simulink model "Supplementary"  (R2021a)
(part 36 of 44)

C12b = 0.125*a4*lc4_1*m4*theta_dot_1*sin(2.0*theta3 - 2.0*theta2 + 2.0*theta4) - 0.125*a4*lc4_1*m4*theta_dot_1*sin(2.0*theta2 + 2.0*theta3 + 2.0*theta4) + 0.5*lc5_1*lc5_3*m5*theta_dot_2*sin(theta3 - theta2 + theta4 + theta5) + 0.25*a1*a3*m3*theta_dot_1*sin(theta2 - theta3) + 0.5*a1*a3*m4*theta_dot_1*sin(theta2 - theta3) + 0.5*a1*a3*m5*theta_dot_1*sin(theta2 - theta3) + 0.25*a2*a3*m3*theta_dot_2*sin(theta2 - theta3) + 0.5*a2*a3*m4*theta_dot_2*sin(theta2 - theta3) + 0.5*a2*a3*m5*theta_dot_2*sin(theta2 - theta3) - 0.25*a4*a5*m5*theta_dot_3*sin(theta2 - theta5) - 0.25*a4*a5*m5*theta_dot_4*sin(theta2 - theta5) - 0.125*a4*a5*m5*theta_dot_5*sin(theta2 - theta5) - 0.125*a5*lc5_2*m5*theta_dot_1*cos(2.0*theta3 - 2.0*theta2 + 2.0*theta4 + 2.0*theta5) + 0.125*a5*lc5_2*m5*theta_dot_1*cos(2.0*theta2 + 2.0*theta3 + 2.0*theta4 + 2.0*theta5) - 0.25*a3*a4*m4*theta_dot_2*cos(2.0*theta3 - theta2 + theta4) + 0.25*a3*a4*m4*theta_dot_3*cos(2.0*theta3 - theta2 + theta4) - 0.5*a3*a4*m5*theta_dot_2*cos(2.0*theta3 - theta2 + theta4) + 0.125*a3*a4*m4*theta_dot_4*cos(2.0*theta3 - theta2 + theta4) + 0.5*a3*a4*m5*theta_dot_3*cos(2.0*theta3 - theta2 + theta4) + 0.25*a3*a4*m5*theta_dot_4*cos(2.0*theta3 - theta2 + theta4) + 0.5*lc3_1*lc3_3*m3*theta_dot_2*cos(theta2 - theta3) + 0.5*a1*lc3_1*m3*theta_dot_1*sin(theta2 - theta3) + 0.5*a2*lc3_1*m3*theta_dot_2*sin(theta2 - theta3) + 0.5*a3*lc4_2*m4*theta_dot_3*sin(theta2 - theta4) + 0.25*a3*lc4_2*m4*theta_dot_4*sin(theta2 - theta4) - 0.5*a4*lc5_1*m5*theta_dot_3*sin(theta2 - theta5) - 0.5*a4*lc5_1*m5*theta_dot_4*sin(theta2 - theta5) - 0.25*a4*lc5_1*m5*theta_dot_5*sin(theta2 - theta5) - 0.25*lc5_1*lc5_2*m5*theta_dot_1*cos(2.0*theta3 - 2.0*theta2 + 2.0*theta4 + 2.0*theta5) + 0.25*lc5_1*lc5_2*m5*theta_dot_1*cos(2.0*theta2 + 2.0*theta3 + 2.0*theta4 + 2.0*theta5) - 0.5*a3*lc4_1*m4*theta_dot_2*cos(2.0*theta3 - theta2 + theta4) + 0.5*a3*lc4_1*m4*theta_dot_3*cos(2.0*theta3 - theta2 + theta4) + 0.25*a3*lc4_1*m4*theta_dot_4*cos(2.0*theta3 - theta2 + theta4) - 0.5*a1*lc4_2*m4*theta_dot_1*cos(theta2 + theta3 + theta4) + 0.5*a2*lc4_2*m4*theta_dot_2*cos(theta2 + theta3 + theta4) + 0.25*a4*lc4_3*m4*theta_dot_2*cos(theta2 + theta3 + theta4) + 0.5*a4*lc5_3*m5*theta_dot_2*cos(theta2 + theta3 + theta4) + 0.5*a3*lc5_2*m5*theta_dot_3*cos(theta2 + theta4 + theta5) + 0.25*a3*lc5_2*m5*theta_dot_4*cos(theta2 + theta4 + theta5) + 0.25*a3*lc5_2*m5*theta_dot_5*cos(theta2 + theta4 + theta5) - 0.125*a5*lc5_1*m5*theta_dot_1*sin(2.0*theta3 - 2.0*theta2 + 2.0*theta4 + 2.0*theta5) + 0.125*a5*lc5_1*m5*theta_dot_1*sin(2.0*theta2 + 2.0*theta3 + 2.0*theta4 + 2.0*theta5) - 0.25*a1*a4*m4*theta_dot_1*sin(theta2 + theta3 + theta4) - 0.5*a1*a4*m5*theta_dot_1*sin(theta2 + theta3 + theta4) + 0.25*a2*a4*m4*theta_dot_2*sin(theta2 + theta3 + theta4) + 0.5*a2*a4*m5*theta_dot_2*sin(theta2 + theta3 + theta4) + 0.25*a3*a5*m5*theta_dot_3*sin(theta2 + theta4 + theta5) + 0.125*a3*a5*m5*theta_dot_4*sin(theta2 + theta4 + theta5) + 0.125*a3*a5*m5*theta_dot_5*sin(theta2 + theta4 + theta5) + 0.5*lc3_2*lc3_3*m3*theta_dot_2*sin(theta2 - theta3) + 0.5*lc4_1*lc4_3*m4*theta_dot_2*cos(theta2 + theta3 + theta4) + 0.5*a3*lc4_2*m4*theta_dot_2*sin(2.0*theta3 - theta2 + theta4) - 0.5*a3*lc4_2*m4*theta_dot_3*sin(2.0*theta3 - theta2 + theta4) - 0.25*a3*lc4_2*m4*theta_dot_4*sin(2.0*theta3 - theta2 + theta4) - 0.5*a1*lc4_1*m4*theta_dot_1*sin(theta2 + theta3 + theta4) + 0.5*a2*lc4_1*m4*theta_dot_2*sin(theta2 + theta3 + theta4) + 0.5*a3*lc5_1*m5*theta_dot_3*sin(theta2 + theta4 + theta5) + 0.25*a3*lc5_1*m5*theta_dot_4*sin(theta2 + theta4 + theta5) + 0.25*a3*lc5_1*m5*theta_dot_5*sin(theta2 + theta4 + theta5) - 0.5*a4*lc5_2*m5*theta_dot_2*cos(2.0*theta3 - theta2 + 2.0*theta4 + theta5) + 0.5*a4*lc5_2*m5*theta_dot_3*cos(2.0*theta3 - theta2 + 2.0*theta4 + theta5) + 0.5*a4*lc5_2*m5*theta_dot_4*cos(2.0*theta3 - theta2 + 2.0*theta4 + theta5) + 0.25*a4*lc5_2*m5*theta_dot_5*cos(2.0*theta3 - theta2 + 2.0*theta4 + theta5) - 0.5*a2*lc5_2*m5*theta_dot_1*cos(theta3 - 2.0*theta2 + theta4 + theta5) + 0.5*a2*lc5_2*m5*theta_dot_1*cos(2.0*theta2 + theta3 + theta4 + theta5) + 0.5*a3*lc5_2*m5*theta_dot_2*cos(theta2 + 2.0*theta3 + theta4 + theta5) + 0.5*a3*lc5_2*m5*theta_dot_3*cos(theta2 + 2.0*theta3 + theta4 + theta5) + 0.25*a3*lc5_2*m5*theta_dot_4*cos(theta2 + 2.0*theta3 + theta4 + theta5) + 0.25*a5*lc5_3*m5*theta_dot_1*cos(theta3 - 2.0*theta2 + theta4 + theta5) + 0.25*a5*lc5_3*m5*theta_dot_1*cos(2.0*theta2 + theta3 + theta4 + theta5) + 0.25*a3*lc5_2*m5*theta_dot_5*cos(theta2 + 2.0*theta3 + theta4 + theta5) - 0.25*a4*a5*m5*theta_dot_2*sin(2.0*theta3 - theta2 + 2.0*theta4 + theta5) + 0.25*a4*a5*m5*theta_dot_3*sin(2.0*theta3 - theta2 + 2.0*theta4 + theta5) + 0.25*a4*a5*m5*theta_dot_4*sin(2.0*theta3 - theta2 + 2.0*theta4 + theta5) + 0.125*a4*a5*m5*theta_dot_5*sin(2.0*theta3 - theta2 + 2.0*theta4 + theta5) - 0.25*a2*a5*m5*theta_dot_1*sin(theta3 - 2.0*theta2 + theta4 + theta5) + 0.25*a2*a5*m5*theta_dot_1*sin(2.0*theta2 + theta3 + theta4 + theta5) + 0.25*a3*a5*m5*theta_dot_2*sin(theta2 + 2.0*theta3 + theta4 + theta5) + 0.25*a3*a5*m5*theta_dot_3*sin(theta2 + 2.0*theta3 + theta4 + theta5) + 0.125*a3*a5*m5*theta_dot_4*sin(theta2 + 2.0*theta3 + theta4 + theta5) + 0.125*a3*a5*m5*theta_dot_5*sin(theta2 + 2.0*theta3 + theta4 + theta5) - 0.5*lc4_2*lc4_3*m4*theta_dot_2*sin(theta2 + theta3 + theta4) + 0.5*lc5_1*lc5_3*m5*theta_dot_1*cos(theta3 - 2.0*theta2 + theta4 + theta5) + 0.5*lc5_1*lc5_3*m5*theta_dot_1*cos(2.0*theta2 + theta3 + theta4 + theta5) + 0.25*a2*a3*m3*theta_dot_1*cos(2.0*theta2 + theta3) + 0.5*a2*a3*m4*theta_dot_1*cos(2.0*theta2 + theta3) + 0.5*a2*a3*m5*theta_dot_1*cos(2.0*theta2 + theta3) - 0.125*a4*a5*m5*theta_dot_1*cos(2.0*theta2 + theta5) - 0.5*a4*lc5_1*m5*theta_dot_2*sin(2.0*theta3 - theta2 + 2.0*theta4 + theta5) + 0.5*a4*lc5_1*m5*theta_dot_3*sin(2.0*theta3 - theta2 + 2.0*theta4 + theta5) + 0.5*a4*lc5_1*m5*theta_dot_4*sin(2.0*theta3 - theta2 + 2.0*theta4 + theta5) + 0.25*a4*lc5_1*m5*theta_dot_5*sin(2.0*theta3 - theta2 + 2.0*theta4 + theta5) - 0.5*a2*lc5_1*m5*theta_dot_1*sin(theta3 - 2.0*theta2 + theta4 + theta5) + 0.5*a2*lc5_1*m5*theta_dot_1*sin(2.0*theta2 + theta3 + theta4 + theta5) + 0.5*a3*lc5_1*m5*theta_dot_2*sin(theta2 + 2.0*theta3 + theta4 + theta5) + 0.5*a3*lc5_1*m5*theta_dot_3*sin(theta2 + 2.0*theta3 + theta4 + theta5) + 0.25*a3*lc5_1*m5*theta_dot_4*sin(theta2 + 2.0*theta3 + theta4 + theta5) + 0.25*a3*lc5_1*m5*theta_dot_5*sin(theta2 + 2.0*theta3 + theta4 + theta5) + 0.5*a2*lc3_1*m3*theta_dot_1*cos(2.0*theta2 + theta3) - 0.25*a3*lc3_1*m3*theta_dot_2*cos(theta2 - 2.0*theta3) + 0.25*a3*lc3_1*m3*theta_dot_2*cos(theta2 + 2.0*theta3) + 0.25*a3*lc3_1*m3*theta_dot_3*cos(theta2 - 2.0*theta3) + 0.25*a3*lc3_1*m3*theta_dot_3*cos(theta2 + 2.0*theta3) + 0.25*a3*lc4_2*m4*theta_dot_1*cos(2.0*theta2 + theta4) - 0.25*a4*lc5_1*m5*theta_dot_1*cos(2.0*theta2 + theta5) - 0.5*lc5_2*lc5_3*m5*theta_dot_1*sin(theta3 - 2.0*theta2 + theta4 + theta5) - 0.5*lc5_2*lc5_3*m5*theta_dot_1*sin(2.0*theta2 + theta3 + theta4 + theta5) + 0.125*a3*a4*m4*theta_dot_1*sin(2.0*theta2 + theta4) + 0.25*a3*a4*m5*theta_dot_1*sin(2.0*theta2 + theta4) - 0.5*lc3_2*lc3_3*m3*theta_dot_1*cos(2.0*theta2 + theta3) - 0.5*a2*lc3_2*m3*theta_dot_1*sin(2.0*theta2 + theta3) - 0.25*a3*lc3_2*m3*theta_dot_2*sin(theta2 - 2.0*theta3) - 0.25*a3*lc3_2*m3*theta_dot_2*sin(theta2 + 2.0*theta3) - 0.25*a3*lc3_3*m3*theta_dot_1*sin(2.0*theta2 + theta3) + 0.25*a3*lc3_2*m3*theta_dot_3*sin(theta2 - 2.0*theta3) - 0.25*a3*lc3_2*m3*theta_dot_3*sin(theta2 + 2.0*theta3) + 0.25*a3*lc4_1*m4*theta_dot_1*sin(2.0*theta2 + theta4) - 0.5*a3*lc4_3*m4*theta_dot_1*sin(2.0*theta2 + theta3) - 0.5*a3*lc5_3*m5*theta_dot_1*sin(2.0*theta2 + theta3) + 0.25*a4*lc5_2*m5*theta_dot_1*sin(2.0*theta2 + theta5) + 0.25*a3*lc4_2*m4*theta_dot_1*cos(2.0*theta3 - 2.0*theta2 + theta4) - 0.25*a3*lc4_2*m4*theta_dot_1*cos(2.0*theta2 + 2.0*theta3 + theta4) + 0.25*a4*lc4_1*m4*theta_dot_2*cos(theta2 + 2.0*theta3 + 2.0*theta4) + 0.25*a4*lc4_1*m4*theta_dot_3*cos(theta2 + 2.0*theta3 + 2.0*theta4) + 0.25*a4*lc4_1*m4*theta_dot_4*cos(theta2 + 2.0*theta3 + 2.0*theta4) + 0.125*a3*a4*m4*theta_dot_1*sin(2.0*theta3 - 2.0*theta2 + theta4) - 0.125*a3*a4*m4*theta_dot_1*sin(2.0*theta2 + 2.0*theta3 + theta4) + 0.25*a3*a4*m5*theta_dot_1*sin(2.0*theta3 - 2.0*theta2 + theta4) - 0.25*a3*a4*m5*theta_dot_1*sin(2.0*theta2 + 2.0*theta3 + theta4) - 0.5*lc3_1*lc3_2*m3*theta_dot_2*sin(theta2 - 2.0*theta3) - 0.5*lc3_1*lc3_2*m3*theta_dot_2*sin(theta2 + 2.0*theta3) - 0.5*lc3_1*lc3_3*m3*theta_dot_1*sin(2.0*theta2 + theta3) + 0.5*lc3_1*lc3_2*m3*theta_dot_3*sin(theta2 - 2.0*theta3) - 0.5*lc3_1*lc3_2*m3*theta_dot_3*sin(theta2 + 2.0*theta3) - 0.125*a4*a5*m5*theta_dot_1*cos(2.0*theta3 - 2.0*theta2 + 2.0*theta4 + theta5) + 0.125*a4*a5*m5*theta_dot_1*cos(2.0*theta2 + 2.0*theta3 + 2.0*theta4 + theta5) + 0.25*a3*lc4_1*m4*theta_dot_1*sin(2.0*theta3 - 2.0*theta2 + theta4) - 0.25*a3*lc4_1*m4*theta_dot_1*sin(2.0*theta2 + 2.0*theta3 + theta4) - 0.25*a4*lc4_2*m4*theta_dot_2*sin(theta2 + 2.0*theta3 + 2.0*theta4) - 0.25*a4*lc4_2*m4*theta_dot_3*sin(theta2 + 2.0*theta3 + 2.0*theta4) - 0.25*a4*lc4_2*m4*theta_dot_4*sin(theta2 + 2.0*theta3 + 2.0*theta4) - 0.25*a4*lc5_1*m5*theta_dot_1*cos(2.0*theta3 - 2.0*theta2 + 2.0*theta4 + theta5) + 0.25*a4*lc5_1*m5*theta_dot_1*cos(2.0*theta2 + 2.0*theta3 + 2.0*theta4 + theta5) - 0.25*a5*lc5_1*m5*theta_dot_2*cos(theta2 + 2.0*theta3 + 2.0*theta4 + 2.0*theta5) - 0.25*a5*lc5_1*m5*theta_dot_3*cos(theta2 + 2.0*theta3 + 2.0*theta4 + 2.0*theta5) - 0.25*a5*lc5_1*m5*theta_dot_4*cos(theta2 + 2.0*theta3 + 2.0*theta4 + 2.0*theta5) - 0.25*a5*lc5_1*m5*theta_dot_5*cos(theta2 + 2.0*theta3 + 2.0*theta4 + 2.0*theta5) + 0.5*a2*lc2_3*m2*theta_dot_1*cos(2.0*theta2) + 1.0*a2*lc3_3*m3*theta_dot_1*cos(2.0*theta2) + 1.0*a2*lc4_3*m4*theta_dot_1*cos(2.0*theta2) + 1.0*a2*lc5_3*m5*theta_dot_1*cos(2.0*theta2) - 0.5*lc4_1*lc4_2*m4*theta_dot_2*sin(theta2 + 2.0*theta3 + 2.0*theta4) - 0.5*lc4_1*lc4_2*m4*theta_dot_3*sin(theta2 + 2.0*theta3 + 2.0*theta4) - 0.5*lc4_1*lc4_2*m4*theta_dot_4*sin(theta2 + 2.0*theta3 + 2.0*theta4) - 0.5*a1*lc4_2*m4*theta_dot_1*cos(theta3 - theta2 + theta4) - 0.5*a2*lc4_2*m4*theta_dot_2*cos(theta3 - theta2 + theta4) + 0.25*a4*lc4_3*m4*theta_dot_2*cos(theta3 - theta2 + theta4) + 0.5*a4*lc5_3*m5*theta_dot_2*cos(theta3 - theta2 + theta4) + 0.5*a3*lc5_2*m5*theta_dot_3*cos(theta4 - theta2 + theta5) + 0.25*a3*lc5_2*m5*theta_dot_4*cos(theta4 - theta2 + theta5) + 0.25*a3*lc5_2*m5*theta_dot_5*cos(theta4 - theta2 + theta5) + 1.0*lc2_1*lc2_3*m2*theta_dot_1*cos(2.0*theta2) + 0.25*a4*lc5_2*m5*theta_dot_1*sin(2.0*theta3 - 2.0*theta2 + 2.0*theta4 + theta5) - 0.25*a4*lc5_2*m5*theta_dot_1*sin(2.0*theta2 + 2.0*theta3 + 2.0*theta4 + theta5) + 0.25*a5*lc5_2*m5*theta_dot_2*sin(theta2 + 2.0*theta3 + 2.0*theta4 + 2.0*theta5) + 0.25*a5*lc5_2*m5*theta_dot_3*sin(theta2 + 2.0*theta3 + 2.0*theta4 + 2.0*theta5) + 0.25*a5*lc5_2*m5*theta_dot_4*sin(theta2 + 2.0*theta3 + 2.0*theta4 + 2.0*theta5) + 0.25*a5*lc5_2*m5*theta_dot_5*sin(theta2 + 2.0*theta3 + 2.0*theta4 + 2.0*theta5) - 0.25*a1*a4*m4*theta_dot_1*sin(theta3 - theta2 + theta4) - 0.5*a1*a4*m5*theta_dot_1*sin(theta3 - theta2 + theta4) - 0.25*a2*a4*m4*theta_dot_2*sin(theta3 - theta2 + theta4) - 0.5*a2*a4*m5*theta_dot_2*sin(theta3 - theta2 + theta4) + 0.25*a3*a5*m5*theta_dot_3*sin(theta4 - theta2 + theta5) + 0.125*a3*a5*m5*theta_dot_4*sin(theta4 - theta2 + theta5) + 0.125*a3*a5*m5*theta_dot_5*sin(theta4 - theta2 + theta5) + 0.5*a2*lc2_1*m2*theta_dot_1*sin(2.0*theta2) + 0.25*a3*lc3_1*m3*theta_dot_1*sin(2.0*theta2) + 0.25*a4*lc4_1*m4*theta_dot_1*sin(2.0*theta2) + 0.25*a5*lc5_1*m5*theta_dot_1*sin(2.0*theta2) + 0.25*a1*a5*m5*theta_dot_1*cos(theta2 + theta3 + theta4 + theta5) - 0.25*a2*a5*m5*theta_dot_2*cos(theta2 + theta3 + theta4 + theta5) + 0.5*lc4_1*lc4_3*m4*theta_dot_2*cos(theta3 - theta2 + theta4) + 0.5*lc5_1*lc5_2*m5*theta_dot_2*sin(theta2 + 2.0*theta3 + 2.0*theta4 + 2.0*theta5) + 0.5*lc5_1*lc5_2*m5*theta_dot_3*sin(theta2 + 2.0*theta3 + 2.0*theta4 + 2.0*theta5) + 0.5*lc5_1*lc5_2*m5*theta_dot_4*sin(theta2 + 2.0*theta3 + 2.0*theta4 + 2.0*theta5) + 0.5*lc5_1*lc5_2*m5*theta_dot_5*sin(theta2 + 2.0*theta3 + 2.0*theta4 + 2.0*theta5) - 0.5*a1*lc4_1*m4*theta_dot_1*sin(theta3 - theta2 + theta4) - 0.5*a2*lc4_1*m4*theta_dot_2*sin(theta3 - theta2 + theta4) + 0.5*a3*lc5_1*m5*theta_dot_3*sin(theta4 - theta2 + theta5) + 0.25*a3*lc5_1*m5*theta_dot_4*sin(theta4 - theta2 + theta5) + 0.25*a3*lc5_1*m5*theta_dot_5*sin(theta4 - theta2 + theta5) - 0.5*a3*lc5_2*m5*theta_dot_2*cos(2.0*theta3 - theta2 + theta4 + theta5) + 0.5*a3*lc5_2*m5*theta_dot_3*cos(2.0*theta3 - theta2 + theta4 + theta5) + 0.25*a3*lc5_2*m5*theta_dot_4*cos(2.0*theta3 - theta2 + theta4 + theta5) + 0.25*a3*lc5_2*m5*theta_dot_5*cos(2.0*theta3 - theta2 + theta4 + theta5) + 0.5*a1*lc5_1*m5*theta_dot_1*cos(theta2 + theta3 + theta4 + theta5) - 0.5*a2*lc5_1*m5*theta_dot_2*cos(theta2 + theta3 + theta4 + theta5) - 0.25*a3*a5*m5*theta_dot_2*sin(2.0*theta3 - theta2 + theta4 + theta5) + 0.25*a3*a5*m5*theta_dot_3*sin(2.0*theta3 - theta2 + theta4 + theta5) + 0.125*a3*a5*m5*theta_dot_4*sin(2.0*theta3 - theta2 + theta4 + theta5) + 0.125*a3*a5*m5*theta_dot_5*sin(2.0*theta3 - theta2 + theta4 + theta5) - 0.5*lc4_2*lc4_3*m4*theta_dot_2*sin(theta3 - theta2 + theta4) - 0.25*a2*a3*m3*theta_dot_1*cos(2.0*theta2 - theta3) - 0.5*a2*a3*m4*theta_dot_1*cos(2.0*theta2 - theta3) - 0.5*a2*a3*m5*theta_dot_1*cos(2.0*theta2 - theta3) + 0.125*a4*a5*m5*theta_dot_1*cos(2.0*theta2 - theta5) + 0.5*lc5_2*lc5_3*m5*theta_dot_2*cos(theta2 + theta3 + theta4 + theta5) + 0.25*a3*a4*m4*theta_dot_3*cos(theta2 + theta4) + 0.125*a3*a4*m4*theta_dot_4*cos(theta2 + theta4) + 0.5*a3*a4*m5*theta_dot_3*cos(theta2 + theta4) + 0.25*a3*a4*m5*theta_dot_4*cos(theta2 + theta4) - 0.5*a3*lc5_1*m5*theta_dot_2*sin(2.0*theta3 - theta2 + theta4 + theta5) + 0.5*a3*lc5_1*m5*theta_dot_3*sin(2.0*theta3 - theta2 + theta4 + theta5) + 0.25*a3*lc5_1*m5*theta_dot_4*sin(2.0*theta3 - theta2 + theta4 + theta5) + 0.25*a3*lc5_1*m5*theta_dot_5*sin(2.0*theta3 - theta2 + theta4 + theta5) - 0.5*a1*lc5_2*m5*theta_dot_1*sin(theta2 + theta3 + theta4 + theta5) + 0.5*a2*lc5_2*m5*theta_dot_2*sin(theta2 + theta3 + theta4 + theta5) + 0.25*a5*lc5_3*m5*theta_dot_2*sin(theta2 + theta3 + theta4 + theta5) - 0.5*a2*lc3_1*m3*theta_dot_1*cos(2.0*theta2 - theta3) - 0.25*a3*lc4_2*m4*theta_dot_1*cos(2.0*theta2 - theta4) + 0.25*a4*lc5_1*m5*theta_dot_1*cos(2.0*theta2 - theta5) - 0.5*a1*lc3_2*m3*theta_dot_1*cos(theta2 + theta3) + 0.5*a2*lc3_2*m3*theta_dot_2*cos(theta2 + theta3) + 0.25*a3*lc3_3*m3*theta_dot_2*cos(theta2 + theta3) + 0.5*a3*lc4_1*m4*theta_dot_3*cos(theta2 + theta4) + 0.5*a3*lc4_3*m4*theta_dot_2*cos(theta2 + theta3) + 0.25*a3*lc4_1*m4*theta_dot_4*cos(theta2 + theta4) + 0.5*a3*lc5_3*m5*theta_dot_2*cos(theta2 + theta3) + 0.5*a4*lc5_2*m5*theta_dot_3*cos(theta2 + theta5) + 0.5*a4*lc5_2*m5*theta_dot_4*cos(theta2 + theta5) + 0.25*a4*lc5_2*m5*theta_dot_5*cos(theta2 + theta5) + 0.125*a3*a4*m4*theta_dot_1*sin(2.0*theta2 - theta4) + 0.25*a3*a4*m5*theta_dot_1*sin(2.0*theta2 - theta4) + 0.5*lc5_1*lc5_3*m5*theta_dot_2*sin(theta2 + theta3 + theta4 + theta5) - 0.25*a1*a3*m3*theta_dot_1*sin(theta2 + theta3) - 0.5*a1*a3*m4*theta_dot_1*sin(theta2 + theta3) - 0.5*a1*a3*m5*theta_dot_1*sin(theta2 + theta3) + 0.25*a2*a3*m3*theta_dot_2*sin(theta2 + theta3) + 0.5*a2*a3*m4*theta_dot_2*sin(theta2 + theta3) + 0.5*a2*a3*m5*theta_dot_2*sin(theta2 + theta3) + 0.25*a4*a5*m5*theta_dot_3*sin(theta2 + theta5) + 0.25*a4*a5*m5*theta_dot_4*sin(theta2 + theta5) + 0.125*a4*a5*m5*theta_dot_5*sin(theta2 + theta5) - 0.25*a2*a4*m4*theta_dot_1*cos(theta3 - 2.0*theta2 + theta4) + 0.25*a2*a4*m4*theta_dot_1*cos(2.0*theta2 + theta3 + theta4) - 0.5*a2*a4*m5*theta_dot_1*cos(theta3 - 2.0*theta2 + theta4) + 0.5*a2*a4*m5*theta_dot_1*cos(2.0*theta2 + theta3 + theta4) + 0.25*a3*a4*m4*theta_dot_2*cos(theta2 + 2.0*theta3 + theta4) + 0.25*a3*a4*m4*theta_dot_3*cos(theta2 + 2.0*theta3 + theta4) + 0.5*a3*a4*m5*theta_dot_2*cos(theta2 + 2.0*theta3 + theta4) + 0.125*a3*a4*m4*theta_dot_4*cos(theta2 + 2.0*theta3 + theta4) + 0.5*a3*a4*m5*theta_dot_3*cos(theta2 + 2.0*theta3 + theta4) + 0.25*a3*a4*m5*theta_dot_4*cos(theta2 + 2.0*theta3 + theta4) + 0.125*a3*a5*m5*theta_dot_1*cos(theta4 - 2.0*theta2 + theta5) - 0.125*a3*a5*m5*theta_dot_1*cos(2.0*theta2 + theta4 + theta5) - 0.5*lc3_2*lc3_3*m3*theta_dot_1*cos(2.0*theta2 - theta3) + 0.5*lc3_1*lc3_3*m3*theta_dot_2*cos(theta2 + theta3) - 0.5*a2*lc3_2*m3*theta_dot_1*sin(2.0*theta2 - theta3) + 0.25*a3*lc3_3*m3*theta_dot_1*sin(2.0*theta2 - theta3) + 0.25*a3*lc4_1*m4*theta_dot_1*sin(2.0*theta2 - theta4) + 0.5*a3*lc4_3*m4*theta_dot_1*sin(2.0*theta2 - theta3) + 0.5*a3*lc5_3*m5*theta_dot_1*sin(2.0*theta2 - theta3) + 0.25*a4*lc5_2*m5*theta_dot_1*sin(2.0*theta2 - theta5) - 0.5*a1*lc3_1*m3*theta_dot_1*sin(theta2 + theta3) + 0.5*a2*lc3_1*m3*theta_dot_2*sin(theta2 + theta3) - 0.5*a3*lc4_2*m4*theta_dot_3*sin(theta2 + theta4) - 0.25*a3*lc4_2*m4*theta_dot_4*sin(theta2 + theta4) + 0.5*a4*lc5_1*m5*theta_dot_3*sin(theta2 + theta5) + 0.5*a4*lc5_1*m5*theta_dot_4*sin(theta2 + theta5) + 0.25*a4*lc5_1*m5*theta_dot_5*sin(theta2 + theta5) - 0.25*a4*lc4_1*m4*theta_dot_2*cos(2.0*theta3 - theta2 + 2.0*theta4) + 0.25*a4*lc4_1*m4*theta_dot_3*cos(2.0*theta3 - theta2 + 2.0*theta4) + 0.25*a4*lc4_1*m4*theta_dot_4*cos(2.0*theta3 - theta2 + 2.0*theta4) - 0.5*a2*lc4_1*m4*theta_dot_1*cos(theta3 - 2.0*theta2 + theta4) + 0.5*a2*lc4_1*m4*theta_dot_1*cos(2.0*theta2 + theta3 + theta4) + 0.5*a3*lc4_1*m4*theta_dot_2*cos(theta2 + 2.0*theta3 + theta4) + 0.5*a3*lc4_1*m4*theta_dot_3*cos(theta2 + 2.0*theta3 + theta4) + 0.25*a3*lc4_1*m4*theta_dot_4*cos(theta2 + 2.0*theta3 + theta4) + 0.25*a3*lc5_1*m5*theta_dot_1*cos(theta4 - 2.0*theta2 + theta5) - 0.25*a3*lc5_1*m5*theta_dot_1*cos(2.0*theta2 + theta4 + theta5) + 0.5*lc3_1*lc3_3*m3*theta_dot_1*sin(2.0*theta2 - theta3) - 0.5*lc3_2*lc3_3*m3*theta_dot_2*sin(theta2 + theta3) - 0.125*a3*a5*m5*theta_dot_1*cos(2.0*theta3 - 2.0*theta2 + theta4 + theta5) + 0.125*a3*a5*m5*theta_dot_1*cos(2.0*theta2 + 2.0*theta3 + theta4 + theta5) - 0.5*lc4_2*lc4_3*m4*theta_dot_1*cos(theta3 - 2.0*theta2 + theta4) - 0.5*lc4_2*lc4_3*m4*theta_dot_1*cos(2.0*theta2 + theta3 + theta4) + 0.5*a1*a2*m2*theta_dot_1*cos(theta2) + 1.0*a1*a2*m3*theta_dot_1*cos(theta2) + 1.0*a1*a2*m4*theta_dot_1*cos(theta2) + 1.0*a1*a2*m5*theta_dot_1*cos(theta2) + 0.25*a4*lc4_2*m4*theta_dot_2*sin(2.0*theta3 - theta2 + 2.0*theta4) - 0.25*a4*lc4_2*m4*theta_dot_3*sin(2.0*theta3 - theta2 + 2.0*theta4) - 0.25*a4*lc4_2*m4*theta_dot_4*sin(2.0*theta3 - theta2 + 2.0*theta4) + 0.5*a2*lc4_2*m4*theta_dot_1*sin(theta3 - 2.0*theta2 + theta4) - 0.5*a2*lc4_2*m4*theta_dot_1*sin(2.0*theta2 + theta3 + theta4) - 0.5*a3*lc4_2*m4*theta_dot_2*sin(theta2 + 2.0*theta3 + theta4) - 0.5*a3*lc4_2*m4*theta_dot_3*sin(theta2 + 2.0*theta3 + theta4) - 0.25*a4*lc4_3*m4*theta_dot_1*sin(theta3 - 2.0*theta2 + theta4) - 0.25*a4*lc4_3*m4*theta_dot_1*sin(2.0*theta2 + theta3 + theta4) - 0.25*a3*lc4_2*m4*theta_dot_4*sin(theta2 + 2.0*theta3 + theta4) - 0.25*a3*lc5_2*m5*theta_dot_1*sin(theta4 - 2.0*theta2 + theta5) + 0.25*a3*lc5_2*m5*theta_dot_1*sin(2.0*theta2 + theta4 + theta5) - 0.5*a4*lc5_3*m5*theta_dot_1*sin(theta3 - 2.0*theta2 + theta4) - 0.5*a4*lc5_3*m5*theta_dot_1*sin(2.0*theta2 + theta3 + theta4) + 0.25*a5*lc5_1*m5*theta_dot_2*cos(2.0*theta3 - theta2 + 2.0*theta4 + 2.0*theta5) - 0.25*a5*lc5_1*m5*theta_dot_3*cos(2.0*theta3 - theta2 + 2.0*theta4 + 2.0*theta5) - 0.25*a5*lc5_1*m5*theta_dot_4*cos(2.0*theta3 - theta2 + 2.0*theta4 + 2.0*theta5) - 0.25*a5*lc5_1*m5*theta_dot_5*cos(2.0*theta3 - theta2 + 2.0*theta4 + 2.0*theta5) - 0.25*a3*lc5_1*m5*theta_dot_1*cos(2.0*theta3 - 2.0*theta2 + theta4 + theta5) + 0.25*a3*lc5_1*m5*theta_dot_1*cos(2.0*theta2 + 2.0*theta3 + theta4 + theta5) + 0.5*a4*lc5_2*m5*theta_dot_2*cos(theta2 + 2.0*theta3 + 2.0*theta4 + theta5) + 0.5*a4*lc5_2*m5*theta_dot_3*cos(theta2 + 2.0*theta3 + 2.0*theta4 + theta5) + 0.5*a4*lc5_2*m5*theta_dot_4*cos(theta2 + 2.0*theta3 + 2.0*theta4 + theta5) + 0.25*a4*lc5_2*m5*theta_dot_5*cos(theta2 + 2.0*theta3 + 2.0*theta4 + theta5) + 1.0*a1*lc2_1*m2*theta_dot_1*cos(theta2) + 0.5*a3*lc3_1*m3*theta_dot_3*cos(theta2) + 0.5*a4*lc4_1*m4*theta_dot_3*cos(theta2) + 0.5*a4*lc4_1*m4*theta_dot_4*cos(theta2) + 0.5*a5*lc5_1*m5*theta_dot_3*cos(theta2) + 0.5*a5*lc5_1*m5*theta_dot_4*cos(theta2) + 0.5*a5*lc5_1*m5*theta_dot_5*cos(theta2) + 0.25*a4*a5*m5*theta_dot_2*sin(theta2 + 2.0*theta3 + 2.0*theta4 + theta5) + 0.25*a4*a5*m5*theta_dot_3*sin(theta2 + 2.0*theta3 + 2.0*theta4 + theta5) + 0.25*a4*a5*m5*theta_dot_4*sin(theta2 + 2.0*theta3 + 2.0*theta4 + theta5) + 0.125*a4*a5*m5*theta_dot_5*sin(theta2 + 2.0*theta3 + 2.0*theta4 + theta5) + 0.5*lc4_1*lc4_2*m4*theta_dot_2*sin(2.0*theta3 - theta2 + 2.0*theta4) - 0.5*lc4_1*lc4_2*m4*theta_dot_3*sin(2.0*theta3 - theta2 + 2.0*theta4) - 0.5*lc4_1*lc4_2*m4*theta_dot_4*sin(2.0*theta3 - theta2 + 2.0*theta4) - 0.5*lc4_1*lc4_3*m4*theta_dot_1*sin(theta3 - 2.0*theta2 + theta4) - 0.5*lc4_1*lc4_3*m4*theta_dot_1*sin(2.0*theta2 + theta3 + theta4) - 0.25*a5*lc5_2*m5*theta_dot_2*sin(2.0*theta3 - theta2 + 2.0*theta4 + 2.0*theta5) + 0.25*a5*lc5_2*m5*theta_dot_3*sin(2.0*theta3 - theta2 + 2.0*theta4 + 2.0*theta5) + 0.25*a5*lc5_2*m5*theta_dot_4*sin(2.0*theta3 - theta2 + 2.0*theta4 + 2.0*theta5) + 0.25*a5*lc5_2*m5*theta_dot_5*sin(2.0*theta3 - theta2 + 2.0*theta4 + 2.0*theta5) + 1.0*lc2_2*lc2_3*m2*theta_dot_2*cos(theta2) + 0.25*a3*lc5_2*m5*theta_dot_1*sin(2.0*theta3 - 2.0*theta2 + theta4 + theta5) - 0.25*a3*lc5_2*m5*theta_dot_1*sin(2.0*theta2 + 2.0*theta3 + theta4 + theta5) + 0.5*a4*lc5_1*m5*theta_dot_2*sin(theta2 + 2.0*theta3 + 2.0*theta4 + theta5) + 0.5*a4*lc5_1*m5*theta_dot_3*sin(theta2 + 2.0*theta3 + 2.0*theta4 + theta5) + 0.5*a4*lc5_1*m5*theta_dot_4*sin(theta2 + 2.0*theta3 + 2.0*theta4 + theta5) + 0.25*a4*lc5_1*m5*theta_dot_5*sin(theta2 + 2.0*theta3 + 2.0*theta4 + theta5) - 1.0*a1*lc2_3*m2*theta_dot_1*sin(theta2) + 0.5*a2*lc2_2*m2*theta_dot_2*sin(theta2) - 1.0*a1*lc3_3*m3*theta_dot_1*sin(theta2) - 1.0*a1*lc4_3*m4*theta_dot_1*sin(theta2) - 1.0*a1*lc5_3*m5*theta_dot_1*sin(theta2) + 0.25*a1*a5*m5*theta_dot_1*cos(theta3 - theta2 + theta4 + theta5) + 0.25*a2*a5*m5*theta_dot_2*cos(theta3 - theta2 + theta4 + theta5) + 0.125*a3*lc3_2*m3*theta_dot_1*cos(2.0*theta2 - 2.0*theta3) - 0.125*a3*lc3_2*m3*theta_dot_1*cos(2.0*theta2 + 2.0*theta3) - 0.5*lc5_1*lc5_2*m5*theta_dot_2*sin(2.0*theta3 - theta2 + 2.0*theta4 + 2.0*theta5) + 0.5*lc5_1*lc5_2*m5*theta_dot_3*sin(2.0*theta3 - theta2 + 2.0*theta4 + 2.0*theta5) + 0.5*lc5_1*lc5_2*m5*theta_dot_4*sin(2.0*theta3 - theta2 + 2.0*theta4 + 2.0*theta5) + 0.5*lc5_1*lc5_2*m5*theta_dot_5*sin(2.0*theta3 - theta2 + 2.0*theta4 + 2.0*theta5)
C12 = C12a + C12b
C13a = 0.25*I_xy_3*theta_dot_1*cos(2.0*theta2 - 2.0*theta3) + 0.25*I_xy_3*theta_dot_1*cos(2.0*theta2 + 2.0*theta3) + 0.5*I_xy_4*theta_dot_1*cos(2.0*theta3 + 2.0*theta4) + 0.5*I_yz_5*theta_dot_3*cos(theta3 - theta2 + theta4 + theta5) + 0.5*I_yz_5*theta_dot_4*cos(theta3 - theta2 + theta4 + theta5) + 0.5*I_yz_5*theta_dot_5*cos(theta3 - theta2 + theta4 + theta5) - 0.125*I_xx_3*theta_dot_1*sin(2.0*theta2 - 2.0*theta3) + 0.125*I_xx_3*theta_dot_1*sin(2.0*theta2 + 2.0*theta3) + 0.25*I_xx_4*theta_dot_1*sin(2.0*theta3 + 2.0*theta4) + 0.125*I_yy_3*theta_dot_1*sin(2.0*theta2 - 2.0*theta3) - 0.125*I_yy_3*theta_dot_1*sin(2.0*theta2 + 2.0*theta3) - 0.25*I_yy_4*theta_dot_1*sin(2.0*theta3 + 2.0*theta4) + 0.25*I_xy_4*theta_dot_1*cos(2.0*theta3 - 2.0*theta2 + 2.0*theta4) + 0.25*I_xy_4*theta_dot_1*cos(2.0*theta2 + 2.0*theta3 + 2.0*theta4) - 0.5*I_xy_5*theta_dot_1*cos(2.0*theta3 + 2.0*theta4 + 2.0*theta5) + 0.5*I_xz_5*theta_dot_3*sin(theta3 - theta2 + theta4 + theta5) + 0.5*I_xz_5*theta_dot_4*sin(theta3 - theta2 + theta4 + theta5) + 0.5*I_xz_5*theta_dot_5*sin(theta3 - theta2 + theta4 + theta5) + 0.5*I_xz_3*theta_dot_3*cos(theta2 - theta3) + 0.125*I_xx_4*theta_dot_1*sin(2.0*theta3 - 2.0*theta2 + 2.0*theta4) + 0.125*I_xx_4*theta_dot_1*sin(2.0*theta2 + 2.0*theta3 + 2.0*theta4) - 0.25*I_xx_5*theta_dot_1*sin(2.0*theta3 + 2.0*theta4 + 2.0*theta5) - 0.125*I_yy_4*theta_dot_1*sin(2.0*theta3 - 2.0*theta2 + 2.0*theta4) - 0.125*I_yy_4*theta_dot_1*sin(2.0*theta2 + 2.0*theta3 + 2.0*theta4) + 0.25*I_yy_5*theta_dot_1*sin(2.0*theta3 + 2.0*theta4 + 2.0*theta5) - 0.25*I_xy_5*theta_dot_1*cos(2.0*theta3 - 2.0*theta2 + 2.0*theta4 + 2.0*theta5) - 0.25*I_xy_5*theta_dot_1*cos(2.0*theta2 + 2.0*theta3 + 2.0*theta4 + 2.0*theta5) + 0.5*I_yz_3*theta_dot_3*sin(theta2 - theta3) + 0.5*I_xz_4*theta_dot_3*cos(theta2 + theta3 + theta4) + 0.5*I_xz_4*theta_dot_4*cos(theta2 + theta3 + theta4) - 0.125*I_xx_5*theta_dot_1*sin(2.0*theta3 - 2.0*theta2 + 2.0*theta4 + 2.0*theta5) - 0.125*I_xx_5*theta_dot_1*sin(2.0*theta2 + 2.0*theta3 + 2.0*theta4 + 2.0*theta5) + 0.125*I_yy_5*theta_dot_1*sin(2.0*theta3 - 2.0*theta2 + 2.0*theta4 + 2.0*theta5) + 0.125*I_yy_5*theta_dot_1*sin(2.0*theta2 + 2.0*theta3 + 2.0*theta4 + 2.0*theta5) - 0.5*I_yz_4*theta_dot_3*sin(theta2 + theta3 + theta4) - 0.5*I_yz_4*theta_dot_4*sin(theta2 + theta3 + theta4) + 0.25*I_xz_5*theta_dot_1*cos(theta3 - 2.0*theta2 + theta4 + theta5) - 0.25*I_xz_5*theta_dot_1*cos(2.0*theta2 + theta3 + theta4 + theta5) - 0.25*I_yz_5*theta_dot_1*sin(theta3 - 2.0*theta2 + theta4 + theta5) + 0.25*I_yz_5*theta_dot_1*sin(2.0*theta2 + theta3 + theta4 + theta5) - 0.25*I_xx_3*theta_dot_2*cos(theta2 - 2.0*theta3) - 0.25*I_xx_3*theta_dot_2*cos(theta2 + 2.0*theta3) + 0.25*I_yy_3*theta_dot_2*cos(theta2 - 2.0*theta3) + 0.25*I_yy_3*theta_dot_2*cos(theta2 + 2.0*theta3) + 0.25*I_yz_3*theta_dot_1*cos(2.0*theta2 + theta3) - 0.5*I_xy_3*theta_dot_2*sin(theta2 - 2.0*theta3) + 0.5*I_xy_3*theta_dot_2*sin(theta2 + 2.0*theta3) + 0.25*I_xz_3*theta_dot_1*sin(2.0*theta2 + theta3) - 0.25*I_xx_4*theta_dot_2*cos(theta2 + 2.0*theta3 + 2.0*theta4) + 0.25*I_yy_4*theta_dot_2*cos(theta2 + 2.0*theta3 + 2.0*theta4) + 0.5*I_xy_4*theta_dot_2*sin(theta2 + 2.0*theta3 + 2.0*theta4) + 0.25*I_xx_5*theta_dot_2*cos(theta2 + 2.0*theta3 + 2.0*theta4 + 2.0*theta5) - 0.25*I_yy_5*theta_dot_2*cos(theta2 + 2.0*theta3 + 2.0*theta4 + 2.0*theta5) + 0.5*I_xy_3*theta_dot_1*cos(2.0*theta3) + 0.5*I_xz_4*theta_dot_3*cos(theta3 - theta2 + theta4) + 0.5*I_xz_4*theta_dot_4*cos(theta3 - theta2 + theta4) - 0.5*I_xy_5*theta_dot_2*sin(theta2 + 2.0*theta3 + 2.0*theta4 + 2.0*theta5) + 0.25*I_xx_3*theta_dot_1*sin(2.0*theta3) - 0.25*I_yy_3*theta_dot_1*sin(2.0*theta3) - 0.5*I_yz_4*theta_dot_3*sin(theta3 - theta2 + theta4) - 0.5*I_yz_4*theta_dot_4*sin(theta3 - theta2 + theta4) + 0.5*I_yz_5*theta_dot_3*cos(theta2 + theta3 + theta4 + theta5) + 0.5*I_yz_5*theta_dot_4*cos(theta2 + theta3 + theta4 + theta5) + 0.5*I_yz_5*theta_dot_5*cos(theta2 + theta3 + theta4 + theta5) + 0.5*I_xz_5*theta_dot_3*sin(theta2 + theta3 + theta4 + theta5) + 0.5*I_xz_5*theta_dot_4*sin(theta2 + theta3 + theta4 + theta5) + 0.5*I_xz_5*theta_dot_5*sin(theta2 + theta3 + theta4 + theta5) - 0.25*I_yz_3*theta_dot_1*cos(2.0*theta2 - theta3) + 0.5*I_xz_3*theta_dot_3*cos(theta2 + theta3) + 0.25*I_xz_3*theta_dot_1*sin(2.0*theta2 - theta3) - 0.5*I_yz_3*theta_dot_3*sin(theta2 + theta3) - 0.25*I_xx_4*theta_dot_2*cos(2.0*theta3 - theta2 + 2.0*theta4) + 0.25*I_yy_4*theta_dot_2*cos(2.0*theta3 - theta2 + 2.0*theta4) - 0.25*I_yz_4*theta_dot_1*cos(theta3 - 2.0*theta2 + theta4) + 0.25*I_yz_4*theta_dot_1*cos(2.0*theta2 + theta3 + theta4) + 0.5*I_xy_4*theta_dot_2*sin(2.0*theta3 - theta2 + 2.0*theta4) - 0.25*I_xz_4*theta_dot_1*sin(theta3 - 2.0*theta2 + theta4) + 0.25*I_xz_4*theta_dot_1*sin(2.0*theta2 + theta3 + theta4) + 0.25*I_xx_5*theta_dot_2*cos(2.0*theta3 - theta2 + 2.0*theta4 + 2.0*theta5) - 0.25*I_yy_5*theta_dot_2*cos(2.0*theta3 - theta2 + 2.0*theta4 + 2.0*theta5) + 0.5*I_zz_3*theta_dot_2*cos(theta2) + 0.5*I_zz_4*theta_dot_2*cos(theta2) + 0.5*I_zz_5*theta_dot_2*cos(theta2) - 0.5*I_xy_5*theta_dot_2*sin(2.0*theta3 - theta2 + 2.0*theta4 + 2.0*theta5) + 0.125*lc3_1^2*m3*theta_dot_1*sin(2.0*theta2 - 2.0*theta3) - 0.125*lc3_1^2*m3*theta_dot_1*sin(2.0*theta2 + 2.0*theta3) - 0.125*lc3_2^2*m3*theta_dot_1*sin(2.0*theta2 - 2.0*theta3) + 0.125*lc3_2^2*m3*theta_dot_1*sin(2.0*theta2 + 2.0*theta3) - 0.25*lc4_1^2*m4*theta_dot_1*sin(2.0*theta3 + 2.0*theta4) + 0.25*lc4_2^2*m4*theta_dot_1*sin(2.0*theta3 + 2.0*theta4) - 0.03125*a4^2*m4*theta_dot_1*sin(2.0*theta3 - 2.0*theta2 + 2.0*theta4) - 0.03125*a4^2*m4*theta_dot_1*sin(2.0*theta2 + 2.0*theta3 + 2.0*theta4) - 0.125*a4^2*m5*theta_dot_1*sin(2.0*theta3 - 2.0*theta2 + 2.0*theta4) - 0.125*a4^2*m5*theta_dot_1*sin(2.0*theta2 + 2.0*theta3 + 2.0*theta4) + 0.0625*a5^2*m5*theta_dot_1*sin(2.0*theta3 + 2.0*theta4 + 2.0*theta5) - 0.125*lc4_1^2*m4*theta_dot_1*sin(2.0*theta3 - 2.0*theta2 + 2.0*theta4) - 0.125*lc4_1^2*m4*theta_dot_1*sin(2.0*theta2 + 2.0*theta3 + 2.0*theta4) + 0.125*lc4_2^2*m4*theta_dot_1*sin(2.0*theta3 - 2.0*theta2 + 2.0*theta4) + 0.125*lc4_2^2*m4*theta_dot_1*sin(2.0*theta2 + 2.0*theta3 + 2.0*theta4) + 0.25*lc5_1^2*m5*theta_dot_1*sin(2.0*theta3 + 2.0*theta4 + 2.0*theta5) - 0.25*lc5_2^2*m5*theta_dot_1*sin(2.0*theta3 + 2.0*theta4 + 2.0*theta5) + 0.03125*a5^2*m5*theta_dot_1*sin(2.0*theta3 - 2.0*theta2 + 2.0*theta4 + 2.0*theta5) + 0.03125*a5^2*m5*theta_dot_1*sin(2.0*theta2 + 2.0*theta3 + 2.0*theta4 + 2.0*theta5) + 0.125*lc5_1^2*m5*theta_dot_1*sin(2.0*theta3 - 2.0*theta2 + 2.0*theta4 + 2.0*theta5) + 0.125*lc5_1^2*m5*theta_dot_1*sin(2.0*theta2 + 2.0*theta3 + 2.0*theta4 + 2.0*theta5) - 0.125*lc5_2^2*m5*theta_dot_1*sin(2.0*theta3 - 2.0*theta2 + 2.0*theta4 + 2.0*theta5) - 0.125*lc5_2^2*m5*theta_dot_1*sin(2.0*theta2 + 2.0*theta3 + 2.0*theta4 + 2.0*theta5) + 0.0625*a3^2*m3*theta_dot_2*cos(theta2 - 2.0*theta3) + 0.0625*a3^2*m3*theta_dot_2*cos(theta2 + 2.0*theta3) + 0.25*a3^2*m4*theta_dot_2*cos(theta2 - 2.0*theta3) + 0.25*a3^2*m4*theta_dot_2*cos(theta2 + 2.0*theta3) + 0.25*a3^2*m5*theta_dot_2*cos(theta2 - 2.0*theta3) + 0.25*a3^2*m5*theta_dot_2*cos(theta2 + 2.0*theta3) + 0.25*lc3_1^2*m3*theta_dot_2*cos(theta2 - 2.0*theta3) + 0.25*lc3_1^2*m3*theta_dot_2*cos(theta2 + 2.0*theta3) - 0.25*lc3_2^2*m3*theta_dot_2*cos(theta2 - 2.0*theta3) - 0.25*lc3_2^2*m3*theta_dot_2*cos(theta2 + 2.0*theta3) + 0.0625*a4^2*m4*theta_dot_2*cos(theta2 + 2.0*theta3 + 2.0*theta4) + 0.25*a4^2*m5*theta_dot_2*cos(theta2 + 2.0*theta3 + 2.0*theta4) + 0.25*lc4_1^2*m4*theta_dot_2*cos(theta2 + 2.0*theta3 + 2.0*theta4) - 0.25*lc4_2^2*m4*theta_dot_2*cos(theta2 + 2.0*theta3 + 2.0*theta4) - 0.0625*a5^2*m5*theta_dot_2*cos(theta2 + 2.0*theta3 + 2.0*theta4 + 2.0*theta5) - 0.25*lc5_1^2*m5*theta_dot_2*cos(theta2 + 2.0*theta3 + 2.0*theta4 + 2.0*theta5) + 0.25*lc5_2^2*m5*theta_dot_2*cos(theta2 + 2.0*theta3 + 2.0*theta4 + 2.0*theta5) - 0.0625*a3^2*m3*theta_dot_1*sin(2.0*theta3) - 0.25*a3^2*m4*theta_dot_1*sin(2.0*theta3) - 0.25*a3^2*m5*theta_dot_1*sin(2.0*theta3) - 0.25*lc3_1^2*m3*theta_dot_1*sin(2.0*theta3) + 0.25*lc3_2^2*m3*theta_dot_1*sin(2.0*theta3) + 0.0625*a4^2*m4*theta_dot_2*cos(2.0*theta3 - theta2 + 2.0*theta4) + 0.25*a4^2*m5*theta_dot_2*cos(2.0*theta3 - theta2 + 2.0*theta4) + 0.25*lc4_1^2*m4*theta_dot_2*cos(2.0*theta3 - theta2 + 2.0*theta4) - 0.25*lc4_2^2*m4*theta_dot_2*cos(2.0*theta3 - theta2 + 2.0*theta4) - 0.0625*a5^2*m5*theta_dot_2*cos(2.0*theta3 - theta2 + 2.0*theta4 + 2.0*theta5) + 0.125*a3^2*m3*theta_dot_2*cos(theta2) + 0.5*a3^2*m4*theta_dot_2*cos(theta2) + 0.5*a3^2*m5*theta_dot_2*cos(theta2) + 0.125*a4^2*m4*theta_dot_2*cos(theta2) + 0.5*a4^2*m5*theta_dot_2*cos(theta2) + 0.125*a5^2*m5*theta_dot_2*cos(theta2) - 0.25*lc5_1^2*m5*theta_dot_2*cos(2.0*theta3 - theta2 + 2.0*theta4 + 2.0*theta5) + 0.25*lc5_2^2*m5*theta_dot_2*cos(2.0*theta3 - theta2 + 2.0*theta4 + 2.0*theta5) + 0.5*lc3_1^2*m3*theta_dot_2*cos(theta2) + 0.5*lc3_2^2*m3*theta_dot_2*cos(theta2) + 0.5*lc4_1^2*m4*theta_dot_2*cos(theta2) + 0.5*lc4_2^2*m4*theta_dot_2*cos(theta2) + 0.5*lc5_1^2*m5*theta_dot_2*cos(theta2) + 0.5*lc5_2^2*m5*theta_dot_2*cos(theta2) + 0.03125*a3^2*m3*theta_dot_1*sin(2.0*theta2 - 2.0*theta3) - 0.03125*a3^2*m3*theta_dot_1*sin(2.0*theta2 + 2.0*theta3) + 0.125*a3^2*m4*theta_dot_1*sin(2.0*theta2 - 2.0*theta3) - 0.125*a3^2*m4*theta_dot_1*sin(2.0*theta2 + 2.0*theta3) + 0.125*a3^2*m5*theta_dot_1*sin(2.0*theta2 - 2.0*theta3) - 0.125*a3^2*m5*theta_dot_1*sin(2.0*theta2 + 2.0*theta3) - 0.0625*a4^2*m4*theta_dot_1*sin(2.0*theta3 + 2.0*theta4) - 0.25*a4^2*m5*theta_dot_1*sin(2.0*theta3 + 2.0*theta4) - 0.5*a1*lc5_1*m5*theta_dot_1*cos(theta3 - theta2 + theta4 + theta5) - 0.5*a2*lc5_1*m5*theta_dot_3*cos(theta3 - theta2 + theta4 + theta5) - 0.5*a2*lc5_1*m5*theta_dot_4*cos(theta3 - theta2 + theta4 + theta5) - 0.5*a2*lc5_1*m5*theta_dot_5*cos(theta3 - theta2 + theta4 + theta5) - 0.25*lc3_1*lc3_2*m3*theta_dot_1*cos(2.0*theta2 - 2.0*theta3) - 0.25*lc3_1*lc3_2*m3*theta_dot_1*cos(2.0*theta2 + 2.0*theta3) - 0.5*lc4_1*lc4_2*m4*theta_dot_1*cos(2.0*theta3 + 2.0*theta4) + 0.125*a3*lc3_1*m3*theta_dot_1*sin(2.0*theta2 - 2.0*theta3) - 0.125*a3*lc3_1*m3*theta_dot_1*sin(2.0*theta2 + 2.0*theta3) - 0.25*a4*lc4_1*m4*theta_dot_1*sin(2.0*theta3 + 2.0*theta4) - 0.125*a4*lc4_2*m4*theta_dot_1*cos(2.0*theta3 - 2.0*theta2 + 2.0*theta4) - 0.125*a4*lc4_2*m4*theta_dot_1*cos(2.0*theta2 + 2.0*theta3 + 2.0*theta4) + 0.25*a5*lc5_2*m5*theta_dot_1*cos(2.0*theta3 + 2.0*theta4 + 2.0*theta5) - 0.5*lc5_2*lc5_3*m5*theta_dot_3*cos(theta3 - theta2 + theta4 + theta5) - 0.5*lc5_2*lc5_3*m5*theta_dot_4*cos(theta3 - theta2 + theta4 + theta5) - 0.5*lc5_2*lc5_3*m5*theta_dot_5*cos(theta3 - theta2 + theta4 + theta5) + 0.25*a3*a4*m4*theta_dot_2*cos(theta2 - theta4) + 0.5*a3*a4*m5*theta_dot_2*cos(theta2 - theta4) - 0.25*a3*a4*m4*theta_dot_4*cos(theta2 - theta4) - 0.5*a3*a4*m5*theta_dot_4*cos(theta2 - theta4) + 0.5*a1*lc5_2*m5*theta_dot_1*sin(theta3 - theta2 + theta4 + theta5) + 0.5*a2*lc5_2*m5*theta_dot_3*sin(theta3 - theta2 + theta4 + theta5) + 0.5*a2*lc5_2*m5*theta_dot_4*sin(theta3 - theta2 + theta4 + theta5) + 0.5*a2*lc5_2*m5*theta_dot_5*sin(theta3 - theta2 + theta4 + theta5) - 0.25*a5*lc5_3*m5*theta_dot_3*sin(theta3 - theta2 + theta4 + theta5) - 0.25*a5*lc5_3*m5*theta_dot_4*sin(theta3 - theta2 + theta4 + theta5) - 0.25*a5*lc5_3*m5*theta_dot_5*sin(theta3 - theta2 + theta4 + theta5) - 0.25*lc4_1*lc4_2*m4*theta_dot_1*cos(2.0*theta3 - 2.0*theta2 + 2.0*theta4) - 0.25*lc4_1*lc4_2*m4*theta_dot_1*cos(2.0*theta2 + 2.0*theta3 + 2.0*theta4) + 0.5*lc5_1*lc5_2*m5*theta_dot_1*cos(2.0*theta3 + 2.0*theta4 + 2.0*theta5) + 0.5*a1*lc3_2*m3*theta_dot_1*cos(theta2 - theta3) + 0.5*a2*lc3_2*m3*theta_dot_3*cos(theta2 - theta3) - 0.25*a3*lc3_3*m3*theta_dot_3*cos(theta2 - theta3) + 0.5*a3*lc4_1*m4*theta_dot_2*cos(theta2 - theta4) - 0.5*a3*lc4_1*m4*theta_dot_4*cos(theta2 - theta4) - 0.5*a3*lc4_3*m4*theta_dot_3*cos(theta2 - theta3) - 0.5*a3*lc5_3*m5*theta_dot_3*cos(theta2 - theta3) + 0.5*a4*lc5_2*m5*theta_dot_2*cos(theta2 - theta5) - 0.5*a4*lc5_2*m5*theta_dot_5*cos(theta2 - theta5) - 0.125*a4*lc4_1*m4*theta_dot_1*sin(2.0*theta3 - 2.0*theta2 + 2.0*theta4) - 0.125*a4*lc4_1*m4*theta_dot_1*sin(2.0*theta2 + 2.0*theta3 + 2.0*theta4) + 0.25*a5*lc5_1*m5*theta_dot_1*sin(2.0*theta3 + 2.0*theta4 + 2.0*theta5) - 0.5*lc5_1*lc5_3*m5*theta_dot_3*sin(theta3 - theta2 + theta4 + theta5) - 0.5*lc5_1*lc5_3*m5*theta_dot_4*sin(theta3 - theta2 + theta4 + theta5) - 0.5*lc5_1*lc5_3*m5*theta_dot_5*sin(theta3 - theta2 + theta4 + theta5) - 0.25*a1*a3*m3*theta_dot_1*sin(theta2 - theta3) - 0.5*a1*a3*m4*theta_dot_1*sin(theta2 - theta3) - 0.5*a1*a3*m5*theta_dot_1*sin(theta2 - theta3) - 0.25*a2*a3*m3*theta_dot_3*sin(theta2 - theta3) - 0.5*a2*a3*m4*theta_dot_3*sin(theta2 - theta3) - 0.5*a2*a3*m5*theta_dot_3*sin(theta2 - theta3) - 0.25*a4*a5*m5*theta_dot_2*sin(theta2 - theta5) + 0.25*a4*a5*m5*theta_dot_5*sin(theta2 - theta5) + 0.125*a5*lc5_2*m5*theta_dot_1*cos(2.0*theta3 - 2.0*theta2 + 2.0*theta4 + 2.0*theta5) + 0.125*a5*lc5_2*m5*theta_dot_1*cos(2.0*theta2 + 2.0*theta3 + 2.0*theta4 + 2.0*theta5) + 0.25*a3*a4*m4*theta_dot_2*cos(2.0*theta3 - theta2 + theta4) + 0.5*a3*a4*m5*theta_dot_2*cos(2.0*theta3 - theta2 + theta4) - 0.5*lc3_1*lc3_3*m3*theta_dot_3*cos(theta2 - theta3) - 0.5*a1*lc3_1*m3*theta_dot_1*sin(theta2 - theta3) - 0.5*a2*lc3_1*m3*theta_dot_3*sin(theta2 - theta3) + 0.5*a3*lc4_2*m4*theta_dot_2*sin(theta2 - theta4) - 0.5*a3*lc4_2*m4*theta_dot_4*sin(theta2 - theta4) - 0.5*a4*lc5_1*m5*theta_dot_2*sin(theta2 - theta5) + 0.5*a4*lc5_1*m5*theta_dot_5*sin(theta2 - theta5) + 0.25*lc5_1*lc5_2*m5*theta_dot_1*cos(2.0*theta3 - 2.0*theta2 + 2.0*theta4 + 2.0*theta5) + 0.25*lc5_1*lc5_2*m5*theta_dot_1*cos(2.0*theta2 + 2.0*theta3 + 2.0*theta4 + 2.0*theta5) + 0.5*a3*lc4_1*m4*theta_dot_2*cos(2.0*theta3 - theta2 + theta4) - 0.5*a1*lc4_2*m4*theta_dot_1*cos(theta2 + theta3 + theta4) - 0.5*a2*lc4_2*m4*theta_dot_3*cos(theta2 + theta3 + theta4) - 0.5*a2*lc4_2*m4*theta_dot_4*cos(theta2 + theta3 + theta4) - 0.25*a4*lc4_3*m4*theta_dot_3*cos(theta2 + theta3 + theta4) - 0.25*a4*lc4_3*m4*theta_dot_4*cos(theta2 + theta3 + theta4) - 0.5*a2*lc5_2*m5*theta_dot_1*cos(theta3 + theta4 + theta5) - 1.0*a1*lc5_2*m5*theta_dot_3*cos(theta3 + theta4 + theta5) + 0.5*a3*lc5_2*m5*theta_dot_2*cos(theta2 + theta4 + theta5) - 1.0*a1*lc5_2*m5*theta_dot_4*cos(theta3 + theta4 + theta5) - 0.5*a4*lc5_3*m5*theta_dot_3*cos(theta2 + theta3 + theta4) - 1.0*a1*lc5_2*m5*theta_dot_5*cos(theta3 + theta4 + theta5) + 0.5*a3*lc5_2*m5*theta_dot_4*cos(theta2 + theta4 + theta5) - 0.5*a4*lc5_3*m5*theta_dot_4*cos(theta2 + theta3 + theta4) + 0.5*a3*lc5_2*m5*theta_dot_5*cos(theta2 + theta4 + theta5) + 0.125*a5*lc5_1*m5*theta_dot_1*sin(2.0*theta3 - 2.0*theta2 + 2.0*theta4 + 2.0*theta5) + 0.125*a5*lc5_1*m5*theta_dot_1*sin(2.0*theta2 + 2.0*theta3 + 2.0*theta4 + 2.0*theta5) - 0.25*a1*a4*m4*theta_dot_1*sin(theta2 + theta3 + theta4) - 0.5*a1*a4*m5*theta_dot_1*sin(theta2 + theta3 + theta4) - 0.25*a2*a4*m4*theta_dot_3*sin(theta2 + theta3 + theta4) - 0.25*a2*a4*m4*theta_dot_4*sin(theta2 + theta3 + theta4) - 0.5*a2*a4*m5*theta_dot_3*sin(theta2 + theta3 + theta4) - 0.5*a2*a4*m5*theta_dot_4*sin(theta2 + theta3 + theta4) - 0.25*a2*a5*m5*theta_dot_1*sin(theta3 + theta4 + theta5) - 0.5*a1*a5*m5*theta_dot_3*sin(theta3 + theta4 + theta5) 
C13b = 0.25*a3*a5*m5*theta_dot_2*sin(theta2 + theta4 + theta5) - 0.5*a1*a5*m5*theta_dot_4*sin(theta3 + theta4 + theta5) - 0.5*a1*a5*m5*theta_dot_5*sin(theta3 + theta4 + theta5) + 0.25*a3*a5*m5*theta_dot_4*sin(theta2 + theta4 + theta5) + 0.25*a3*a5*m5*theta_dot_5*sin(theta2 + theta4 + theta5) - 0.5*lc3_2*lc3_3*m3*theta_dot_3*sin(theta2 - theta3) - 0.5*lc4_1*lc4_3*m4*theta_dot_3*cos(theta2 + theta3 + theta4) - 0.5*lc4_1*lc4_3*m4*theta_dot_4*cos(theta2 + theta3 + theta4) - 0.5*a3*lc4_2*m4*theta_dot_2*sin(2.0*theta3 - theta2 + theta4) - 0.5*a1*lc4_1*m4*theta_dot_1*sin(theta2 + theta3 + theta4) - 0.5*a2*lc4_1*m4*theta_dot_3*sin(theta2 + theta3 + theta4) - 0.5*a2*lc4_1*m4*theta_dot_4*sin(theta2 + theta3 + theta4) - 0.5*a2*lc5_1*m5*theta_dot_1*sin(theta3 + theta4 + theta5) - 1.0*a1*lc5_1*m5*theta_dot_3*sin(theta3 + theta4 + theta5) + 0.5*a3*lc5_1*m5*theta_dot_2*sin(theta2 + theta4 + theta5) - 1.0*a1*lc5_1*m5*theta_dot_4*sin(theta3 + theta4 + theta5) - 1.0*a1*lc5_1*m5*theta_dot_5*sin(theta3 + theta4 + theta5) + 0.5*a3*lc5_1*m5*theta_dot_4*sin(theta2 + theta4 + theta5) + 0.5*a3*lc5_1*m5*theta_dot_5*sin(theta2 + theta4 + theta5) + 0.5*a4*lc5_2*m5*theta_dot_2*cos(2.0*theta3 - theta2 + 2.0*theta4 + theta5) + 0.25*a2*lc5_2*m5*theta_dot_1*cos(theta3 - 2.0*theta2 + theta4 + theta5) + 0.25*a2*lc5_2*m5*theta_dot_1*cos(2.0*theta2 + theta3 + theta4 + theta5) + 0.5*a3*lc5_2*m5*theta_dot_2*cos(theta2 + 2.0*theta3 + theta4 + theta5) - 0.125*a5*lc5_3*m5*theta_dot_1*cos(theta3 - 2.0*theta2 + theta4 + theta5) + 0.125*a5*lc5_3*m5*theta_dot_1*cos(2.0*theta2 + theta3 + theta4 + theta5) + 0.25*a4*a5*m5*theta_dot_2*sin(2.0*theta3 - theta2 + 2.0*theta4 + theta5) + 0.125*a2*a5*m5*theta_dot_1*sin(theta3 - 2.0*theta2 + theta4 + theta5) + 0.125*a2*a5*m5*theta_dot_1*sin(2.0*theta2 + theta3 + theta4 + theta5) + 0.25*a3*a5*m5*theta_dot_2*sin(theta2 + 2.0*theta3 + theta4 + theta5) + 0.5*lc4_2*lc4_3*m4*theta_dot_3*sin(theta2 + theta3 + theta4) + 0.5*lc4_2*lc4_3*m4*theta_dot_4*sin(theta2 + theta3 + theta4) - 0.25*lc5_1*lc5_3*m5*theta_dot_1*cos(theta3 - 2.0*theta2 + theta4 + theta5) + 0.25*lc5_1*lc5_3*m5*theta_dot_1*cos(2.0*theta2 + theta3 + theta4 + theta5) + 0.125*a2*a3*m3*theta_dot_1*cos(2.0*theta2 + theta3) + 0.25*a2*a3*m4*theta_dot_1*cos(2.0*theta2 + theta3) + 0.25*a2*a3*m5*theta_dot_1*cos(2.0*theta2 + theta3) + 0.5*a4*lc5_1*m5*theta_dot_2*sin(2.0*theta3 - theta2 + 2.0*theta4 + theta5) + 0.25*a2*lc5_1*m5*theta_dot_1*sin(theta3 - 2.0*theta2 + theta4 + theta5) + 0.25*a2*lc5_1*m5*theta_dot_1*sin(2.0*theta2 + theta3 + theta4 + theta5) + 0.5*a3*lc5_1*m5*theta_dot_2*sin(theta2 + 2.0*theta3 + theta4 + theta5) + 0.25*a2*lc3_1*m3*theta_dot_1*cos(2.0*theta2 + theta3) + 0.25*a3*lc3_1*m3*theta_dot_2*cos(theta2 - 2.0*theta3) + 0.25*a3*lc3_1*m3*theta_dot_2*cos(theta2 + 2.0*theta3) - 0.5*a3*lc4_2*m4*theta_dot_1*cos(2.0*theta3 + theta4) + 0.25*lc5_2*lc5_3*m5*theta_dot_1*sin(theta3 - 2.0*theta2 + theta4 + theta5) - 0.25*lc5_2*lc5_3*m5*theta_dot_1*sin(2.0*theta2 + theta3 + theta4 + theta5) - 0.25*a3*a4*m4*theta_dot_1*sin(2.0*theta3 + theta4) - 0.5*a3*a4*m5*theta_dot_1*sin(2.0*theta3 + theta4) + 0.25*a4*a5*m5*theta_dot_1*cos(2.0*theta3 + 2.0*theta4 + theta5) - 0.25*lc3_2*lc3_3*m3*theta_dot_1*cos(2.0*theta2 + theta3) - 0.25*a2*lc3_2*m3*theta_dot_1*sin(2.0*theta2 + theta3) + 0.25*a3*lc3_2*m3*theta_dot_2*sin(theta2 - 2.0*theta3) - 0.25*a3*lc3_2*m3*theta_dot_2*sin(theta2 + 2.0*theta3) - 0.125*a3*lc3_3*m3*theta_dot_1*sin(2.0*theta2 + theta3) - 0.5*a3*lc4_1*m4*theta_dot_1*sin(2.0*theta3 + theta4) - 0.25*a3*lc4_3*m4*theta_dot_1*sin(2.0*theta2 + theta3) - 0.25*a3*lc5_3*m5*theta_dot_1*sin(2.0*theta2 + theta3) - 0.25*a3*lc4_2*m4*theta_dot_1*cos(2.0*theta3 - 2.0*theta2 + theta4) - 0.25*a3*lc4_2*m4*theta_dot_1*cos(2.0*theta2 + 2.0*theta3 + theta4) + 0.25*a4*lc4_1*m4*theta_dot_2*cos(theta2 + 2.0*theta3 + 2.0*theta4) + 0.5*a4*lc5_1*m5*theta_dot_1*cos(2.0*theta3 + 2.0*theta4 + theta5) - 0.125*a3*a4*m4*theta_dot_1*sin(2.0*theta3 - 2.0*theta2 + theta4) - 0.125*a3*a4*m4*theta_dot_1*sin(2.0*theta2 + 2.0*theta3 + theta4) - 0.25*a3*a4*m5*theta_dot_1*sin(2.0*theta3 - 2.0*theta2 + theta4) - 0.25*a3*a4*m5*theta_dot_1*sin(2.0*theta2 + 2.0*theta3 + theta4) + 0.5*lc3_1*lc3_2*m3*theta_dot_2*sin(theta2 - 2.0*theta3) - 0.5*lc3_1*lc3_2*m3*theta_dot_2*sin(theta2 + 2.0*theta3) - 0.25*lc3_1*lc3_3*m3*theta_dot_1*sin(2.0*theta2 + theta3) + 0.125*a4*a5*m5*theta_dot_1*cos(2.0*theta3 - 2.0*theta2 + 2.0*theta4 + theta5) + 0.125*a4*a5*m5*theta_dot_1*cos(2.0*theta2 + 2.0*theta3 + 2.0*theta4 + theta5) - 0.25*a3*lc4_1*m4*theta_dot_1*sin(2.0*theta3 - 2.0*theta2 + theta4) - 0.25*a3*lc4_1*m4*theta_dot_1*sin(2.0*theta2 + 2.0*theta3 + theta4) - 0.25*a4*lc4_2*m4*theta_dot_2*sin(theta2 + 2.0*theta3 + 2.0*theta4) - 0.5*a4*lc5_2*m5*theta_dot_1*sin(2.0*theta3 + 2.0*theta4 + theta5) + 0.25*a4*lc5_1*m5*theta_dot_1*cos(2.0*theta3 - 2.0*theta2 + 2.0*theta4 + theta5) + 0.25*a4*lc5_1*m5*theta_dot_1*cos(2.0*theta2 + 2.0*theta3 + 2.0*theta4 + theta5) - 0.25*a5*lc5_1*m5*theta_dot_2*cos(theta2 + 2.0*theta3 + 2.0*theta4 + 2.0*theta5) - 0.25*a3*lc3_2*m3*theta_dot_1*cos(2.0*theta3) - 0.5*lc4_1*lc4_2*m4*theta_dot_2*sin(theta2 + 2.0*theta3 + 2.0*theta4) + 0.5*a1*lc4_2*m4*theta_dot_1*cos(theta3 - theta2 + theta4) + 0.5*a2*lc4_2*m4*theta_dot_3*cos(theta3 - theta2 + theta4) + 0.5*a2*lc4_2*m4*theta_dot_4*cos(theta3 - theta2 + theta4) - 0.25*a4*lc4_3*m4*theta_dot_3*cos(theta3 - theta2 + theta4) - 0.25*a4*lc4_3*m4*theta_dot_4*cos(theta3 - theta2 + theta4) + 0.5*a3*lc5_2*m5*theta_dot_2*cos(theta4 - theta2 + theta5) - 0.5*a4*lc5_3*m5*theta_dot_3*cos(theta3 - theta2 + theta4) - 0.5*a3*lc5_2*m5*theta_dot_4*cos(theta4 - theta2 + theta5) - 0.5*a4*lc5_3*m5*theta_dot_4*cos(theta3 - theta2 + theta4) - 0.5*a3*lc5_2*m5*theta_dot_5*cos(theta4 - theta2 + theta5) - 0.5*lc3_1*lc3_2*m3*theta_dot_1*cos(2.0*theta3) - 0.25*a4*lc5_2*m5*theta_dot_1*sin(2.0*theta3 - 2.0*theta2 + 2.0*theta4 + theta5) - 0.25*a4*lc5_2*m5*theta_dot_1*sin(2.0*theta2 + 2.0*theta3 + 2.0*theta4 + theta5) + 0.25*a5*lc5_2*m5*theta_dot_2*sin(theta2 + 2.0*theta3 + 2.0*theta4 + 2.0*theta5) + 0.25*a1*a4*m4*theta_dot_1*sin(theta3 - theta2 + theta4) + 0.5*a1*a4*m5*theta_dot_1*sin(theta3 - theta2 + theta4) + 0.25*a2*a4*m4*theta_dot_3*sin(theta3 - theta2 + theta4) + 0.25*a2*a4*m4*theta_dot_4*sin(theta3 - theta2 + theta4) + 0.5*a2*a4*m5*theta_dot_3*sin(theta3 - theta2 + theta4) + 0.5*a2*a4*m5*theta_dot_4*sin(theta3 - theta2 + theta4) + 0.25*a3*a5*m5*theta_dot_2*sin(theta4 - theta2 + theta5) - 0.25*a3*a5*m5*theta_dot_4*sin(theta4 - theta2 + theta5) - 0.25*a3*a5*m5*theta_dot_5*sin(theta4 - theta2 + theta5) - 0.25*a3*lc3_1*m3*theta_dot_1*sin(2.0*theta3) + 0.25*a1*a5*m5*theta_dot_1*cos(theta2 + theta3 + theta4 + theta5) + 0.25*a2*a5*m5*theta_dot_3*cos(theta2 + theta3 + theta4 + theta5) + 0.25*a2*a5*m5*theta_dot_4*cos(theta2 + theta3 + theta4 + theta5) + 0.25*a2*a5*m5*theta_dot_5*cos(theta2 + theta3 + theta4 + theta5) - 0.5*lc4_1*lc4_3*m4*theta_dot_3*cos(theta3 - theta2 + theta4) - 0.5*lc4_1*lc4_3*m4*theta_dot_4*cos(theta3 - theta2 + theta4) + 0.5*lc5_1*lc5_2*m5*theta_dot_2*sin(theta2 + 2.0*theta3 + 2.0*theta4 + 2.0*theta5) + 0.5*a1*lc4_1*m4*theta_dot_1*sin(theta3 - theta2 + theta4) + 0.5*a2*lc4_1*m4*theta_dot_3*sin(theta3 - theta2 + theta4) + 0.5*a2*lc4_1*m4*theta_dot_4*sin(theta3 - theta2 + theta4) + 0.5*a3*lc5_1*m5*theta_dot_2*sin(theta4 - theta2 + theta5) - 0.5*a3*lc5_1*m5*theta_dot_4*sin(theta4 - theta2 + theta5) - 0.5*a3*lc5_1*m5*theta_dot_5*sin(theta4 - theta2 + theta5) + 0.5*a3*lc5_2*m5*theta_dot_2*cos(2.0*theta3 - theta2 + theta4 + theta5) + 0.5*a1*lc5_1*m5*theta_dot_1*cos(theta2 + theta3 + theta4 + theta5) + 0.5*a2*lc5_1*m5*theta_dot_3*cos(theta2 + theta3 + theta4 + theta5) + 0.5*a2*lc5_1*m5*theta_dot_4*cos(theta2 + theta3 + theta4 + theta5) + 0.5*a2*lc5_1*m5*theta_dot_5*cos(theta2 + theta3 + theta4 + theta5) + 0.25*a3*a5*m5*theta_dot_2*sin(2.0*theta3 - theta2 + theta4 + theta5) + 0.5*lc4_2*lc4_3*m4*theta_dot_3*sin(theta3 - theta2 + theta4) + 0.5*lc4_2*lc4_3*m4*theta_dot_4*sin(theta3 - theta2 + theta4) + 0.125*a2*a3*m3*theta_dot_1*cos(2.0*theta2 - theta3) + 0.25*a2*a3*m4*theta_dot_1*cos(2.0*theta2 - theta3) + 0.25*a2*a3*m5*theta_dot_1*cos(2.0*theta2 - theta3) - 0.5*lc5_2*lc5_3*m5*theta_dot_3*cos(theta2 + theta3 + theta4 + theta5) - 0.5*lc5_2*lc5_3*m5*theta_dot_4*cos(theta2 + theta3 + theta4 + theta5) - 0.5*lc5_2*lc5_3*m5*theta_dot_5*cos(theta2 + theta3 + theta4 + theta5) - 0.25*a2*a4*m4*theta_dot_1*cos(theta3 + theta4) - 0.5*a1*a4*m4*theta_dot_3*cos(theta3 + theta4) - 0.5*a2*a4*m5*theta_dot_1*cos(theta3 + theta4) + 0.25*a3*a4*m4*theta_dot_2*cos(theta2 + theta4) - 0.5*a1*a4*m4*theta_dot_4*cos(theta3 + theta4) - 1.0*a1*a4*m5*theta_dot_3*cos(theta3 + theta4) + 0.5*a3*a4*m5*theta_dot_2*cos(theta2 + theta4) - 1.0*a1*a4*m5*theta_dot_4*cos(theta3 + theta4) + 0.25*a3*a4*m4*theta_dot_4*cos(theta2 + theta4) + 0.5*a3*a4*m5*theta_dot_4*cos(theta2 + theta4) + 0.5*a3*lc5_1*m5*theta_dot_2*sin(2.0*theta3 - theta2 + theta4 + theta5) - 0.5*a1*lc5_2*m5*theta_dot_1*sin(theta2 + theta3 + theta4 + theta5) - 0.5*a2*lc5_2*m5*theta_dot_3*sin(theta2 + theta3 + theta4 + theta5) - 0.5*a2*lc5_2*m5*theta_dot_4*sin(theta2 + theta3 + theta4 + theta5) - 0.5*a2*lc5_2*m5*theta_dot_5*sin(theta2 + theta3 + theta4 + theta5) - 0.25*a5*lc5_3*m5*theta_dot_3*sin(theta2 + theta3 + theta4 + theta5) - 0.25*a5*lc5_3*m5*theta_dot_4*sin(theta2 + theta3 + theta4 + theta5) - 0.25*a5*lc5_3*m5*theta_dot_5*sin(theta2 + theta3 + theta4 + theta5) + 0.25*a2*lc3_1*m3*theta_dot_1*cos(2.0*theta2 - theta3) - 0.5*a1*lc3_2*m3*theta_dot_1*cos(theta2 + theta3) - 0.5*a2*lc3_2*m3*theta_dot_3*cos(theta2 + theta3) - 0.25*a3*lc3_3*m3*theta_dot_3*cos(theta2 + theta3) - 0.5*a2*lc4_1*m4*theta_dot_1*cos(theta3 + theta4) - 1.0*a1*lc4_1*m4*theta_dot_3*cos(theta3 + theta4) + 0.5*a3*lc4_1*m4*theta_dot_2*cos(theta2 + theta4) - 1.0*a1*lc4_1*m4*theta_dot_4*cos(theta3 + theta4) + 0.5*a3*lc4_1*m4*theta_dot_4*cos(theta2 + theta4) - 0.5*a3*lc4_3*m4*theta_dot_3*cos(theta2 + theta3) - 0.5*a3*lc5_3*m5*theta_dot_3*cos(theta2 + theta3) + 0.5*a4*lc5_2*m5*theta_dot_2*cos(theta2 + theta5) + 0.5*a4*lc5_2*m5*theta_dot_5*cos(theta2 + theta5) - 0.5*lc5_1*lc5_3*m5*theta_dot_3*sin(theta2 + theta3 + theta4 + theta5) - 0.5*lc5_1*lc5_3*m5*theta_dot_4*sin(theta2 + theta3 + theta4 + theta5) - 0.5*lc5_1*lc5_3*m5*theta_dot_5*sin(theta2 + theta3 + theta4 + theta5) - 0.25*a1*a3*m3*theta_dot_1*sin(theta2 + theta3) - 0.5*a1*a3*m4*theta_dot_1*sin(theta2 + theta3) - 0.5*a1*a3*m5*theta_dot_1*sin(theta2 + theta3) - 0.25*a2*a3*m3*theta_dot_3*sin(theta2 + theta3) - 0.5*a2*a3*m4*theta_dot_3*sin(theta2 + theta3) - 0.5*a2*a3*m5*theta_dot_3*sin(theta2 + theta3) + 0.25*a4*a5*m5*theta_dot_2*sin(theta2 + theta5) + 0.25*a4*a5*m5*theta_dot_5*sin(theta2 + theta5) + 0.125*a2*a4*m4*theta_dot_1*cos(theta3 - 2.0*theta2 + theta4) + 0.125*a2*a4*m4*theta_dot_1*cos(2.0*theta2 + theta3 + theta4) + 0.25*a2*a4*m5*theta_dot_1*cos(theta3 - 2.0*theta2 + theta4) + 0.25*a2*a4*m5*theta_dot_1*cos(2.0*theta2 + theta3 + theta4) + 0.25*a3*a4*m4*theta_dot_2*cos(theta2 + 2.0*theta3 + theta4) + 0.5*a3*a4*m5*theta_dot_2*cos(theta2 + 2.0*theta3 + theta4) + 0.25*a3*a5*m5*theta_dot_1*cos(2.0*theta3 + theta4 + theta5) + 0.25*lc3_2*lc3_3*m3*theta_dot_1*cos(2.0*theta2 - theta3) - 0.5*lc3_1*lc3_3*m3*theta_dot_3*cos(theta2 + theta3) + 0.25*a2*lc3_2*m3*theta_dot_1*sin(2.0*theta2 - theta3) - 0.125*a3*lc3_3*m3*theta_dot_1*sin(2.0*theta2 - theta3) - 0.25*a3*lc4_3*m4*theta_dot_1*sin(2.0*theta2 - theta3) - 0.25*a3*lc5_3*m5*theta_dot_1*sin(2.0*theta2 - theta3) - 0.5*a1*lc3_1*m3*theta_dot_1*sin(theta2 + theta3) - 0.5*a2*lc3_1*m3*theta_dot_3*sin(theta2 + theta3) + 0.5*a2*lc4_2*m4*theta_dot_1*sin(theta3 + theta4) + 1.0*a1*lc4_2*m4*theta_dot_3*sin(theta3 + theta4) - 0.5*a3*lc4_2*m4*theta_dot_2*sin(theta2 + theta4) + 1.0*a1*lc4_2*m4*theta_dot_4*sin(theta3 + theta4) - 0.5*a3*lc4_2*m4*theta_dot_4*sin(theta2 + theta4) + 0.5*a4*lc5_1*m5*theta_dot_2*sin(theta2 + theta5) + 0.5*a4*lc5_1*m5*theta_dot_5*sin(theta2 + theta5) + 0.25*a4*lc4_1*m4*theta_dot_2*cos(2.0*theta3 - theta2 + 2.0*theta4) + 0.25*a2*lc4_1*m4*theta_dot_1*cos(theta3 - 2.0*theta2 + theta4) + 0.25*a2*lc4_1*m4*theta_dot_1*cos(2.0*theta2 + theta3 + theta4) + 0.5*a3*lc4_1*m4*theta_dot_2*cos(theta2 + 2.0*theta3 + theta4) + 0.5*a3*lc5_1*m5*theta_dot_1*cos(2.0*theta3 + theta4 + theta5) - 0.25*lc3_1*lc3_3*m3*theta_dot_1*sin(2.0*theta2 - theta3) + 0.5*lc3_2*lc3_3*m3*theta_dot_3*sin(theta2 + theta3) + 0.125*a3*a5*m5*theta_dot_1*cos(2.0*theta3 - 2.0*theta2 + theta4 + theta5) + 0.125*a3*a5*m5*theta_dot_1*cos(2.0*theta2 + 2.0*theta3 + theta4 + theta5) + 0.25*lc4_2*lc4_3*m4*theta_dot_1*cos(theta3 - 2.0*theta2 + theta4) - 0.25*lc4_2*lc4_3*m4*theta_dot_1*cos(2.0*theta2 + theta3 + theta4) - 0.25*a2*a3*m3*theta_dot_1*cos(theta3) - 0.5*a1*a3*m3*theta_dot_3*cos(theta3) - 0.5*a2*a3*m4*theta_dot_1*cos(theta3) - 1.0*a1*a3*m4*theta_dot_3*cos(theta3) - 0.5*a2*a3*m5*theta_dot_1*cos(theta3) - 1.0*a1*a3*m5*theta_dot_3*cos(theta3) - 0.25*a4*lc4_2*m4*theta_dot_2*sin(2.0*theta3 - theta2 + 2.0*theta4) - 0.25*a2*lc4_2*m4*theta_dot_1*sin(theta3 - 2.0*theta2 + theta4) - 0.25*a2*lc4_2*m4*theta_dot_1*sin(2.0*theta2 + theta3 + theta4) - 0.5*a3*lc4_2*m4*theta_dot_2*sin(theta2 + 2.0*theta3 + theta4) + 0.125*a4*lc4_3*m4*theta_dot_1*sin(theta3 - 2.0*theta2 + theta4) - 0.125*a4*lc4_3*m4*theta_dot_1*sin(2.0*theta2 + theta3 + theta4) + 0.25*a4*lc5_3*m5*theta_dot_1*sin(theta3 - 2.0*theta2 + theta4) - 0.25*a4*lc5_3*m5*theta_dot_1*sin(2.0*theta2 + theta3 + theta4) - 0.5*a3*lc5_2*m5*theta_dot_1*sin(2.0*theta3 + theta4 + theta5) - 0.25*a5*lc5_1*m5*theta_dot_2*cos(2.0*theta3 - theta2 + 2.0*theta4 + 2.0*theta5) + 0.25*a3*lc5_1*m5*theta_dot_1*cos(2.0*theta3 - 2.0*theta2 + theta4 + theta5) + 0.25*a3*lc5_1*m5*theta_dot_1*cos(2.0*theta2 + 2.0*theta3 + theta4 + theta5) + 0.5*a4*lc5_2*m5*theta_dot_2*cos(theta2 + 2.0*theta3 + 2.0*theta4 + theta5) - 0.5*a2*lc3_1*m3*theta_dot_1*cos(theta3) - 1.0*a1*lc3_1*m3*theta_dot_3*cos(theta3) + 0.5*a3*lc3_1*m3*theta_dot_2*cos(theta2) + 0.5*a4*lc4_1*m4*theta_dot_2*cos(theta2) + 0.5*a5*lc5_1*m5*theta_dot_2*cos(theta2) + 0.25*a4*a5*m5*theta_dot_2*sin(theta2 + 2.0*theta3 + 2.0*theta4 + theta5) - 0.5*lc4_1*lc4_2*m4*theta_dot_2*sin(2.0*theta3 - theta2 + 2.0*theta4) + 0.25*lc4_1*lc4_3*m4*theta_dot_1*sin(theta3 - 2.0*theta2 + theta4) - 0.25*lc4_1*lc4_3*m4*theta_dot_1*sin(2.0*theta2 + theta3 + theta4) + 0.25*a5*lc5_2*m5*theta_dot_2*sin(2.0*theta3 - theta2 + 2.0*theta4 + 2.0*theta5) - 0.25*a3*lc5_2*m5*theta_dot_1*sin(2.0*theta3 - 2.0*theta2 + theta4 + theta5) - 0.25*a3*lc5_2*m5*theta_dot_1*sin(2.0*theta2 + 2.0*theta3 + theta4 + theta5) + 0.5*a4*lc5_1*m5*theta_dot_2*sin(theta2 + 2.0*theta3 + 2.0*theta4 + theta5) + 0.5*a2*lc3_2*m3*theta_dot_1*sin(theta3) + 1.0*a1*lc3_2*m3*theta_dot_3*sin(theta3) - 0.25*a1*a5*m5*theta_dot_1*cos(theta3 - theta2 + theta4 + theta5) - 0.25*a2*a5*m5*theta_dot_3*cos(theta3 - theta2 + theta4 + theta5) - 0.25*a2*a5*m5*theta_dot_4*cos(theta3 - theta2 + theta4 + theta5) - 0.25*a2*a5*m5*theta_dot_5*cos(theta3 - theta2 + theta4 + theta5) - 0.125*a3*lc3_2*m3*theta_dot_1*cos(2.0*theta2 - 2.0*theta3) - 0.125*a3*lc3_2*m3*theta_dot_1*cos(2.0*theta2 + 2.0*theta3) - 0.25*a4*lc4_2*m4*theta_dot_1*cos(2.0*theta3 + 2.0*theta4) + 0.5*lc5_1*lc5_2*m5*theta_dot_2*sin(2.0*theta3 - theta2 + 2.0*theta4 + 2.0*theta5)
C13  = C13a + C13b 
C14 = 0.5*I_yz_5*theta_dot_3*cos(theta3 - theta2 + theta4 + theta5) + 0.5*I_yz_5*theta_dot_4*cos(theta3 - theta2 + theta4 + theta5) + 0.5*I_yz_5*theta_dot_5*cos(theta3 - theta2 + theta4 + theta5) + 0.5*I_xz_5*theta_dot_3*sin(theta3 - theta2 + theta4 + theta5) + 0.5*I_xz_5*theta_dot_4*sin(theta3 - theta2 + theta4 + theta5) + 0.5*I_xz_5*theta_dot_5*sin(theta3 - theta2 + theta4 + theta5) - 0.25*I_xy_5*theta_dot_1*cos(2*theta2 + 2*theta3 + 2*theta4 + 2*theta5) + 0.5*I_xz_4*theta_dot_3*cos(theta2 + theta3 + theta4) + 0.5*I_xz_4*theta_dot_4*cos(theta2 + theta3 + theta4) - 0.125*I_xx_5*theta_dot_1*sin(2*theta2 + 2*theta3 + 2*theta4 + 2*theta5) + 0.125*I_yy_5*theta_dot_1*sin(2*theta2 + 2*theta3 + 2*theta4 + 2*theta5) - 0.5*I_yz_4*theta_dot_3*sin(theta2 + theta3 + theta4) - 0.5*I_yz_4*theta_dot_4*sin(theta2 + theta3 + theta4) + 0.25*I_xz_5*theta_dot_1*cos(theta3 - 2.0*theta2 + theta4 + theta5) - 0.25*I_xz_5*theta_dot_1*cos(2.0*theta2 + theta3 + theta4 + theta5) + 0.25*I_xy_4*theta_dot_1*cos(2*theta2 + 2*theta3 + 2*theta4) - 0.5*I_xy_5*theta_dot_1*cos(2*theta3 + 2*theta4 + 2*theta5) - 0.25*I_yz_5*theta_dot_1*sin(theta3 - 2.0*theta2 + theta4 + theta5) + 0.25*I_yz_5*theta_dot_1*sin(2.0*theta2 + theta3 + theta4 + theta5) + 0.125*I_xx_4*theta_dot_1*sin(2*theta2 + 2*theta3 + 2*theta4) - 0.25*I_xx_5*theta_dot_1*sin(2*theta3 + 2*theta4 + 2*theta5) - 0.125*I_yy_4*theta_dot_1*sin(2*theta2 + 2*theta3 + 2*theta4) + 0.25*I_yy_5*theta_dot_1*sin(2*theta3 + 2*theta4 + 2*theta5) - 0.25*I_xx_4*theta_dot_2*cos(theta2 + 2.0*theta3 + 2.0*theta4) + 0.25*I_yy_4*theta_dot_2*cos(theta2 + 2.0*theta3 + 2.0*theta4) + 0.5*I_xy_4*theta_dot_1*cos(2*theta3 + 2*theta4) + 0.5*I_xy_4*theta_dot_2*sin(theta2 + 2.0*theta3 + 2.0*theta4) + 0.25*I_xx_5*theta_dot_2*cos(theta2 + 2.0*theta3 + 2.0*theta4 + 2.0*theta5) - 0.25*I_yy_5*theta_dot_2*cos(theta2 + 2.0*theta3 + 2.0*theta4 + 2.0*theta5) + 0.25*I_xx_4*theta_dot_1*sin(2*theta3 + 2*theta4) - 0.25*I_yy_4*theta_dot_1*sin(2*theta3 + 2*theta4) + 0.5*I_xz_4*theta_dot_3*cos(theta3 - theta2 + theta4) + 0.5*I_xz_4*theta_dot_4*cos(theta3 - theta2 + theta4) - 0.5*I_xy_5*theta_dot_2*sin(theta2 + 2.0*theta3 + 2.0*theta4 + 2.0*theta5) - 0.5*I_yz_4*theta_dot_3*sin(theta3 - theta2 + theta4) - 0.5*I_yz_4*theta_dot_4*sin(theta3 - theta2 + theta4) + 0.5*I_yz_5*theta_dot_3*cos(theta2 + theta3 + theta4 + theta5) + 0.5*I_yz_5*theta_dot_4*cos(theta2 + theta3 + theta4 + theta5) + 0.5*I_yz_5*theta_dot_5*cos(theta2 + theta3 + theta4 + theta5) + 0.5*I_xz_5*theta_dot_3*sin(theta2 + theta3 + theta4 + theta5) + 0.5*I_xz_5*theta_dot_4*sin(theta2 + theta3 + theta4 + theta5) + 0.5*I_xz_5*theta_dot_5*sin(theta2 + theta3 + theta4 + theta5) - 0.25*I_xx_4*theta_dot_2*cos(2.0*theta3 - theta2 + 2.0*theta4) + 0.25*I_xy_4*theta_dot_1*cos(2.0*theta3 - 2*theta2 + 2.0*theta4) + 0.25*I_yy_4*theta_dot_2*cos(2.0*theta3 - theta2 + 2.0*theta4) - 0.25*I_yz_4*theta_dot_1*cos(theta3 - 2.0*theta2 + theta4) + 0.25*I_yz_4*theta_dot_1*cos(2.0*theta2 + theta3 + theta4) + 0.125*I_xx_4*theta_dot_1*sin(2.0*theta3 - 2*theta2 + 2.0*theta4) + 0.5*I_xy_4*theta_dot_2*sin(2.0*theta3 - theta2 + 2.0*theta4) - 0.125*I_yy_4*theta_dot_1*sin(2.0*theta3 - 2*theta2 + 2.0*theta4) - 0.25*I_xz_4*theta_dot_1*sin(theta3 - 2.0*theta2 + theta4) + 0.25*I_xz_4*theta_dot_1*sin(2.0*theta2 + theta3 + theta4) + 0.25*I_xx_5*theta_dot_2*cos(2.0*theta3 - theta2 + 2.0*theta4 + 2.0*theta5) - 0.25*I_xy_5*theta_dot_1*cos(2.0*theta3 - 2*theta2 + 2.0*theta4 + 2.0*theta5) - 0.25*I_yy_5*theta_dot_2*cos(2.0*theta3 - theta2 + 2.0*theta4 + 2.0*theta5) + 0.5*I_zz_4*theta_dot_2*cos(theta2) + 0.5*I_zz_5*theta_dot_2*cos(theta2) - 0.125*I_xx_5*theta_dot_1*sin(2.0*theta3 - 2*theta2 + 2.0*theta4 + 2.0*theta5) - 0.5*I_xy_5*theta_dot_2*sin(2.0*theta3 - theta2 + 2.0*theta4 + 2.0*theta5) + 0.125*I_yy_5*theta_dot_1*sin(2.0*theta3 - 2*theta2 + 2.0*theta4 + 2.0*theta5) + 0.03125*a5^2*m5*theta_dot_1*sin(2*theta2 + 2*theta3 + 2*theta4 + 2*theta5) + 0.125*lc5_1^2*m5*theta_dot_1*sin(2*theta2 + 2*theta3 + 2*theta4 + 2*theta5) - 0.125*lc5_2^2*m5*theta_dot_1*sin(2*theta2 + 2*theta3 + 2*theta4 + 2*theta5) - 0.03125*a4^2*m4*theta_dot_1*sin(2*theta2 + 2*theta3 + 2*theta4) - 0.125*a4^2*m5*theta_dot_1*sin(2*theta2 + 2*theta3 + 2*theta4) + 0.0625*a5^2*m5*theta_dot_1*sin(2*theta3 + 2*theta4 + 2*theta5) - 0.125*lc4_1^2*m4*theta_dot_1*sin(2*theta2 + 2*theta3 + 2*theta4) + 0.125*lc4_2^2*m4*theta_dot_1*sin(2*theta2 + 2*theta3 + 2*theta4) + 0.25*lc5_1^2*m5*theta_dot_1*sin(2*theta3 + 2*theta4 + 2*theta5) - 0.25*lc5_2^2*m5*theta_dot_1*sin(2*theta3 + 2*theta4 + 2*theta5) + 0.0625*a4^2*m4*theta_dot_2*cos(theta2 + 2.0*theta3 + 2.0*theta4) + 0.25*a4^2*m5*theta_dot_2*cos(theta2 + 2.0*theta3 + 2.0*theta4) + 0.25*lc4_1^2*m4*theta_dot_2*cos(theta2 + 2.0*theta3 + 2.0*theta4) - 0.25*lc4_2^2*m4*theta_dot_2*cos(theta2 + 2.0*theta3 + 2.0*theta4) - 0.0625*a5^2*m5*theta_dot_2*cos(theta2 + 2.0*theta3 + 2.0*theta4 + 2.0*theta5) - 0.0625*a4^2*m4*theta_dot_1*sin(2*theta3 + 2*theta4) - 0.25*a4^2*m5*theta_dot_1*sin(2*theta3 + 2*theta4) - 0.25*lc5_1^2*m5*theta_dot_2*cos(theta2 + 2.0*theta3 + 2.0*theta4 + 2.0*theta5) + 0.25*lc5_2^2*m5*theta_dot_2*cos(theta2 + 2.0*theta3 + 2.0*theta4 + 2.0*theta5) - 0.25*lc4_1^2*m4*theta_dot_1*sin(2*theta3 + 2*theta4) + 0.25*lc4_2^2*m4*theta_dot_1*sin(2*theta3 + 2*theta4) + 0.0625*a4^2*m4*theta_dot_2*cos(2.0*theta3 - theta2 + 2.0*theta4) + 0.25*a4^2*m5*theta_dot_2*cos(2.0*theta3 - theta2 + 2.0*theta4) + 0.25*lc4_1^2*m4*theta_dot_2*cos(2.0*theta3 - theta2 + 2.0*theta4) - 0.25*lc4_2^2*m4*theta_dot_2*cos(2.0*theta3 - theta2 + 2.0*theta4) - 0.03125*a4^2*m4*theta_dot_1*sin(2.0*theta3 - 2*theta2 + 2.0*theta4) - 0.125*a4^2*m5*theta_dot_1*sin(2.0*theta3 - 2*theta2 + 2.0*theta4) - 0.0625*a5^2*m5*theta_dot_2*cos(2.0*theta3 - theta2 + 2.0*theta4 + 2.0*theta5) + 0.125*a4^2*m4*theta_dot_2*cos(theta2) + 0.5*a4^2*m5*theta_dot_2*cos(theta2) + 0.125*a5^2*m5*theta_dot_2*cos(theta2) - 0.125*lc4_1^2*m4*theta_dot_1*sin(2.0*theta3 - 2*theta2 + 2.0*theta4) + 0.125*lc4_2^2*m4*theta_dot_1*sin(2.0*theta3 - 2*theta2 + 2.0*theta4) - 0.25*lc5_1^2*m5*theta_dot_2*cos(2.0*theta3 - theta2 + 2.0*theta4 + 2.0*theta5) + 0.25*lc5_2^2*m5*theta_dot_2*cos(2.0*theta3 - theta2 + 2.0*theta4 + 2.0*theta5) + 0.03125*a5^2*m5*theta_dot_1*sin(2.0*theta3 - 2*theta2 + 2.0*theta4 + 2.0*theta5) + 0.5*lc4_1^2*m4*theta_dot_2*cos(theta2) + 0.5*lc4_2^2*m4*theta_dot_2*cos(theta2) + 0.5*lc5_1^2*m5*theta_dot_2*cos(theta2) + 0.5*lc5_2^2*m5*theta_dot_2*cos(theta2) + 0.125*lc5_1^2*m5*theta_dot_1*sin(2.0*theta3 - 2*theta2 + 2.0*theta4 + 2.0*theta5) - 0.125*lc5_2^2*m5*theta_dot_1*sin(2.0*theta3 - 2*theta2 + 2.0*theta4 + 2.0*theta5) - 0.5*a1*lc5_1*m5*theta_dot_1*cos(theta3 - theta2 + theta4 + theta5) - 0.5*a2*lc5_1*m5*theta_dot_3*cos(theta3 - theta2 + theta4 + theta5) - 0.5*a2*lc5_1*m5*theta_dot_4*cos(theta3 - theta2 + theta4 + theta5) - 0.5*a2*lc5_1*m5*theta_dot_5*cos(theta3 - theta2 + theta4 + theta5) - 0.125*a3*lc4_1*m4*theta_dot_1*sin(2.0*theta2 - 1.0*theta4) - 0.5*lc5_2*lc5_3*m5*theta_dot_3*cos(theta3 - theta2 + theta4 + theta5) - 0.5*lc5_2*lc5_3*m5*theta_dot_4*cos(theta3 - theta2 + theta4 + theta5) - 0.5*lc5_2*lc5_3*m5*theta_dot_5*cos(theta3 - theta2 + theta4 + theta5) + 0.5*a1*lc5_2*m5*theta_dot_1*sin(theta3 - theta2 + theta4 + theta5) + 0.5*a2*lc5_2*m5*theta_dot_3*sin(theta3 - theta2 + theta4 + theta5) + 0.5*a2*lc5_2*m5*theta_dot_4*sin(theta3 - theta2 + theta4 + theta5) + 0.5*a2*lc5_2*m5*theta_dot_5*sin(theta3 - theta2 + theta4 + theta5) - 0.25*a5*lc5_3*m5*theta_dot_3*sin(theta3 - theta2 + theta4 + theta5) - 0.25*a5*lc5_3*m5*theta_dot_4*sin(theta3 - theta2 + theta4 + theta5) - 0.25*a5*lc5_3*m5*theta_dot_5*sin(theta3 - theta2 + theta4 + theta5) - 0.5*lc5_1*lc5_3*m5*theta_dot_3*sin(theta3 - theta2 + theta4 + theta5) - 0.5*lc5_1*lc5_3*m5*theta_dot_4*sin(theta3 - theta2 + theta4 + theta5) - 0.5*lc5_1*lc5_3*m5*theta_dot_5*sin(theta3 - theta2 + theta4 + theta5) + 0.125*a5*lc5_2*m5*theta_dot_1*cos(2*theta2 + 2*theta3 + 2*theta4 + 2*theta5) + 0.125*a3*a4*m4*theta_dot_2*cos(2.0*theta3 - theta2 + theta4) + 0.25*a3*a4*m5*theta_dot_2*cos(2.0*theta3 - theta2 + theta4) + 0.25*lc5_1*lc5_2*m5*theta_dot_1*cos(2*theta2 + 2*theta3 + 2*theta4 + 2*theta5) + 0.25*a3*lc4_1*m4*theta_dot_2*cos(2.0*theta3 - theta2 + theta4) - 0.5*a1*lc4_2*m4*theta_dot_1*cos(theta2 + theta3 + theta4) - 0.5*a2*lc4_2*m4*theta_dot_3*cos(theta2 + theta3 + theta4) - 0.5*a2*lc4_2*m4*theta_dot_4*cos(theta2 + theta3 + theta4) - 0.25*a4*lc4_3*m4*theta_dot_3*cos(theta2 + theta3 + theta4) - 0.25*a4*lc4_3*m4*theta_dot_4*cos(theta2 + theta3 + theta4) - 0.5*a2*lc5_2*m5*theta_dot_1*cos(theta3 + theta4 + theta5) - 1.0*a1*lc5_2*m5*theta_dot_3*cos(theta3 + theta4 + theta5) + 0.25*a3*lc5_2*m5*theta_dot_2*cos(theta2 + theta4 + theta5) - 1.0*a1*lc5_2*m5*theta_dot_4*cos(theta3 + theta4 + theta5) + 0.5*a3*lc5_2*m5*theta_dot_3*cos(theta2 + theta4 + theta5) - 0.5*a4*lc5_3*m5*theta_dot_3*cos(theta2 + theta3 + theta4) - 1.0*a1*lc5_2*m5*theta_dot_5*cos(theta3 + theta4 + theta5) + 0.5*a3*lc5_2*m5*theta_dot_4*cos(theta2 + theta4 + theta5) - 0.5*a4*lc5_3*m5*theta_dot_4*cos(theta2 + theta3 + theta4) + 0.5*a3*lc5_2*m5*theta_dot_5*cos(theta2 + theta4 + theta5) + 0.125*a5*lc5_1*m5*theta_dot_1*sin(2*theta2 + 2*theta3 + 2*theta4 + 2*theta5) - 0.25*a1*a4*m4*theta_dot_1*sin(theta2 + theta3 + theta4) - 0.5*a1*a4*m5*theta_dot_1*sin(theta2 + theta3 + theta4) - 0.25*a2*a4*m4*theta_dot_3*sin(theta2 + theta3 + theta4) - 0.25*a2*a4*m4*theta_dot_4*sin(theta2 + theta3 + theta4) - 0.5*a2*a4*m5*theta_dot_3*sin(theta2 + theta3 + theta4) - 0.5*a2*a4*m5*theta_dot_4*sin(theta2 + theta3 + theta4) - 0.25*a2*a5*m5*theta_dot_1*sin(theta3 + theta4 + theta5) - 0.5*a1*a5*m5*theta_dot_3*sin(theta3 + theta4 + theta5) + 0.125*a3*a5*m5*theta_dot_2*sin(theta2 + theta4 + theta5) - 0.5*a1*a5*m5*theta_dot_4*sin(theta3 + theta4 + theta5) + 0.25*a3*a5*m5*theta_dot_3*sin(theta2 + theta4 + theta5) - 0.5*a1*a5*m5*theta_dot_5*sin(theta3 + theta4 + theta5) + 0.25*a3*a5*m5*theta_dot_4*sin(theta2 + theta4 + theta5) + 0.25*a3*a5*m5*theta_dot_5*sin(theta2 + theta4 + theta5) - 0.5*lc4_1*lc4_3*m4*theta_dot_3*cos(theta2 + theta3 + theta4) - 0.5*lc4_1*lc4_3*m4*theta_dot_4*cos(theta2 + theta3 + theta4) - 0.25*a3*lc4_2*m4*theta_dot_2*sin(2.0*theta3 - theta2 + theta4) - 0.5*a1*lc4_1*m4*theta_dot_1*sin(theta2 + theta3 + theta4) - 0.5*a2*lc4_1*m4*theta_dot_3*sin(theta2 + theta3 + theta4) - 0.5*a2*lc4_1*m4*theta_dot_4*sin(theta2 + theta3 + theta4) - 0.5*a2*lc5_1*m5*theta_dot_1*sin(theta3 + theta4 + theta5) - 1.0*a1*lc5_1*m5*theta_dot_3*sin(theta3 + theta4 + theta5) + 0.25*a3*lc5_1*m5*theta_dot_2*sin(theta2 + theta4 + theta5) - 1.0*a1*lc5_1*m5*theta_dot_4*sin(theta3 + theta4 + theta5) + 0.5*a3*lc5_1*m5*theta_dot_3*sin(theta2 + theta4 + theta5) - 1.0*a1*lc5_1*m5*theta_dot_5*sin(theta3 + theta4 + theta5) + 0.5*a3*lc5_1*m5*theta_dot_4*sin(theta2 + theta4 + theta5) + 0.5*a3*lc5_1*m5*theta_dot_5*sin(theta2 + theta4 + theta5) + 0.5*a4*lc5_2*m5*theta_dot_2*cos(2.0*theta3 - theta2 + 2.0*theta4 + theta5) + 0.25*a2*lc5_2*m5*theta_dot_1*cos(theta3 - 2.0*theta2 + theta4 + theta5) + 0.25*a2*lc5_2*m5*theta_dot_1*cos(2.0*theta2 + theta3 + theta4 + theta5) + 0.25*a3*lc5_2*m5*theta_dot_2*cos(theta2 + 2.0*theta3 + theta4 + theta5) - 0.125*a5*lc5_3*m5*theta_dot_1*cos(theta3 - 2.0*theta2 + theta4 + theta5) + 0.125*a5*lc5_3*m5*theta_dot_1*cos(2.0*theta2 + theta3 + theta4 + theta5) + 0.25*a4*a5*m5*theta_dot_2*sin(2.0*theta3 - theta2 + 2.0*theta4 + theta5) + 0.125*a2*a5*m5*theta_dot_1*sin(theta3 - 2.0*theta2 + theta4 + theta5) + 0.125*a2*a5*m5*theta_dot_1*sin(2.0*theta2 + theta3 + theta4 + theta5) + 0.125*a3*a5*m5*theta_dot_2*sin(theta2 + 2.0*theta3 + theta4 + theta5) + 0.5*lc4_2*lc4_3*m4*theta_dot_3*sin(theta2 + theta3 + theta4) + 0.5*lc4_2*lc4_3*m4*theta_dot_4*sin(theta2 + theta3 + theta4) - 0.125*a4*lc4_2*m4*theta_dot_1*cos(2*theta2 + 2*theta3 + 2*theta4) + 0.25*a5*lc5_2*m5*theta_dot_1*cos(2*theta3 + 2*theta4 + 2*theta5) - 0.25*lc5_1*lc5_3*m5*theta_dot_1*cos(theta3 - 2.0*theta2 + theta4 + theta5) + 0.25*lc5_1*lc5_3*m5*theta_dot_1*cos(2.0*theta2 + theta3 + theta4 + theta5) + 0.125*a3*a4*m4*theta_dot_2*cos(theta2 - 1.0*theta4) - 0.25*a3*a4*m4*theta_dot_3*cos(theta2 - 1.0*theta4) + 0.25*a3*a4*m5*theta_dot_2*cos(theta2 - 1.0*theta4) - 0.25*a3*a4*m4*theta_dot_4*cos(theta2 - 1.0*theta4) - 0.5*a3*a4*m5*theta_dot_3*cos(theta2 - 1.0*theta4) - 0.5*a3*a4*m5*theta_dot_4*cos(theta2 - 1.0*theta4) + 0.5*a4*lc5_1*m5*theta_dot_2*sin(2.0*theta3 - theta2 + 2.0*theta4 + theta5) + 0.25*a2*lc5_1*m5*theta_dot_1*sin(theta3 - 2.0*theta2 + theta4 + theta5) + 0.25*a2*lc5_1*m5*theta_dot_1*sin(2.0*theta2 + theta3 + theta4 + theta5) + 0.25*a3*lc5_1*m5*theta_dot_2*sin(theta2 + 2.0*theta3 + theta4 + theta5) - 0.25*lc4_1*lc4_2*m4*theta_dot_1*cos(2*theta2 + 2*theta3 + 2*theta4) + 0.5*lc5_1*lc5_2*m5*theta_dot_1*cos(2*theta3 + 2*theta4 + 2*theta5) + 0.25*a3*lc4_1*m4*theta_dot_2*cos(theta2 - 1.0*theta4) - 0.5*a3*lc4_1*m4*theta_dot_3*cos(theta2 - 1.0*theta4) + 0.125*a3*lc4_2*m4*theta_dot_1*cos(2.0*theta2 + theta4) - 0.5*a3*lc4_1*m4*theta_dot_4*cos(theta2 - 1.0*theta4) - 0.25*a3*lc4_2*m4*theta_dot_1*cos(2.0*theta3 + theta4) + 0.5*a4*lc5_2*m5*theta_dot_2*cos(theta2 - 1.0*theta5) - 0.5*a4*lc5_2*m5*theta_dot_5*cos(theta2 - 1.0*theta5) - 0.125*a4*lc4_1*m4*theta_dot_1*sin(2*theta2 + 2*theta3 + 2*theta4) + 0.25*a5*lc5_1*m5*theta_dot_1*sin(2*theta3 + 2*theta4 + 2*theta5) + 0.25*lc5_2*lc5_3*m5*theta_dot_1*sin(theta3 - 2.0*theta2 + theta4 + theta5) - 0.25*lc5_2*lc5_3*m5*theta_dot_1*sin(2.0*theta2 + theta3 + theta4 + theta5) + 0.0625*a3*a4*m4*theta_dot_1*sin(2.0*theta2 + theta4) - 0.125*a3*a4*m4*theta_dot_1*sin(2.0*theta3 + theta4) + 0.125*a3*a4*m5*theta_dot_1*sin(2.0*theta2 + theta4) - 0.25*a3*a4*m5*theta_dot_1*sin(2.0*theta3 + theta4) - 0.25*a4*a5*m5*theta_dot_2*sin(theta2 - 1.0*theta5) + 0.25*a4*a5*m5*theta_dot_5*sin(theta2 - 1.0*theta5) + 0.25*a4*a5*m5*theta_dot_1*cos(2.0*theta3 + 2.0*theta4 + theta5) + 0.125*a3*lc4_1*m4*theta_dot_1*sin(2.0*theta2 + theta4) - 0.25*a3*lc4_1*m4*theta_dot_1*sin(2.0*theta3 + theta4) + 0.25*a3*lc4_2*m4*theta_dot_2*sin(theta2 - 1.0*theta4) - 0.5*a3*lc4_2*m4*theta_dot_3*sin(theta2 - 1.0*theta4) - 0.5*a3*lc4_2*m4*theta_dot_4*sin(theta2 - 1.0*theta4) - 0.5*a4*lc5_1*m5*theta_dot_2*sin(theta2 - 1.0*theta5) + 0.5*a4*lc5_1*m5*theta_dot_5*sin(theta2 - 1.0*theta5) - 0.125*a3*lc4_2*m4*theta_dot_1*cos(2.0*theta3 - 2.0*theta2 + theta4) - 0.125*a3*lc4_2*m4*theta_dot_1*cos(2.0*theta2 + 2.0*theta3 + theta4) + 0.25*a4*lc4_1*m4*theta_dot_2*cos(theta2 + 2.0*theta3 + 2.0*theta4) + 0.5*a4*lc5_1*m5*theta_dot_1*cos(2.0*theta3 + 2.0*theta4 + theta5) - 0.0625*a3*a4*m4*theta_dot_1*sin(2.0*theta3 - 2.0*theta2 + theta4) - 0.0625*a3*a4*m4*theta_dot_1*sin(2.0*theta2 + 2.0*theta3 + theta4) - 0.125*a3*a4*m5*theta_dot_1*sin(2.0*theta3 - 2.0*theta2 + theta4) - 0.125*a3*a4*m5*theta_dot_1*sin(2.0*theta2 + 2.0*theta3 + theta4) + 0.125*a4*a5*m5*theta_dot_1*cos(2.0*theta3 - 2.0*theta2 + 2.0*theta4 + theta5) + 0.125*a4*a5*m5*theta_dot_1*cos(2.0*theta2 + 2.0*theta3 + 2.0*theta4 + theta5) - 0.25*a4*lc4_2*m4*theta_dot_1*cos(2*theta3 + 2*theta4) - 0.125*a3*lc4_1*m4*theta_dot_1*sin(2.0*theta3 - 2.0*theta2 + theta4) - 0.125*a3*lc4_1*m4*theta_dot_1*sin(2.0*theta2 + 2.0*theta3 + theta4) - 0.25*a4*lc4_2*m4*theta_dot_2*sin(theta2 + 2.0*theta3 + 2.0*theta4) - 0.5*a4*lc5_2*m5*theta_dot_1*sin(2.0*theta3 + 2.0*theta4 + theta5) + 0.25*a4*lc5_1*m5*theta_dot_1*cos(2.0*theta3 - 2.0*theta2 + 2.0*theta4 + theta5) + 0.25*a4*lc5_1*m5*theta_dot_1*cos(2.0*theta2 + 2.0*theta3 + 2.0*theta4 + theta5) - 0.25*a5*lc5_1*m5*theta_dot_2*cos(theta2 + 2.0*theta3 + 2.0*theta4 + 2.0*theta5) - 0.5*lc4_1*lc4_2*m4*theta_dot_1*cos(2*theta3 + 2*theta4) - 0.5*lc4_1*lc4_2*m4*theta_dot_2*sin(theta2 + 2.0*theta3 + 2.0*theta4) - 0.25*a4*lc4_1*m4*theta_dot_1*sin(2*theta3 + 2*theta4) + 0.5*a1*lc4_2*m4*theta_dot_1*cos(theta3 - theta2 + theta4) + 0.5*a2*lc4_2*m4*theta_dot_3*cos(theta3 - theta2 + theta4) + 0.5*a2*lc4_2*m4*theta_dot_4*cos(theta3 - theta2 + theta4) - 0.25*a4*lc4_3*m4*theta_dot_3*cos(theta3 - theta2 + theta4) - 0.25*a4*lc4_3*m4*theta_dot_4*cos(theta3 - theta2 + theta4) + 0.25*a3*lc5_2*m5*theta_dot_2*cos(theta4 - theta2 + theta5) - 0.5*a3*lc5_2*m5*theta_dot_3*cos(theta4 - theta2 + theta5) - 0.5*a4*lc5_3*m5*theta_dot_3*cos(theta3 - theta2 + theta4) - 0.5*a3*lc5_2*m5*theta_dot_4*cos(theta4 - theta2 + theta5) - 0.5*a4*lc5_3*m5*theta_dot_4*cos(theta3 - theta2 + theta4) - 0.5*a3*lc5_2*m5*theta_dot_5*cos(theta4 - theta2 + theta5) - 0.25*a4*lc5_2*m5*theta_dot_1*sin(2.0*theta3 - 2.0*theta2 + 2.0*theta4 + theta5) - 0.25*a4*lc5_2*m5*theta_dot_1*sin(2.0*theta2 + 2.0*theta3 + 2.0*theta4 + theta5) + 0.25*a5*lc5_2*m5*theta_dot_2*sin(theta2 + 2.0*theta3 + 2.0*theta4 + 2.0*theta5) + 0.25*a1*a4*m4*theta_dot_1*sin(theta3 - theta2 + theta4) + 0.5*a1*a4*m5*theta_dot_1*sin(theta3 - theta2 + theta4) + 0.25*a2*a4*m4*theta_dot_3*sin(theta3 - theta2 + theta4) + 0.25*a2*a4*m4*theta_dot_4*sin(theta3 - theta2 + theta4) + 0.5*a2*a4*m5*theta_dot_3*sin(theta3 - theta2 + theta4) + 0.5*a2*a4*m5*theta_dot_4*sin(theta3 - theta2 + theta4) + 0.125*a3*a5*m5*theta_dot_2*sin(theta4 - theta2 + theta5) - 0.25*a3*a5*m5*theta_dot_3*sin(theta4 - theta2 + theta5) - 0.25*a3*a5*m5*theta_dot_4*sin(theta4 - theta2 + theta5) - 0.25*a3*a5*m5*theta_dot_5*sin(theta4 - theta2 + theta5) + 0.25*a1*a5*m5*theta_dot_1*cos(theta2 + theta3 + theta4 + theta5) + 0.25*a2*a5*m5*theta_dot_3*cos(theta2 + theta3 + theta4 + theta5) + 0.25*a2*a5*m5*theta_dot_4*cos(theta2 + theta3 + theta4 + theta5) + 0.25*a2*a5*m5*theta_dot_5*cos(theta2 + theta3 + theta4 + theta5) - 0.5*lc4_1*lc4_3*m4*theta_dot_3*cos(theta3 - theta2 + theta4) - 0.5*lc4_1*lc4_3*m4*theta_dot_4*cos(theta3 - theta2 + theta4) + 0.5*lc5_1*lc5_2*m5*theta_dot_2*sin(theta2 + 2.0*theta3 + 2.0*theta4 + 2.0*theta5) + 0.5*a1*lc4_1*m4*theta_dot_1*sin(theta3 - theta2 + theta4) + 0.5*a2*lc4_1*m4*theta_dot_3*sin(theta3 - theta2 + theta4) + 0.5*a2*lc4_1*m4*theta_dot_4*sin(theta3 - theta2 + theta4) + 0.25*a3*lc5_1*m5*theta_dot_2*sin(theta4 - theta2 + theta5) - 0.5*a3*lc5_1*m5*theta_dot_3*sin(theta4 - theta2 + theta5) - 0.5*a3*lc5_1*m5*theta_dot_4*sin(theta4 - theta2 + theta5) - 0.5*a3*lc5_1*m5*theta_dot_5*sin(theta4 - theta2 + theta5) + 0.25*a3*lc5_2*m5*theta_dot_2*cos(2.0*theta3 - theta2 + theta4 + theta5) + 0.5*a1*lc5_1*m5*theta_dot_1*cos(theta2 + theta3 + theta4 + theta5) + 0.5*a2*lc5_1*m5*theta_dot_3*cos(theta2 + theta3 + theta4 + theta5) + 0.5*a2*lc5_1*m5*theta_dot_4*cos(theta2 + theta3 + theta4 + theta5) + 0.5*a2*lc5_1*m5*theta_dot_5*cos(theta2 + theta3 + theta4 + theta5) + 0.125*a3*a5*m5*theta_dot_2*sin(2.0*theta3 - theta2 + theta4 + theta5) + 0.5*lc4_2*lc4_3*m4*theta_dot_3*sin(theta3 - theta2 + theta4) + 0.5*lc4_2*lc4_3*m4*theta_dot_4*sin(theta3 - theta2 + theta4) - 0.5*lc5_2*lc5_3*m5*theta_dot_3*cos(theta2 + theta3 + theta4 + theta5) - 0.5*lc5_2*lc5_3*m5*theta_dot_4*cos(theta2 + theta3 + theta4 + theta5) - 0.5*lc5_2*lc5_3*m5*theta_dot_5*cos(theta2 + theta3 + theta4 + theta5) - 0.25*a2*a4*m4*theta_dot_1*cos(theta3 + theta4) - 0.5*a1*a4*m4*theta_dot_3*cos(theta3 + theta4) - 0.5*a2*a4*m5*theta_dot_1*cos(theta3 + theta4) + 0.125*a3*a4*m4*theta_dot_2*cos(theta2 + theta4) - 0.5*a1*a4*m4*theta_dot_4*cos(theta3 + theta4) - 1.0*a1*a4*m5*theta_dot_3*cos(theta3 + theta4) + 0.25*a3*a4*m4*theta_dot_3*cos(theta2 + theta4) + 0.25*a3*a4*m5*theta_dot_2*cos(theta2 + theta4) - 1.0*a1*a4*m5*theta_dot_4*cos(theta3 + theta4) + 0.25*a3*a4*m4*theta_dot_4*cos(theta2 + theta4) + 0.5*a3*a4*m5*theta_dot_3*cos(theta2 + theta4) + 0.5*a3*a4*m5*theta_dot_4*cos(theta2 + theta4) + 0.375*a3*a5*m5*theta_dot_1*cos(theta4 + theta5) + 0.25*a3*lc5_1*m5*theta_dot_2*sin(2.0*theta3 - theta2 + theta4 + theta5) - 0.5*a1*lc5_2*m5*theta_dot_1*sin(theta2 + theta3 + theta4 + theta5) - 0.5*a2*lc5_2*m5*theta_dot_3*sin(theta2 + theta3 + theta4 + theta5) - 0.5*a2*lc5_2*m5*theta_dot_4*sin(theta2 + theta3 + theta4 + theta5) - 0.5*a2*lc5_2*m5*theta_dot_5*sin(theta2 + theta3 + theta4 + theta5) - 0.25*a5*lc5_3*m5*theta_dot_3*sin(theta2 + theta3 + theta4 + theta5) - 0.25*a5*lc5_3*m5*theta_dot_4*sin(theta2 + theta3 + theta4 + theta5) - 0.25*a5*lc5_3*m5*theta_dot_5*sin(theta2 + theta3 + theta4 + theta5) - 0.5*a2*lc4_1*m4*theta_dot_1*cos(theta3 + theta4) - 1.0*a1*lc4_1*m4*theta_dot_3*cos(theta3 + theta4) + 0.25*a3*lc4_1*m4*theta_dot_2*cos(theta2 + theta4) - 1.0*a1*lc4_1*m4*theta_dot_4*cos(theta3 + theta4) + 0.5*a3*lc4_1*m4*theta_dot_3*cos(theta2 + theta4) + 0.5*a3*lc4_1*m4*theta_dot_4*cos(theta2 + theta4) + 0.75*a3*lc5_1*m5*theta_dot_1*cos(theta4 + theta5) + 0.5*a4*lc5_2*m5*theta_dot_2*cos(theta2 + theta5) + 0.5*a4*lc5_2*m5*theta_dot_5*cos(theta2 + theta5) - 0.5*lc5_1*lc5_3*m5*theta_dot_3*sin(theta2 + theta3 + theta4 + theta5) - 0.5*lc5_1*lc5_3*m5*theta_dot_4*sin(theta2 + theta3 + theta4 + theta5) - 0.5*lc5_1*lc5_3*m5*theta_dot_5*sin(theta2 + theta3 + theta4 + theta5) + 0.25*a4*a5*m5*theta_dot_2*sin(theta2 + theta5) + 0.25*a4*a5*m5*theta_dot_5*sin(theta2 + theta5) + 0.125*a2*a4*m4*theta_dot_1*cos(theta3 - 2.0*theta2 + theta4) + 0.125*a2*a4*m4*theta_dot_1*cos(2.0*theta2 + theta3 + theta4) + 0.25*a2*a4*m5*theta_dot_1*cos(theta3 - 2.0*theta2 + theta4) + 0.25*a2*a4*m5*theta_dot_1*cos(2.0*theta2 + theta3 + theta4) + 0.125*a3*a4*m4*theta_dot_2*cos(theta2 + 2.0*theta3 + theta4) + 0.25*a3*a4*m5*theta_dot_2*cos(theta2 + 2.0*theta3 + theta4) - 0.0625*a3*a5*m5*theta_dot_1*cos(theta4 - 2.0*theta2 + theta5) - 0.0625*a3*a5*m5*theta_dot_1*cos(2.0*theta2 + theta4 + theta5) + 0.125*a3*a5*m5*theta_dot_1*cos(2.0*theta3 + theta4 + theta5) + 0.5*a2*lc4_2*m4*theta_dot_1*sin(theta3 + theta4) + a1*lc4_2*m4*theta_dot_3*sin(theta3 + theta4) - 0.25*a3*lc4_2*m4*theta_dot_2*sin(theta2 + theta4) + a1*lc4_2*m4*theta_dot_4*sin(theta3 + theta4) - 0.5*a3*lc4_2*m4*theta_dot_3*sin(theta2 + theta4) - 0.5*a3*lc4_2*m4*theta_dot_4*sin(theta2 + theta4) + 0.5*a4*lc5_1*m5*theta_dot_2*sin(theta2 + theta5) - 0.75*a3*lc5_2*m5*theta_dot_1*sin(theta4 + theta5) + 0.5*a4*lc5_1*m5*theta_dot_5*sin(theta2 + theta5) + 0.25*a4*lc4_1*m4*theta_dot_2*cos(2.0*theta3 - theta2 + 2.0*theta4) - 0.125*a4*lc4_2*m4*theta_dot_1*cos(2.0*theta3 - 2*theta2 + 2.0*theta4) + 0.25*a2*lc4_1*m4*theta_dot_1*cos(theta3 - 2.0*theta2 + theta4) + 0.25*a2*lc4_1*m4*theta_dot_1*cos(2.0*theta2 + theta3 + theta4) + 0.25*a3*lc4_1*m4*theta_dot_2*cos(theta2 + 2.0*theta3 + theta4) - 0.125*a3*lc5_1*m5*theta_dot_1*cos(theta4 - 2.0*theta2 + theta5) - 0.125*a3*lc5_1*m5*theta_dot_1*cos(2.0*theta2 + theta4 + theta5) + 0.25*a3*lc5_1*m5*theta_dot_1*cos(2.0*theta3 + theta4 + theta5) + 0.0625*a3*a5*m5*theta_dot_1*cos(2.0*theta3 - 2.0*theta2 + theta4 + theta5) + 0.0625*a3*a5*m5*theta_dot_1*cos(2.0*theta2 + 2.0*theta3 + theta4 + theta5) - 0.25*lc4_1*lc4_2*m4*theta_dot_1*cos(2.0*theta3 - 2*theta2 + 2.0*theta4) + 0.25*lc4_2*lc4_3*m4*theta_dot_1*cos(theta3 - 2.0*theta2 + theta4) - 0.25*lc4_2*lc4_3*m4*theta_dot_1*cos(2.0*theta2 + theta3 + theta4) - 0.125*a4*lc4_1*m4*theta_dot_1*sin(2.0*theta3 - 2*theta2 + 2.0*theta4) - 0.25*a4*lc4_2*m4*theta_dot_2*sin(2.0*theta3 - theta2 + 2.0*theta4) - 0.25*a2*lc4_2*m4*theta_dot_1*sin(theta3 - 2.0*theta2 + theta4) - 0.25*a2*lc4_2*m4*theta_dot_1*sin(2.0*theta2 + theta3 + theta4) - 0.25*a3*lc4_2*m4*theta_dot_2*sin(theta2 + 2.0*theta3 + theta4) + 0.125*a4*lc4_3*m4*theta_dot_1*sin(theta3 - 2.0*theta2 + theta4) - 0.125*a4*lc4_3*m4*theta_dot_1*sin(2.0*theta2 + theta3 + theta4) + 0.125*a3*lc5_2*m5*theta_dot_1*sin(theta4 - 2.0*theta2 + theta5) + 0.125*a3*lc5_2*m5*theta_dot_1*sin(2.0*theta2 + theta4 + theta5) + 0.25*a4*lc5_3*m5*theta_dot_1*sin(theta3 - 2.0*theta2 + theta4) - 0.25*a4*lc5_3*m5*theta_dot_1*sin(2.0*theta2 + theta3 + theta4) - 0.25*a3*lc5_2*m5*theta_dot_1*sin(2.0*theta3 + theta4 + theta5) - 0.25*a5*lc5_1*m5*theta_dot_2*cos(2.0*theta3 - theta2 + 2.0*theta4 + 2.0*theta5) + 0.125*a5*lc5_2*m5*theta_dot_1*cos(2.0*theta3 - 2*theta2 + 2.0*theta4 + 2.0*theta5) + 0.125*a3*lc5_1*m5*theta_dot_1*cos(2.0*theta3 - 2.0*theta2 + theta4 + theta5) + 0.125*a3*lc5_1*m5*theta_dot_1*cos(2.0*theta2 + 2.0*theta3 + theta4 + theta5) + 0.5*a4*lc5_2*m5*theta_dot_2*cos(theta2 + 2.0*theta3 + 2.0*theta4 + theta5) + 0.5*a4*lc4_1*m4*theta_dot_2*cos(theta2) - 0.75*a3*lc4_2*m4*theta_dot_1*cos(theta4) + 0.5*a5*lc5_1*m5*theta_dot_2*cos(theta2) + 0.25*a4*a5*m5*theta_dot_2*sin(theta2 + 2.0*theta3 + 2.0*theta4 + theta5) - 0.5*lc4_1*lc4_2*m4*theta_dot_2*sin(2.0*theta3 - theta2 + 2.0*theta4) + 0.25*lc4_1*lc4_3*m4*theta_dot_1*sin(theta3 - 2.0*theta2 + theta4) - 0.25*lc4_1*lc4_3*m4*theta_dot_1*sin(2.0*theta2 + theta3 + theta4) - 0.375*a3*a4*m4*theta_dot_1*sin(theta4) - 0.75*a3*a4*m5*theta_dot_1*sin(theta4) + 0.25*lc5_1*lc5_2*m5*theta_dot_1*cos(2.0*theta3 - 2*theta2 + 2.0*theta4 + 2.0*theta5) + 0.125*a5*lc5_1*m5*theta_dot_1*sin(2.0*theta3 - 2*theta2 + 2.0*theta4 + 2.0*theta5) + 0.25*a5*lc5_2*m5*theta_dot_2*sin(2.0*theta3 - theta2 + 2.0*theta4 + 2.0*theta5) - 0.125*a3*lc5_2*m5*theta_dot_1*sin(2.0*theta3 - 2.0*theta2 + theta4 + theta5) - 0.125*a3*lc5_2*m5*theta_dot_1*sin(2.0*theta2 + 2.0*theta3 + theta4 + theta5) + 0.5*a4*lc5_1*m5*theta_dot_2*sin(theta2 + 2.0*theta3 + 2.0*theta4 + theta5) - 0.75*a3*lc4_1*m4*theta_dot_1*sin(theta4) - 0.25*a1*a5*m5*theta_dot_1*cos(theta3 - theta2 + theta4 + theta5) - 0.25*a2*a5*m5*theta_dot_3*cos(theta3 - theta2 + theta4 + theta5) - 0.25*a2*a5*m5*theta_dot_4*cos(theta3 - theta2 + theta4 + theta5) - 0.25*a2*a5*m5*theta_dot_5*cos(theta3 - theta2 + theta4 + theta5) + 0.125*a3*lc4_2*m4*theta_dot_1*cos(2.0*theta2 - 1.0*theta4) + 0.5*lc5_1*lc5_2*m5*theta_dot_2*sin(2.0*theta3 - theta2 + 2.0*theta4 + 2.0*theta5) - 0.0625*a3*a4*m4*theta_dot_1*sin(2.0*theta2 - 1.0*theta4) - 0.125*a3*a4*m5*theta_dot_1*sin(2.0*theta2 - 1.0*theta4)
C15 = 0.5*I_yz_5*theta_dot_3*cos(theta3 - theta2 + theta4 + theta5) + 0.5*I_yz_5*theta_dot_4*cos(theta3 - theta2 + theta4 + theta5) + 0.5*I_yz_5*theta_dot_5*cos(theta3 - theta2 + theta4 + theta5) + 0.5*I_xz_5*theta_dot_3*sin(theta3 - theta2 + theta4 + theta5) + 0.5*I_xz_5*theta_dot_4*sin(theta3 - theta2 + theta4 + theta5) + 0.5*I_xz_5*theta_dot_5*sin(theta3 - theta2 + theta4 + theta5) - 0.25*I_xy_5*theta_dot_1*cos(2*theta2 + 2*theta3 + 2*theta4 + 2*theta5) - 0.125*I_xx_5*theta_dot_1*sin(2*theta2 + 2*theta3 + 2*theta4 + 2*theta5) + 0.125*I_yy_5*theta_dot_1*sin(2*theta2 + 2*theta3 + 2*theta4 + 2*theta5) + 0.25*I_xz_5*theta_dot_1*cos(theta3 - 2.0*theta2 + theta4 + theta5) - 0.25*I_xz_5*theta_dot_1*cos(2.0*theta2 + theta3 + theta4 + theta5) - 0.5*I_xy_5*theta_dot_1*cos(2*theta3 + 2*theta4 + 2*theta5) - 0.25*I_yz_5*theta_dot_1*sin(theta3 - 2.0*theta2 + theta4 + theta5) + 0.25*I_yz_5*theta_dot_1*sin(2.0*theta2 + theta3 + theta4 + theta5) - 0.25*I_xx_5*theta_dot_1*sin(2*theta3 + 2*theta4 + 2*theta5) + 0.25*I_yy_5*theta_dot_1*sin(2*theta3 + 2*theta4 + 2*theta5) + 0.25*I_xx_5*theta_dot_2*cos(theta2 + 2.0*theta3 + 2.0*theta4 + 2.0*theta5) - 0.25*I_yy_5*theta_dot_2*cos(theta2 + 2.0*theta3 + 2.0*theta4 + 2.0*theta5) - 0.5*I_xy_5*theta_dot_2*sin(theta2 + 2.0*theta3 + 2.0*theta4 + 2.0*theta5) + 0.5*I_yz_5*theta_dot_3*cos(theta2 + theta3 + theta4 + theta5) + 0.5*I_yz_5*theta_dot_4*cos(theta2 + theta3 + theta4 + theta5) + 0.5*I_yz_5*theta_dot_5*cos(theta2 + theta3 + theta4 + theta5) + 0.5*I_xz_5*theta_dot_3*sin(theta2 + theta3 + theta4 + theta5) + 0.5*I_xz_5*theta_dot_4*sin(theta2 + theta3 + theta4 + theta5) + 0.5*I_xz_5*theta_dot_5*sin(theta2 + theta3 + theta4 + theta5) + 0.25*I_xx_5*theta_dot_2*cos(2.0*theta3 - theta2 + 2.0*theta4 + 2.0*theta5) - 0.25*I_xy_5*theta_dot_1*cos(2.0*theta3 - 2*theta2 + 2.0*theta4 + 2.0*theta5) - 0.25*I_yy_5*theta_dot_2*cos(2.0*theta3 - theta2 + 2.0*theta4 + 2.0*theta5) + 0.5*I_zz_5*theta_dot_2*cos(theta2) - 0.125*I_xx_5*theta_dot_1*sin(2.0*theta3 - 2*theta2 + 2.0*theta4 + 2.0*theta5) - 0.5*I_xy_5*theta_dot_2*sin(2.0*theta3 - theta2 + 2.0*theta4 + 2.0*theta5) + 0.125*I_yy_5*theta_dot_1*sin(2.0*theta3 - 2*theta2 + 2.0*theta4 + 2.0*theta5) + 0.03125*a5^2*m5*theta_dot_1*sin(2*theta2 + 2*theta3 + 2*theta4 + 2*theta5) + 0.125*lc5_1^2*m5*theta_dot_1*sin(2*theta2 + 2*theta3 + 2*theta4 + 2*theta5) - 0.125*lc5_2^2*m5*theta_dot_1*sin(2*theta2 + 2*theta3 + 2*theta4 + 2*theta5) + 0.0625*a5^2*m5*theta_dot_1*sin(2*theta3 + 2*theta4 + 2*theta5) + 0.25*lc5_1^2*m5*theta_dot_1*sin(2*theta3 + 2*theta4 + 2*theta5) - 0.25*lc5_2^2*m5*theta_dot_1*sin(2*theta3 + 2*theta4 + 2*theta5) - 0.0625*a5^2*m5*theta_dot_2*cos(theta2 + 2.0*theta3 + 2.0*theta4 + 2.0*theta5) - 0.25*lc5_1^2*m5*theta_dot_2*cos(theta2 + 2.0*theta3 + 2.0*theta4 + 2.0*theta5) + 0.25*lc5_2^2*m5*theta_dot_2*cos(theta2 + 2.0*theta3 + 2.0*theta4 + 2.0*theta5) - 0.0625*a5^2*m5*theta_dot_2*cos(2.0*theta3 - theta2 + 2.0*theta4 + 2.0*theta5) + 0.125*a5^2*m5*theta_dot_2*cos(theta2) - 0.25*lc5_1^2*m5*theta_dot_2*cos(2.0*theta3 - theta2 + 2.0*theta4 + 2.0*theta5) + 0.25*lc5_2^2*m5*theta_dot_2*cos(2.0*theta3 - theta2 + 2.0*theta4 + 2.0*theta5) + 0.03125*a5^2*m5*theta_dot_1*sin(2.0*theta3 - 2*theta2 + 2.0*theta4 + 2.0*theta5) + 0.5*lc5_1^2*m5*theta_dot_2*cos(theta2) + 0.5*lc5_2^2*m5*theta_dot_2*cos(theta2) + 0.125*lc5_1^2*m5*theta_dot_1*sin(2.0*theta3 - 2*theta2 + 2.0*theta4 + 2.0*theta5) - 0.125*lc5_2^2*m5*theta_dot_1*sin(2.0*theta3 - 2*theta2 + 2.0*theta4 + 2.0*theta5) - 0.5*a1*lc5_1*m5*theta_dot_1*cos(theta3 - theta2 + theta4 + theta5) - 0.5*a2*lc5_1*m5*theta_dot_3*cos(theta3 - theta2 + theta4 + theta5) - 0.5*a2*lc5_1*m5*theta_dot_4*cos(theta3 - theta2 + theta4 + theta5) - 0.5*a2*lc5_1*m5*theta_dot_5*cos(theta3 - theta2 + theta4 + theta5) - 0.125*a4*lc5_2*m5*theta_dot_1*sin(2.0*theta2 - 1.0*theta5) - 0.5*lc5_2*lc5_3*m5*theta_dot_3*cos(theta3 - theta2 + theta4 + theta5) - 0.5*lc5_2*lc5_3*m5*theta_dot_4*cos(theta3 - theta2 + theta4 + theta5) - 0.5*lc5_2*lc5_3*m5*theta_dot_5*cos(theta3 - theta2 + theta4 + theta5) + 0.5*a1*lc5_2*m5*theta_dot_1*sin(theta3 - theta2 + theta4 + theta5) + 0.5*a2*lc5_2*m5*theta_dot_3*sin(theta3 - theta2 + theta4 + theta5) + 0.5*a2*lc5_2*m5*theta_dot_4*sin(theta3 - theta2 + theta4 + theta5) + 0.5*a2*lc5_2*m5*theta_dot_5*sin(theta3 - theta2 + theta4 + theta5) - 0.25*a5*lc5_3*m5*theta_dot_3*sin(theta3 - theta2 + theta4 + theta5) - 0.25*a5*lc5_3*m5*theta_dot_4*sin(theta3 - theta2 + theta4 + theta5) - 0.25*a5*lc5_3*m5*theta_dot_5*sin(theta3 - theta2 + theta4 + theta5) - 0.5*lc5_1*lc5_3*m5*theta_dot_3*sin(theta3 - theta2 + theta4 + theta5) - 0.5*lc5_1*lc5_3*m5*theta_dot_4*sin(theta3 - theta2 + theta4 + theta5) - 0.5*lc5_1*lc5_3*m5*theta_dot_5*sin(theta3 - theta2 + theta4 + theta5) + 0.125*a5*lc5_2*m5*theta_dot_1*cos(2*theta2 + 2*theta3 + 2*theta4 + 2*theta5) + 0.25*lc5_1*lc5_2*m5*theta_dot_1*cos(2*theta2 + 2*theta3 + 2*theta4 + 2*theta5) - 0.5*a2*lc5_2*m5*theta_dot_1*cos(theta3 + theta4 + theta5) - 1.0*a1*lc5_2*m5*theta_dot_3*cos(theta3 + theta4 + theta5) + 0.25*a3*lc5_2*m5*theta_dot_2*cos(theta2 + theta4 + theta5) - 1.0*a1*lc5_2*m5*theta_dot_4*cos(theta3 + theta4 + theta5) + 0.5*a3*lc5_2*m5*theta_dot_3*cos(theta2 + theta4 + theta5) - 1.0*a1*lc5_2*m5*theta_dot_5*cos(theta3 + theta4 + theta5) + 0.5*a3*lc5_2*m5*theta_dot_4*cos(theta2 + theta4 + theta5) + 0.5*a3*lc5_2*m5*theta_dot_5*cos(theta2 + theta4 + theta5) + 0.125*a5*lc5_1*m5*theta_dot_1*sin(2*theta2 + 2*theta3 + 2*theta4 + 2*theta5) - 0.25*a2*a5*m5*theta_dot_1*sin(theta3 + theta4 + theta5) - 0.5*a1*a5*m5*theta_dot_3*sin(theta3 + theta4 + theta5) + 0.125*a3*a5*m5*theta_dot_2*sin(theta2 + theta4 + theta5) - 0.5*a1*a5*m5*theta_dot_4*sin(theta3 + theta4 + theta5) + 0.25*a3*a5*m5*theta_dot_3*sin(theta2 + theta4 + theta5) - 0.5*a1*a5*m5*theta_dot_5*sin(theta3 + theta4 + theta5) + 0.25*a3*a5*m5*theta_dot_4*sin(theta2 + theta4 + theta5) + 0.25*a3*a5*m5*theta_dot_5*sin(theta2 + theta4 + theta5) - 0.5*a2*lc5_1*m5*theta_dot_1*sin(theta3 + theta4 + theta5) - 1.0*a1*lc5_1*m5*theta_dot_3*sin(theta3 + theta4 + theta5) + 0.25*a3*lc5_1*m5*theta_dot_2*sin(theta2 + theta4 + theta5) - 1.0*a1*lc5_1*m5*theta_dot_4*sin(theta3 + theta4 + theta5) + 0.5*a3*lc5_1*m5*theta_dot_3*sin(theta2 + theta4 + theta5) - 1.0*a1*lc5_1*m5*theta_dot_5*sin(theta3 + theta4 + theta5) + 0.5*a3*lc5_1*m5*theta_dot_4*sin(theta2 + theta4 + theta5) + 0.5*a3*lc5_1*m5*theta_dot_5*sin(theta2 + theta4 + theta5) + 0.25*a4*lc5_2*m5*theta_dot_2*cos(2.0*theta3 - theta2 + 2.0*theta4 + theta5) + 0.25*a2*lc5_2*m5*theta_dot_1*cos(theta3 - 2.0*theta2 + theta4 + theta5) + 0.25*a2*lc5_2*m5*theta_dot_1*cos(2.0*theta2 + theta3 + theta4 + theta5) + 0.25*a3*lc5_2*m5*theta_dot_2*cos(theta2 + 2.0*theta3 + theta4 + theta5) - 0.125*a5*lc5_3*m5*theta_dot_1*cos(theta3 - 2.0*theta2 + theta4 + theta5) + 0.125*a5*lc5_3*m5*theta_dot_1*cos(2.0*theta2 + theta3 + theta4 + theta5) + 0.125*a4*a5*m5*theta_dot_2*sin(2.0*theta3 - theta2 + 2.0*theta4 + theta5) + 0.125*a2*a5*m5*theta_dot_1*sin(theta3 - 2.0*theta2 + theta4 + theta5) + 0.125*a2*a5*m5*theta_dot_1*sin(2.0*theta2 + theta3 + theta4 + theta5) + 0.125*a3*a5*m5*theta_dot_2*sin(theta2 + 2.0*theta3 + theta4 + theta5) + 0.25*a5*lc5_2*m5*theta_dot_1*cos(2*theta3 + 2*theta4 + 2*theta5) - 0.25*lc5_1*lc5_3*m5*theta_dot_1*cos(theta3 - 2.0*theta2 + theta4 + theta5) + 0.25*lc5_1*lc5_3*m5*theta_dot_1*cos(2.0*theta2 + theta3 + theta4 + theta5) - 0.0625*a4*a5*m5*theta_dot_1*cos(2.0*theta2 + theta5) + 0.25*a4*lc5_1*m5*theta_dot_2*sin(2.0*theta3 - theta2 + 2.0*theta4 + theta5) + 0.25*a2*lc5_1*m5*theta_dot_1*sin(theta3 - 2.0*theta2 + theta4 + theta5) + 0.25*a2*lc5_1*m5*theta_dot_1*sin(2.0*theta2 + theta3 + theta4 + theta5) + 0.25*a3*lc5_1*m5*theta_dot_2*sin(theta2 + 2.0*theta3 + theta4 + theta5) + 0.5*lc5_1*lc5_2*m5*theta_dot_1*cos(2*theta3 + 2*theta4 + 2*theta5) - 0.125*a4*lc5_1*m5*theta_dot_1*cos(2.0*theta2 + theta5) + 0.25*a4*lc5_2*m5*theta_dot_2*cos(theta2 - 1.0*theta5) - 0.5*a4*lc5_2*m5*theta_dot_3*cos(theta2 - 1.0*theta5) - 0.5*a4*lc5_2*m5*theta_dot_4*cos(theta2 - 1.0*theta5) - 0.5*a4*lc5_2*m5*theta_dot_5*cos(theta2 - 1.0*theta5) + 0.25*a5*lc5_1*m5*theta_dot_1*sin(2*theta3 + 2*theta4 + 2*theta5) + 0.25*lc5_2*lc5_3*m5*theta_dot_1*sin(theta3 - 2.0*theta2 + theta4 + theta5) - 0.25*lc5_2*lc5_3*m5*theta_dot_1*sin(2.0*theta2 + theta3 + theta4 + theta5) - 0.125*a4*a5*m5*theta_dot_2*sin(theta2 - 1.0*theta5) + 0.25*a4*a5*m5*theta_dot_3*sin(theta2 - 1.0*theta5) + 0.25*a4*a5*m5*theta_dot_4*sin(theta2 - 1.0*theta5) + 0.25*a4*a5*m5*theta_dot_5*sin(theta2 - 1.0*theta5) + 0.125*a4*a5*m5*theta_dot_1*cos(2.0*theta3 + 2.0*theta4 + theta5) - 0.25*a4*lc5_1*m5*theta_dot_2*sin(theta2 - 1.0*theta5) + 0.5*a4*lc5_1*m5*theta_dot_3*sin(theta2 - 1.0*theta5) + 0.125*a4*lc5_2*m5*theta_dot_1*sin(2.0*theta2 + theta5) + 0.5*a4*lc5_1*m5*theta_dot_4*sin(theta2 - 1.0*theta5) + 0.5*a4*lc5_1*m5*theta_dot_5*sin(theta2 - 1.0*theta5) + 0.25*a4*lc5_1*m5*theta_dot_1*cos(2.0*theta3 + 2.0*theta4 + theta5) + 0.0625*a4*a5*m5*theta_dot_1*cos(2.0*theta3 - 2.0*theta2 + 2.0*theta4 + theta5) + 0.0625*a4*a5*m5*theta_dot_1*cos(2.0*theta2 + 2.0*theta3 + 2.0*theta4 + theta5) - 0.25*a4*lc5_2*m5*theta_dot_1*sin(2.0*theta3 + 2.0*theta4 + theta5) + 0.125*a4*lc5_1*m5*theta_dot_1*cos(2.0*theta3 - 2.0*theta2 + 2.0*theta4 + theta5) + 0.125*a4*lc5_1*m5*theta_dot_1*cos(2.0*theta2 + 2.0*theta3 + 2.0*theta4 + theta5) - 0.25*a5*lc5_1*m5*theta_dot_2*cos(theta2 + 2.0*theta3 + 2.0*theta4 + 2.0*theta5) + 0.25*a3*lc5_2*m5*theta_dot_2*cos(theta4 - theta2 + theta5) - 0.5*a3*lc5_2*m5*theta_dot_3*cos(theta4 - theta2 + theta5) - 0.5*a3*lc5_2*m5*theta_dot_4*cos(theta4 - theta2 + theta5) - 0.5*a3*lc5_2*m5*theta_dot_5*cos(theta4 - theta2 + theta5) - 0.125*a4*lc5_2*m5*theta_dot_1*sin(2.0*theta3 - 2.0*theta2 + 2.0*theta4 + theta5) - 0.125*a4*lc5_2*m5*theta_dot_1*sin(2.0*theta2 + 2.0*theta3 + 2.0*theta4 + theta5) + 0.25*a5*lc5_2*m5*theta_dot_2*sin(theta2 + 2.0*theta3 + 2.0*theta4 + 2.0*theta5) + 0.125*a3*a5*m5*theta_dot_2*sin(theta4 - theta2 + theta5) - 0.25*a3*a5*m5*theta_dot_3*sin(theta4 - theta2 + theta5) - 0.25*a3*a5*m5*theta_dot_4*sin(theta4 - theta2 + theta5) - 0.25*a3*a5*m5*theta_dot_5*sin(theta4 - theta2 + theta5) + 0.25*a1*a5*m5*theta_dot_1*cos(theta2 + theta3 + theta4 + theta5) + 0.25*a2*a5*m5*theta_dot_3*cos(theta2 + theta3 + theta4 + theta5) + 0.25*a2*a5*m5*theta_dot_4*cos(theta2 + theta3 + theta4 + theta5) + 0.25*a2*a5*m5*theta_dot_5*cos(theta2 + theta3 + theta4 + theta5) + 0.5*lc5_1*lc5_2*m5*theta_dot_2*sin(theta2 + 2.0*theta3 + 2.0*theta4 + 2.0*theta5) + 0.25*a3*lc5_1*m5*theta_dot_2*sin(theta4 - theta2 + theta5) - 0.5*a3*lc5_1*m5*theta_dot_3*sin(theta4 - theta2 + theta5) - 0.5*a3*lc5_1*m5*theta_dot_4*sin(theta4 - theta2 + theta5) - 0.5*a3*lc5_1*m5*theta_dot_5*sin(theta4 - theta2 + theta5) + 0.25*a3*lc5_2*m5*theta_dot_2*cos(2.0*theta3 - theta2 + theta4 + theta5) + 0.5*a1*lc5_1*m5*theta_dot_1*cos(theta2 + theta3 + theta4 + theta5) + 0.5*a2*lc5_1*m5*theta_dot_3*cos(theta2 + theta3 + theta4 + theta5) + 0.5*a2*lc5_1*m5*theta_dot_4*cos(theta2 + theta3 + theta4 + theta5) + 0.5*a2*lc5_1*m5*theta_dot_5*cos(theta2 + theta3 + theta4 + theta5) + 0.125*a3*a5*m5*theta_dot_2*sin(2.0*theta3 - theta2 + theta4 + theta5) - 0.5*lc5_2*lc5_3*m5*theta_dot_3*cos(theta2 + theta3 + theta4 + theta5) - 0.5*lc5_2*lc5_3*m5*theta_dot_4*cos(theta2 + theta3 + theta4 + theta5) - 0.5*lc5_2*lc5_3*m5*theta_dot_5*cos(theta2 + theta3 + theta4 + theta5) + 0.375*a3*a5*m5*theta_dot_1*cos(theta4 + theta5) + 0.25*a3*lc5_1*m5*theta_dot_2*sin(2.0*theta3 - theta2 + theta4 + theta5) - 0.5*a1*lc5_2*m5*theta_dot_1*sin(theta2 + theta3 + theta4 + theta5) - 0.5*a2*lc5_2*m5*theta_dot_3*sin(theta2 + theta3 + theta4 + theta5) - 0.5*a2*lc5_2*m5*theta_dot_4*sin(theta2 + theta3 + theta4 + theta5) - 0.5*a2*lc5_2*m5*theta_dot_5*sin(theta2 + theta3 + theta4 + theta5) - 0.25*a5*lc5_3*m5*theta_dot_3*sin(theta2 + theta3 + theta4 + theta5) - 0.25*a5*lc5_3*m5*theta_dot_4*sin(theta2 + theta3 + theta4 + theta5) - 0.25*a5*lc5_3*m5*theta_dot_5*sin(theta2 + theta3 + theta4 + theta5) + 0.75*a3*lc5_1*m5*theta_dot_1*cos(theta4 + theta5) + 0.25*a4*lc5_2*m5*theta_dot_2*cos(theta2 + theta5) + 0.5*a4*lc5_2*m5*theta_dot_3*cos(theta2 + theta5) + 0.5*a4*lc5_2*m5*theta_dot_4*cos(theta2 + theta5) + 0.5*a4*lc5_2*m5*theta_dot_5*cos(theta2 + theta5) - 0.5*lc5_1*lc5_3*m5*theta_dot_3*sin(theta2 + theta3 + theta4 + theta5) - 0.5*lc5_1*lc5_3*m5*theta_dot_4*sin(theta2 + theta3 + theta4 + theta5) - 0.5*lc5_1*lc5_3*m5*theta_dot_5*sin(theta2 + theta3 + theta4 + theta5) + 0.125*a4*a5*m5*theta_dot_2*sin(theta2 + theta5) + 0.25*a4*a5*m5*theta_dot_3*sin(theta2 + theta5) + 0.25*a4*a5*m5*theta_dot_4*sin(theta2 + theta5) + 0.25*a4*a5*m5*theta_dot_5*sin(theta2 + theta5) - 0.0625*a3*a5*m5*theta_dot_1*cos(theta4 - 2.0*theta2 + theta5) - 0.0625*a3*a5*m5*theta_dot_1*cos(2.0*theta2 + theta4 + theta5) + 0.125*a3*a5*m5*theta_dot_1*cos(2.0*theta3 + theta4 + theta5) + 0.25*a4*lc5_1*m5*theta_dot_2*sin(theta2 + theta5) - 0.75*a3*lc5_2*m5*theta_dot_1*sin(theta4 + theta5) + 0.5*a4*lc5_1*m5*theta_dot_3*sin(theta2 + theta5) + 0.5*a4*lc5_1*m5*theta_dot_4*sin(theta2 + theta5) + 0.5*a4*lc5_1*m5*theta_dot_5*sin(theta2 + theta5) - 0.125*a3*lc5_1*m5*theta_dot_1*cos(theta4 - 2.0*theta2 + theta5) - 0.125*a3*lc5_1*m5*theta_dot_1*cos(2.0*theta2 + theta4 + theta5) + 0.25*a3*lc5_1*m5*theta_dot_1*cos(2.0*theta3 + theta4 + theta5) + 0.0625*a3*a5*m5*theta_dot_1*cos(2.0*theta3 - 2.0*theta2 + theta4 + theta5) + 0.0625*a3*a5*m5*theta_dot_1*cos(2.0*theta2 + 2.0*theta3 + theta4 + theta5) + 0.375*a4*a5*m5*theta_dot_1*cos(theta5) + 0.125*a3*lc5_2*m5*theta_dot_1*sin(theta4 - 2.0*theta2 + theta5) + 0.125*a3*lc5_2*m5*theta_dot_1*sin(2.0*theta2 + theta4 + theta5) - 0.25*a3*lc5_2*m5*theta_dot_1*sin(2.0*theta3 + theta4 + theta5) - 0.25*a5*lc5_1*m5*theta_dot_2*cos(2.0*theta3 - theta2 + 2.0*theta4 + 2.0*theta5) + 0.125*a5*lc5_2*m5*theta_dot_1*cos(2.0*theta3 - 2*theta2 + 2.0*theta4 + 2.0*theta5) + 0.125*a3*lc5_1*m5*theta_dot_1*cos(2.0*theta3 - 2.0*theta2 + theta4 + theta5) + 0.125*a3*lc5_1*m5*theta_dot_1*cos(2.0*theta2 + 2.0*theta3 + theta4 + theta5) + 0.25*a4*lc5_2*m5*theta_dot_2*cos(theta2 + 2.0*theta3 + 2.0*theta4 + theta5) + 0.5*a5*lc5_1*m5*theta_dot_2*cos(theta2) + 0.75*a4*lc5_1*m5*theta_dot_1*cos(theta5) + 0.125*a4*a5*m5*theta_dot_2*sin(theta2 + 2.0*theta3 + 2.0*theta4 + theta5) + 0.25*lc5_1*lc5_2*m5*theta_dot_1*cos(2.0*theta3 - 2*theta2 + 2.0*theta4 + 2.0*theta5) - 0.0625*a4*a5*m5*theta_dot_1*cos(2.0*theta2 - 1.0*theta5) + 0.125*a5*lc5_1*m5*theta_dot_1*sin(2.0*theta3 - 2*theta2 + 2.0*theta4 + 2.0*theta5) + 0.25*a5*lc5_2*m5*theta_dot_2*sin(2.0*theta3 - theta2 + 2.0*theta4 + 2.0*theta5) - 0.125*a3*lc5_2*m5*theta_dot_1*sin(2.0*theta3 - 2.0*theta2 + theta4 + theta5) - 0.125*a3*lc5_2*m5*theta_dot_1*sin(2.0*theta2 + 2.0*theta3 + theta4 + theta5) + 0.25*a4*lc5_1*m5*theta_dot_2*sin(theta2 + 2.0*theta3 + 2.0*theta4 + theta5) - 0.75*a4*lc5_2*m5*theta_dot_1*sin(theta5) - 0.25*a1*a5*m5*theta_dot_1*cos(theta3 - theta2 + theta4 + theta5) - 0.25*a2*a5*m5*theta_dot_3*cos(theta3 - theta2 + theta4 + theta5) - 0.25*a2*a5*m5*theta_dot_4*cos(theta3 - theta2 + theta4 + theta5) - 0.25*a2*a5*m5*theta_dot_5*cos(theta3 - theta2 + theta4 + theta5) - 0.125*a4*lc5_1*m5*theta_dot_1*cos(2.0*theta2 - 1.0*theta5) + 0.5*lc5_1*lc5_2*m5*theta_dot_2*sin(2.0*theta3 - theta2 + 2.0*theta4 + 2.0*theta5)


C21a = 0.25*I_xy_3*theta_dot_1*cos(2.0*theta2 - 2.0*theta3) - 0.25*I_xy_3*theta_dot_1*cos(2.0*theta2 + 2.0*theta3) + 0.5*I_yz_5*theta_dot_3*cos(theta3 - theta2 + theta4 + theta5) + 0.5*I_yz_5*theta_dot_4*cos(theta3 - theta2 + theta4 + theta5) + 0.5*I_yz_5*theta_dot_5*cos(theta3 - theta2 + theta4 + theta5) - 0.125*I_xx_3*theta_dot_1*sin(2.0*theta2 - 2.0*theta3) - 0.125*I_xx_3*theta_dot_1*sin(2.0*theta2 + 2.0*theta3) + 0.125*I_yy_3*theta_dot_1*sin(2.0*theta2 - 2.0*theta3) + 0.125*I_yy_3*theta_dot_1*sin(2.0*theta2 + 2.0*theta3) + 0.25*I_xy_4*theta_dot_1*cos(2.0*theta3 - 2.0*theta2 + 2.0*theta4) - 0.25*I_xy_4*theta_dot_1*cos(2.0*theta2 + 2.0*theta3 + 2.0*theta4) + 0.5*I_xz_5*theta_dot_3*sin(theta3 - theta2 + theta4 + theta5) + 0.5*I_xz_5*theta_dot_4*sin(theta3 - theta2 + theta4 + theta5) + 0.5*I_xz_5*theta_dot_5*sin(theta3 - theta2 + theta4 + theta5) + 0.5*I_xz_3*theta_dot_3*cos(theta2 - theta3) + 0.125*I_xx_4*theta_dot_1*sin(2.0*theta3 - 2.0*theta2 + 2.0*theta4) - 0.125*I_xx_4*theta_dot_1*sin(2.0*theta2 + 2.0*theta3 + 2.0*theta4) - 0.125*I_yy_4*theta_dot_1*sin(2.0*theta3 - 2.0*theta2 + 2.0*theta4) + 0.125*I_yy_4*theta_dot_1*sin(2.0*theta2 + 2.0*theta3 + 2.0*theta4) - 0.25*I_xy_5*theta_dot_1*cos(2.0*theta3 - 2.0*theta2 + 2.0*theta4 + 2.0*theta5) + 0.25*I_xy_5*theta_dot_1*cos(2.0*theta2 + 2.0*theta3 + 2.0*theta4 + 2.0*theta5) + 0.5*I_yz_3*theta_dot_3*sin(theta2 - theta3) - 0.5*I_xz_4*theta_dot_3*cos(theta2 + theta3 + theta4) - 0.5*I_xz_4*theta_dot_4*cos(theta2 + theta3 + theta4) - 0.125*I_xx_5*theta_dot_1*sin(2.0*theta3 - 2.0*theta2 + 2.0*theta4 + 2.0*theta5) + 0.125*I_xx_5*theta_dot_1*sin(2.0*theta2 + 2.0*theta3 + 2.0*theta4 + 2.0*theta5) + 0.125*I_yy_5*theta_dot_1*sin(2.0*theta3 - 2.0*theta2 + 2.0*theta4 + 2.0*theta5) - 0.125*I_yy_5*theta_dot_1*sin(2.0*theta2 + 2.0*theta3 + 2.0*theta4 + 2.0*theta5) + 0.5*I_yz_4*theta_dot_3*sin(theta2 + theta3 + theta4) + 0.5*I_yz_4*theta_dot_4*sin(theta2 + theta3 + theta4) + 0.5*I_xz_5*theta_dot_1*cos(theta3 - 2.0*theta2 + theta4 + theta5) + 0.5*I_xz_5*theta_dot_1*cos(2.0*theta2 + theta3 + theta4 + theta5) - 0.5*I_yz_5*theta_dot_1*sin(theta3 - 2.0*theta2 + theta4 + theta5) - 0.5*I_yz_5*theta_dot_1*sin(2.0*theta2 + theta3 + theta4 + theta5) - 0.25*I_xx_3*theta_dot_3*cos(theta2 - 2.0*theta3) - 0.25*I_xx_3*theta_dot_3*cos(theta2 + 2.0*theta3) - 0.5*I_yz_3*theta_dot_1*cos(2.0*theta2 + theta3) + 0.25*I_yy_3*theta_dot_3*cos(theta2 - 2.0*theta3) + 0.25*I_yy_3*theta_dot_3*cos(theta2 + 2.0*theta3) - 0.5*I_xz_3*theta_dot_1*sin(2.0*theta2 + theta3) - 0.5*I_xy_3*theta_dot_3*sin(theta2 - 2.0*theta3) + 0.5*I_xy_3*theta_dot_3*sin(theta2 + 2.0*theta3) - 0.25*I_xx_4*theta_dot_3*cos(theta2 + 2.0*theta3 + 2.0*theta4) - 0.25*I_xx_4*theta_dot_4*cos(theta2 + 2.0*theta3 + 2.0*theta4) + 0.25*I_yy_4*theta_dot_3*cos(theta2 + 2.0*theta3 + 2.0*theta4) + 0.25*I_yy_4*theta_dot_4*cos(theta2 + 2.0*theta3 + 2.0*theta4) + 0.5*I_xy_4*theta_dot_3*sin(theta2 + 2.0*theta3 + 2.0*theta4) + 0.5*I_xy_4*theta_dot_4*sin(theta2 + 2.0*theta3 + 2.0*theta4) + 0.25*I_xx_5*theta_dot_3*cos(theta2 + 2.0*theta3 + 2.0*theta4 + 2.0*theta5) + 0.25*I_xx_5*theta_dot_4*cos(theta2 + 2.0*theta3 + 2.0*theta4 + 2.0*theta5) + 0.25*I_xx_5*theta_dot_5*cos(theta2 + 2.0*theta3 + 2.0*theta4 + 2.0*theta5) - 0.25*I_yy_5*theta_dot_3*cos(theta2 + 2.0*theta3 + 2.0*theta4 + 2.0*theta5) - 0.25*I_yy_5*theta_dot_4*cos(theta2 + 2.0*theta3 + 2.0*theta4 + 2.0*theta5) - 0.25*I_yy_5*theta_dot_5*cos(theta2 + 2.0*theta3 + 2.0*theta4 + 2.0*theta5) + 1.0*I_xz_2*theta_dot_1*cos(2.0*theta2) + 0.5*I_xz_4*theta_dot_3*cos(theta3 - theta2 + theta4) + 0.5*I_xz_4*theta_dot_4*cos(theta3 - theta2 + theta4) - 0.5*I_xy_5*theta_dot_3*sin(theta2 + 2.0*theta3 + 2.0*theta4 + 2.0*theta5) - 0.5*I_xy_5*theta_dot_4*sin(theta2 + 2.0*theta3 + 2.0*theta4 + 2.0*theta5) - 0.5*I_xy_5*theta_dot_5*sin(theta2 + 2.0*theta3 + 2.0*theta4 + 2.0*theta5) + 0.5*I_xx_2*theta_dot_1*sin(2.0*theta2) + 0.25*I_xx_3*theta_dot_1*sin(2.0*theta2) + 0.25*I_xx_4*theta_dot_1*sin(2.0*theta2) + 0.25*I_xx_5*theta_dot_1*sin(2.0*theta2) + 0.25*I_yy_3*theta_dot_1*sin(2.0*theta2) + 0.25*I_yy_4*theta_dot_1*sin(2.0*theta2) + 0.25*I_yy_5*theta_dot_1*sin(2.0*theta2) - 0.5*I_zz_2*theta_dot_1*sin(2.0*theta2) - 0.5*I_zz_3*theta_dot_1*sin(2.0*theta2) - 0.5*I_zz_4*theta_dot_1*sin(2.0*theta2) - 0.5*I_zz_5*theta_dot_1*sin(2.0*theta2) - 0.5*I_yz_4*theta_dot_3*sin(theta3 - theta2 + theta4) - 0.5*I_yz_4*theta_dot_4*sin(theta3 - theta2 + theta4) - 0.5*I_yz_5*theta_dot_3*cos(theta2 + theta3 + theta4 + theta5) - 0.5*I_yz_5*theta_dot_4*cos(theta2 + theta3 + theta4 + theta5) - 0.5*I_yz_5*theta_dot_5*cos(theta2 + theta3 + theta4 + theta5) - 0.5*I_xz_5*theta_dot_3*sin(theta2 + theta3 + theta4 + theta5) - 0.5*I_xz_5*theta_dot_4*sin(theta2 + theta3 + theta4 + theta5) - 0.5*I_xz_5*theta_dot_5*sin(theta2 + theta3 + theta4 + theta5) - 0.5*I_yz_3*theta_dot_1*cos(2.0*theta2 - theta3) - 0.5*I_xz_3*theta_dot_3*cos(theta2 + theta3) + 0.5*I_xz_3*theta_dot_1*sin(2.0*theta2 - theta3) + 0.5*I_yz_3*theta_dot_3*sin(theta2 + theta3) - 0.25*I_xx_4*theta_dot_3*cos(2.0*theta3 - theta2 + 2.0*theta4) - 0.25*I_xx_4*theta_dot_4*cos(2.0*theta3 - theta2 + 2.0*theta4) + 0.25*I_yy_4*theta_dot_3*cos(2.0*theta3 - theta2 + 2.0*theta4) + 0.25*I_yy_4*theta_dot_4*cos(2.0*theta3 - theta2 + 2.0*theta4) - 0.5*I_yz_4*theta_dot_1*cos(theta3 - 2.0*theta2 + theta4) - 0.5*I_yz_4*theta_dot_1*cos(2.0*theta2 + theta3 + theta4) + 0.5*I_xy_4*theta_dot_3*sin(2.0*theta3 - theta2 + 2.0*theta4) + 0.5*I_xy_4*theta_dot_4*sin(2.0*theta3 - theta2 + 2.0*theta4) - 0.5*I_xz_4*theta_dot_1*sin(theta3 - 2.0*theta2 + theta4) - 0.5*I_xz_4*theta_dot_1*sin(2.0*theta2 + theta3 + theta4) + 0.25*I_xx_5*theta_dot_3*cos(2.0*theta3 - theta2 + 2.0*theta4 + 2.0*theta5) + 0.25*I_xx_5*theta_dot_4*cos(2.0*theta3 - theta2 + 2.0*theta4 + 2.0*theta5) + 0.25*I_xx_5*theta_dot_5*cos(2.0*theta3 - theta2 + 2.0*theta4 + 2.0*theta5) - 0.25*I_yy_5*theta_dot_3*cos(2.0*theta3 - theta2 + 2.0*theta4 + 2.0*theta5) - 0.25*I_yy_5*theta_dot_4*cos(2.0*theta3 - theta2 + 2.0*theta4 + 2.0*theta5) - 0.25*I_yy_5*theta_dot_5*cos(2.0*theta3 - theta2 + 2.0*theta4 + 2.0*theta5) - 0.5*I_zz_3*theta_dot_3*cos(theta2) - 0.5*I_zz_4*theta_dot_3*cos(theta2) - 0.5*I_zz_4*theta_dot_4*cos(theta2) - 0.5*I_zz_5*theta_dot_3*cos(theta2) - 0.5*I_zz_5*theta_dot_4*cos(theta2) - 0.5*I_zz_5*theta_dot_5*cos(theta2) - 0.5*I_xy_5*theta_dot_3*sin(2.0*theta3 - theta2 + 2.0*theta4 + 2.0*theta5) - 0.5*I_xy_5*theta_dot_4*sin(2.0*theta3 - theta2 + 2.0*theta4 + 2.0*theta5) - 0.5*I_xy_5*theta_dot_5*sin(2.0*theta3 - theta2 + 2.0*theta4 + 2.0*theta5) + 0.125*lc3_1^2*m3*theta_dot_1*sin(2.0*theta2 - 2.0*theta3) + 0.125*lc3_1^2*m3*theta_dot_1*sin(2.0*theta2 + 2.0*theta3) - 0.125*lc3_2^2*m3*theta_dot_1*sin(2.0*theta2 - 2.0*theta3) - 0.125*lc3_2^2*m3*theta_dot_1*sin(2.0*theta2 + 2.0*theta3) - 0.03125*a4^2*m4*theta_dot_1*sin(2.0*theta3 - 2.0*theta2 + 2.0*theta4) + 0.03125*a4^2*m4*theta_dot_1*sin(2.0*theta2 + 2.0*theta3 + 2.0*theta4) - 0.125*a4^2*m5*theta_dot_1*sin(2.0*theta3 - 2.0*theta2 + 2.0*theta4) + 0.125*a4^2*m5*theta_dot_1*sin(2.0*theta2 + 2.0*theta3 + 2.0*theta4) - 0.125*lc4_1^2*m4*theta_dot_1*sin(2.0*theta3 - 2.0*theta2 + 2.0*theta4) + 0.125*lc4_1^2*m4*theta_dot_1*sin(2.0*theta2 + 2.0*theta3 + 2.0*theta4) + 0.125*lc4_2^2*m4*theta_dot_1*sin(2.0*theta3 - 2.0*theta2 + 2.0*theta4) - 0.125*lc4_2^2*m4*theta_dot_1*sin(2.0*theta2 + 2.0*theta3 + 2.0*theta4) + 0.03125*a5^2*m5*theta_dot_1*sin(2.0*theta3 - 2.0*theta2 + 2.0*theta4 + 2.0*theta5) - 0.03125*a5^2*m5*theta_dot_1*sin(2.0*theta2 + 2.0*theta3 + 2.0*theta4 + 2.0*theta5) + 0.125*lc5_1^2*m5*theta_dot_1*sin(2.0*theta3 - 2.0*theta2 + 2.0*theta4 + 2.0*theta5) - 0.125*lc5_1^2*m5*theta_dot_1*sin(2.0*theta2 + 2.0*theta3 + 2.0*theta4 + 2.0*theta5) - 0.125*lc5_2^2*m5*theta_dot_1*sin(2.0*theta3 - 2.0*theta2 + 2.0*theta4 + 2.0*theta5) + 0.125*lc5_2^2*m5*theta_dot_1*sin(2.0*theta2 + 2.0*theta3 + 2.0*theta4 + 2.0*theta5) + 0.0625*a3^2*m3*theta_dot_3*cos(theta2 - 2.0*theta3) + 0.0625*a3^2*m3*theta_dot_3*cos(theta2 + 2.0*theta3) + 0.25*a3^2*m4*theta_dot_3*cos(theta2 - 2.0*theta3) + 0.25*a3^2*m4*theta_dot_3*cos(theta2 + 2.0*theta3) + 0.25*a3^2*m5*theta_dot_3*cos(theta2 - 2.0*theta3) + 0.25*a3^2*m5*theta_dot_3*cos(theta2 + 2.0*theta3) + 0.25*lc3_1^2*m3*theta_dot_3*cos(theta2 - 2.0*theta3) + 0.25*lc3_1^2*m3*theta_dot_3*cos(theta2 + 2.0*theta3) - 0.25*lc3_2^2*m3*theta_dot_3*cos(theta2 - 2.0*theta3) - 0.25*lc3_2^2*m3*theta_dot_3*cos(theta2 + 2.0*theta3) + 0.0625*a4^2*m4*theta_dot_3*cos(theta2 + 2.0*theta3 + 2.0*theta4) + 0.0625*a4^2*m4*theta_dot_4*cos(theta2 + 2.0*theta3 + 2.0*theta4) + 0.25*a4^2*m5*theta_dot_3*cos(theta2 + 2.0*theta3 + 2.0*theta4) + 0.25*a4^2*m5*theta_dot_4*cos(theta2 + 2.0*theta3 + 2.0*theta4) + 0.25*lc4_1^2*m4*theta_dot_3*cos(theta2 + 2.0*theta3 + 2.0*theta4) + 0.25*lc4_1^2*m4*theta_dot_4*cos(theta2 + 2.0*theta3 + 2.0*theta4) - 0.25*lc4_2^2*m4*theta_dot_3*cos(theta2 + 2.0*theta3 + 2.0*theta4) - 0.25*lc4_2^2*m4*theta_dot_4*cos(theta2 + 2.0*theta3 + 2.0*theta4) - 0.0625*a5^2*m5*theta_dot_3*cos(theta2 + 2.0*theta3 + 2.0*theta4 + 2.0*theta5) - 0.0625*a5^2*m5*theta_dot_4*cos(theta2 + 2.0*theta3 + 2.0*theta4 + 2.0*theta5) - 0.0625*a5^2*m5*theta_dot_5*cos(theta2 + 2.0*theta3 + 2.0*theta4 + 2.0*theta5) - 0.25*lc5_1^2*m5*theta_dot_3*cos(theta2 + 2.0*theta3 + 2.0*theta4 + 2.0*theta5) - 0.25*lc5_1^2*m5*theta_dot_4*cos(theta2 + 2.0*theta3 + 2.0*theta4 + 2.0*theta5) + 0.25*lc5_2^2*m5*theta_dot_3*cos(theta2 + 2.0*theta3 + 2.0*theta4 + 2.0*theta5) - 0.25*lc5_1^2*m5*theta_dot_5*cos(theta2 + 2.0*theta3 + 2.0*theta4 + 2.0*theta5) + 0.25*lc5_2^2*m5*theta_dot_4*cos(theta2 + 2.0*theta3 + 2.0*theta4 + 2.0*theta5) + 0.25*lc5_2^2*m5*theta_dot_5*cos(theta2 + 2.0*theta3 + 2.0*theta4 + 2.0*theta5) - 0.125*a2^2*m2*theta_dot_1*sin(2.0*theta2) - 0.5*a2^2*m3*theta_dot_1*sin(2.0*theta2) - 0.5*a2^2*m4*theta_dot_1*sin(2.0*theta2) - 0.0625*a3^2*m3*theta_dot_1*sin(2.0*theta2) - 0.5*a2^2*m5*theta_dot_1*sin(2.0*theta2) - 0.25*a3^2*m4*theta_dot_1*sin(2.0*theta2) - 0.25*a3^2*m5*theta_dot_1*sin(2.0*theta2) - 0.0625*a4^2*m4*theta_dot_1*sin(2.0*theta2) - 0.25*a4^2*m5*theta_dot_1*sin(2.0*theta2) - 0.0625*a5^2*m5*theta_dot_1*sin(2.0*theta2) - 0.5*lc2_1^2*m2*theta_dot_1*sin(2.0*theta2) + 0.5*lc2_3^2*m2*theta_dot_1*sin(2.0*theta2) - 0.25*lc3_1^2*m3*theta_dot_1*sin(2.0*theta2) - 0.25*lc3_2^2*m3*theta_dot_1*sin(2.0*theta2) + 0.5*lc3_3^2*m3*theta_dot_1*sin(2.0*theta2) - 0.25*lc4_1^2*m4*theta_dot_1*sin(2.0*theta2) - 0.25*lc4_2^2*m4*theta_dot_1*sin(2.0*theta2) + 0.5*lc4_3^2*m4*theta_dot_1*sin(2.0*theta2) - 0.25*lc5_1^2*m5*theta_dot_1*sin(2.0*theta2) - 0.25*lc5_2^2*m5*theta_dot_1*sin(2.0*theta2) + 0.5*lc5_3^2*m5*theta_dot_1*sin(2.0*theta2) + 0.0625*a4^2*m4*theta_dot_3*cos(2.0*theta3 - theta2 + 2.0*theta4) + 0.0625*a4^2*m4*theta_dot_4*cos(2.0*theta3 - theta2 + 2.0*theta4) + 0.25*a4^2*m5*theta_dot_3*cos(2.0*theta3 - theta2 + 2.0*theta4) + 0.25*a4^2*m5*theta_dot_4*cos(2.0*theta3 - theta2 + 2.0*theta4) + 0.25*lc4_1^2*m4*theta_dot_3*cos(2.0*theta3 - theta2 + 2.0*theta4) + 0.25*lc4_1^2*m4*theta_dot_4*cos(2.0*theta3 - theta2 + 2.0*theta4) - 0.25*lc4_2^2*m4*theta_dot_3*cos(2.0*theta3 - theta2 + 2.0*theta4) - 0.25*lc4_2^2*m4*theta_dot_4*cos(2.0*theta3 - theta2 + 2.0*theta4) - 0.0625*a5^2*m5*theta_dot_3*cos(2.0*theta3 - theta2 + 2.0*theta4 + 2.0*theta5) - 0.0625*a5^2*m5*theta_dot_4*cos(2.0*theta3 - theta2 + 2.0*theta4 + 2.0*theta5) - 0.0625*a5^2*m5*theta_dot_5*cos(2.0*theta3 - theta2 + 2.0*theta4 + 2.0*theta5) - 0.125*a3^2*m3*theta_dot_3*cos(theta2) - 0.5*a3^2*m4*theta_dot_3*cos(theta2) - 0.5*a3^2*m5*theta_dot_3*cos(theta2) - 0.125*a4^2*m4*theta_dot_3*cos(theta2) - 0.125*a4^2*m4*theta_dot_4*cos(theta2) - 0.5*a4^2*m5*theta_dot_3*cos(theta2) - 0.5*a4^2*m5*theta_dot_4*cos(theta2) - 0.125*a5^2*m5*theta_dot_3*cos(theta2) - 0.125*a5^2*m5*theta_dot_4*cos(theta2) - 0.125*a5^2*m5*theta_dot_5*cos(theta2) - 0.25*lc5_1^2*m5*theta_dot_3*cos(2.0*theta3 - theta2 + 2.0*theta4 + 2.0*theta5) - 0.25*lc5_1^2*m5*theta_dot_4*cos(2.0*theta3 - theta2 + 2.0*theta4 + 2.0*theta5) + 0.25*lc5_2^2*m5*theta_dot_3*cos(2.0*theta3 - theta2 + 2.0*theta4 + 2.0*theta5) - 0.25*lc5_1^2*m5*theta_dot_5*cos(2.0*theta3 - theta2 + 2.0*theta4 + 2.0*theta5) + 0.25*lc5_2^2*m5*theta_dot_4*cos(2.0*theta3 - theta2 + 2.0*theta4 + 2.0*theta5) + 0.25*lc5_2^2*m5*theta_dot_5*cos(2.0*theta3 - theta2 + 2.0*theta4 + 2.0*theta5) - 0.5*lc3_1^2*m3*theta_dot_3*cos(theta2) - 0.5*lc3_2^2*m3*theta_dot_3*cos(theta2) - 0.5*lc4_1^2*m4*theta_dot_3*cos(theta2) - 0.5*lc4_1^2*m4*theta_dot_4*cos(theta2) - 0.5*lc4_2^2*m4*theta_dot_3*cos(theta2) - 0.5*lc4_2^2*m4*theta_dot_4*cos(theta2) - 0.5*lc5_1^2*m5*theta_dot_3*cos(theta2) - 0.5*lc5_1^2*m5*theta_dot_4*cos(theta2) - 0.5*lc5_2^2*m5*theta_dot_3*cos(theta2) - 0.5*lc5_1^2*m5*theta_dot_5*cos(theta2) - 0.5*lc5_2^2*m5*theta_dot_4*cos(theta2) - 0.5*lc5_2^2*m5*theta_dot_5*cos(theta2) + 0.03125*a3^2*m3*theta_dot_1*sin(2.0*theta2 - 2.0*theta3) + 0.03125*a3^2*m3*theta_dot_1*sin(2.0*theta2 + 2.0*theta3) + 0.125*a3^2*m4*theta_dot_1*sin(2.0*theta2 - 2.0*theta3) + 0.125*a3^2*m4*theta_dot_1*sin(2.0*theta2 + 2.0*theta3) + 0.125*a3^2*m5*theta_dot_1*sin(2.0*theta2 - 2.0*theta3) + 0.125*a3^2*m5*theta_dot_1*sin(2.0*theta2 + 2.0*theta3) - 0.5*a1*lc5_1*m5*theta_dot_1*cos(theta3 - theta2 + theta4 + theta5) - 0.5*a2*lc5_1*m5*theta_dot_3*cos(theta3 - theta2 + theta4 + theta5) - 0.5*a2*lc5_1*m5*theta_dot_4*cos(theta3 - theta2 + theta4 + theta5) - 0.5*a2*lc5_1*m5*theta_dot_5*cos(theta3 - theta2 + theta4 + theta5) - 0.25*lc3_1*lc3_2*m3*theta_dot_1*cos(2.0*theta2 - 2.0*theta3) + 0.25*lc3_1*lc3_2*m3*theta_dot_1*cos(2.0*theta2 + 2.0*theta3) + 0.125*a3*lc3_1*m3*theta_dot_1*sin(2.0*theta2 - 2.0*theta3) + 0.125*a3*lc3_1*m3*theta_dot_1*sin(2.0*theta2 + 2.0*theta3) - 0.125*a4*lc4_2*m4*theta_dot_1*cos(2.0*theta3 - 2.0*theta2 + 2.0*theta4) + 0.125*a4*lc4_2*m4*theta_dot_1*cos(2.0*theta2 + 2.0*theta3 + 2.0*theta4) - 0.5*lc5_2*lc5_3*m5*theta_dot_3*cos(theta3 - theta2 + theta4 + theta5) - 0.5*lc5_2*lc5_3*m5*theta_dot_4*cos(theta3 - theta2 + theta4 + theta5) - 0.5*lc5_2*lc5_3*m5*theta_dot_5*cos(theta3 - theta2 + theta4 + theta5) - 0.25*a3*a4*m4*theta_dot_3*cos(theta2 - theta4) - 0.125*a3*a4*m4*theta_dot_4*cos(theta2 - theta4) - 0.5*a3*a4*m5*theta_dot_3*cos(theta2 - theta4) - 0.25*a3*a4*m5*theta_dot_4*cos(theta2 - theta4) + 0.5*a1*lc5_2*m5*theta_dot_1*sin(theta3 - theta2 + theta4 + theta5) + 0.5*a2*lc5_2*m5*theta_dot_3*sin(theta3 - theta2 + theta4 + theta5) + 0.5*a2*lc5_2*m5*theta_dot_4*sin(theta3 - theta2 + theta4 + theta5) + 0.5*a2*lc5_2*m5*theta_dot_5*sin(theta3 - theta2 + theta4 + theta5) - 0.25*a5*lc5_3*m5*theta_dot_3*sin(theta3 - theta2 + theta4 + theta5) - 0.25*a5*lc5_3*m5*theta_dot_4*sin(theta3 - theta2 + theta4 + theta5) - 0.25*a5*lc5_3*m5*theta_dot_5*sin(theta3 - theta2 + theta4 + theta5) - 0.25*lc4_1*lc4_2*m4*theta_dot_1*cos(2.0*theta3 - 2.0*theta2 + 2.0*theta4) + 0.25*lc4_1*lc4_2*m4*theta_dot_1*cos(2.0*theta2 + 2.0*theta3 + 2.0*theta4) + 0.5*a1*lc3_2*m3*theta_dot_1*cos(theta2 - theta3) + 0.5*a2*lc3_2*m3*theta_dot_3*cos(theta2 - theta3) - 0.25*a3*lc3_3*m3*theta_dot_3*cos(theta2 - theta3) - 0.5*a3*lc4_1*m4*theta_dot_3*cos(theta2 - theta4) - 0.25*a3*lc4_1*m4*theta_dot_4*cos(theta2 - theta4) - 0.5*a3*lc4_3*m4*theta_dot_3*cos(theta2 - theta3) - 0.5*a3*lc5_3*m5*theta_dot_3*cos(theta2 - theta3) - 0.5*a4*lc5_2*m5*theta_dot_3*cos(theta2 - theta5) - 0.5*a4*lc5_2*m5*theta_dot_4*cos(theta2 - theta5) - 0.25*a4*lc5_2*m5*theta_dot_5*cos(theta2 - theta5) - 0.125*a4*lc4_1*m4*theta_dot_1*sin(2.0*theta3 - 2.0*theta2 + 2.0*theta4) + 0.125*a4*lc4_1*m4*theta_dot_1*sin(2.0*theta2 + 2.0*theta3 + 2.0*theta4) - 0.5*lc5_1*lc5_3*m5*theta_dot_3*sin(theta3 - theta2 + theta4 + theta5) - 0.5*lc5_1*lc5_3*m5*theta_dot_4*sin(theta3 - theta2 + theta4 + theta5) - 0.5*lc5_1*lc5_3*m5*theta_dot_5*sin(theta3 - theta2 + theta4 + theta5) - 0.25*a1*a3*m3*theta_dot_1*sin(theta2 - theta3) - 0.5*a1*a3*m4*theta_dot_1*sin(theta2 - theta3) - 0.5*a1*a3*m5*theta_dot_1*sin(theta2 - theta3) - 0.25*a2*a3*m3*theta_dot_3*sin(theta2 - theta3) - 0.5*a2*a3*m4*theta_dot_3*sin(theta2 - theta3) - 0.5*a2*a3*m5*theta_dot_3*sin(theta2 - theta3) + 0.25*a4*a5*m5*theta_dot_3*sin(theta2 - theta5) + 0.25*a4*a5*m5*theta_dot_4*sin(theta2 - theta5) + 0.125*a4*a5*m5*theta_dot_5*sin(theta2 - theta5) + 0.125*a5*lc5_2*m5*theta_dot_1*cos(2.0*theta3 - 2.0*theta2 + 2.0*theta4 + 2.0*theta5) - 0.125*a5*lc5_2*m5*theta_dot_1*cos(2.0*theta2 + 2.0*theta3 + 2.0*theta4 + 2.0*theta5) + 0.25*a3*a4*m4*theta_dot_3*cos(2.0*theta3 - theta2 + theta4) + 0.125*a3*a4*m4*theta_dot_4*cos(2.0*theta3 - theta2 + theta4) + 0.5*a3*a4*m5*theta_dot_3*cos(2.0*theta3 - theta2 + theta4) + 0.25*a3*a4*m5*theta_dot_4*cos(2.0*theta3 - theta2 + theta4) - 0.5*lc3_1*lc3_3*m3*theta_dot_3*cos(theta2 - theta3) - 0.5*a1*lc3_1*m3*theta_dot_1*sin(theta2 - theta3) - 0.5*a2*lc3_1*m3*theta_dot_3*sin(theta2 - theta3) - 0.5*a3*lc4_2*m4*theta_dot_3*sin(theta2 - theta4) - 0.25*a3*lc4_2*m4*theta_dot_4*sin(theta2 - theta4) + 0.5*a4*lc5_1*m5*theta_dot_3*sin(theta2 - theta5) + 0.5*a4*lc5_1*m5*theta_dot_4*sin(theta2 - theta5) + 0.25*a4*lc5_1*m5*theta_dot_5*sin(theta2 - theta5) + 0.25*lc5_1*lc5_2*m5*theta_dot_1*cos(2.0*theta3 - 2.0*theta2 + 2.0*theta4 + 2.0*theta5) - 0.25*lc5_1*lc5_2*m5*theta_dot_1*cos(2.0*theta2 + 2.0*theta3 + 2.0*theta4 + 2.0*theta5) 
C21b = 0.5*a3*lc4_1*m4*theta_dot_3*cos(2.0*theta3 - theta2 + theta4) + 0.25*a3*lc4_1*m4*theta_dot_4*cos(2.0*theta3 - theta2 + theta4) + 0.5*a1*lc4_2*m4*theta_dot_1*cos(theta2 + theta3 + theta4) + 0.5*a2*lc4_2*m4*theta_dot_3*cos(theta2 + theta3 + theta4) + 0.5*a2*lc4_2*m4*theta_dot_4*cos(theta2 + theta3 + theta4) + 0.25*a4*lc4_3*m4*theta_dot_3*cos(theta2 + theta3 + theta4) + 0.25*a4*lc4_3*m4*theta_dot_4*cos(theta2 + theta3 + theta4) - 0.5*a3*lc5_2*m5*theta_dot_3*cos(theta2 + theta4 + theta5) + 0.5*a4*lc5_3*m5*theta_dot_3*cos(theta2 + theta3 + theta4) - 0.25*a3*lc5_2*m5*theta_dot_4*cos(theta2 + theta4 + theta5) + 0.5*a4*lc5_3*m5*theta_dot_4*cos(theta2 + theta3 + theta4) - 0.25*a3*lc5_2*m5*theta_dot_5*cos(theta2 + theta4 + theta5) + 0.125*a5*lc5_1*m5*theta_dot_1*sin(2.0*theta3 - 2.0*theta2 + 2.0*theta4 + 2.0*theta5) - 0.125*a5*lc5_1*m5*theta_dot_1*sin(2.0*theta2 + 2.0*theta3 + 2.0*theta4 + 2.0*theta5) + 0.25*a1*a4*m4*theta_dot_1*sin(theta2 + theta3 + theta4) + 0.5*a1*a4*m5*theta_dot_1*sin(theta2 + theta3 + theta4) + 0.25*a2*a4*m4*theta_dot_3*sin(theta2 + theta3 + theta4) + 0.25*a2*a4*m4*theta_dot_4*sin(theta2 + theta3 + theta4) + 0.5*a2*a4*m5*theta_dot_3*sin(theta2 + theta3 + theta4) + 0.5*a2*a4*m5*theta_dot_4*sin(theta2 + theta3 + theta4) - 0.25*a3*a5*m5*theta_dot_3*sin(theta2 + theta4 + theta5) - 0.125*a3*a5*m5*theta_dot_4*sin(theta2 + theta4 + theta5) - 0.125*a3*a5*m5*theta_dot_5*sin(theta2 + theta4 + theta5) - 0.5*lc3_2*lc3_3*m3*theta_dot_3*sin(theta2 - theta3) + 0.5*lc4_1*lc4_3*m4*theta_dot_3*cos(theta2 + theta3 + theta4) + 0.5*lc4_1*lc4_3*m4*theta_dot_4*cos(theta2 + theta3 + theta4) - 0.5*a3*lc4_2*m4*theta_dot_3*sin(2.0*theta3 - theta2 + theta4) - 0.25*a3*lc4_2*m4*theta_dot_4*sin(2.0*theta3 - theta2 + theta4) + 0.5*a1*lc4_1*m4*theta_dot_1*sin(theta2 + theta3 + theta4) + 0.5*a2*lc4_1*m4*theta_dot_3*sin(theta2 + theta3 + theta4) + 0.5*a2*lc4_1*m4*theta_dot_4*sin(theta2 + theta3 + theta4) - 0.5*a3*lc5_1*m5*theta_dot_3*sin(theta2 + theta4 + theta5) - 0.25*a3*lc5_1*m5*theta_dot_4*sin(theta2 + theta4 + theta5) - 0.25*a3*lc5_1*m5*theta_dot_5*sin(theta2 + theta4 + theta5) + 0.5*a4*lc5_2*m5*theta_dot_3*cos(2.0*theta3 - theta2 + 2.0*theta4 + theta5) + 0.5*a4*lc5_2*m5*theta_dot_4*cos(2.0*theta3 - theta2 + 2.0*theta4 + theta5) + 0.25*a4*lc5_2*m5*theta_dot_5*cos(2.0*theta3 - theta2 + 2.0*theta4 + theta5) + 0.5*a2*lc5_2*m5*theta_dot_1*cos(theta3 - 2.0*theta2 + theta4 + theta5) - 0.5*a2*lc5_2*m5*theta_dot_1*cos(2.0*theta2 + theta3 + theta4 + theta5) + 0.5*a3*lc5_2*m5*theta_dot_3*cos(theta2 + 2.0*theta3 + theta4 + theta5) + 0.25*a3*lc5_2*m5*theta_dot_4*cos(theta2 + 2.0*theta3 + theta4 + theta5) - 0.25*a5*lc5_3*m5*theta_dot_1*cos(theta3 - 2.0*theta2 + theta4 + theta5) - 0.25*a5*lc5_3*m5*theta_dot_1*cos(2.0*theta2 + theta3 + theta4 + theta5) + 0.25*a3*lc5_2*m5*theta_dot_5*cos(theta2 + 2.0*theta3 + theta4 + theta5) + 0.25*a4*a5*m5*theta_dot_3*sin(2.0*theta3 - theta2 + 2.0*theta4 + theta5) + 0.25*a4*a5*m5*theta_dot_4*sin(2.0*theta3 - theta2 + 2.0*theta4 + theta5) + 0.125*a4*a5*m5*theta_dot_5*sin(2.0*theta3 - theta2 + 2.0*theta4 + theta5) + 0.25*a2*a5*m5*theta_dot_1*sin(theta3 - 2.0*theta2 + theta4 + theta5) - 0.25*a2*a5*m5*theta_dot_1*sin(2.0*theta2 + theta3 + theta4 + theta5) + 0.25*a3*a5*m5*theta_dot_3*sin(theta2 + 2.0*theta3 + theta4 + theta5) + 0.125*a3*a5*m5*theta_dot_4*sin(theta2 + 2.0*theta3 + theta4 + theta5) + 0.125*a3*a5*m5*theta_dot_5*sin(theta2 + 2.0*theta3 + theta4 + theta5) - 0.5*lc4_2*lc4_3*m4*theta_dot_3*sin(theta2 + theta3 + theta4) - 0.5*lc4_2*lc4_3*m4*theta_dot_4*sin(theta2 + theta3 + theta4) - 0.5*lc5_1*lc5_3*m5*theta_dot_1*cos(theta3 - 2.0*theta2 + theta4 + theta5) - 0.5*lc5_1*lc5_3*m5*theta_dot_1*cos(2.0*theta2 + theta3 + theta4 + theta5) - 0.25*a2*a3*m3*theta_dot_1*cos(2.0*theta2 + theta3) - 0.5*a2*a3*m4*theta_dot_1*cos(2.0*theta2 + theta3) - 0.5*a2*a3*m5*theta_dot_1*cos(2.0*theta2 + theta3) + 0.125*a4*a5*m5*theta_dot_1*cos(2.0*theta2 + theta5) + 0.5*a4*lc5_1*m5*theta_dot_3*sin(2.0*theta3 - theta2 + 2.0*theta4 + theta5) + 0.5*a4*lc5_1*m5*theta_dot_4*sin(2.0*theta3 - theta2 + 2.0*theta4 + theta5) + 0.25*a4*lc5_1*m5*theta_dot_5*sin(2.0*theta3 - theta2 + 2.0*theta4 + theta5) + 0.5*a2*lc5_1*m5*theta_dot_1*sin(theta3 - 2.0*theta2 + theta4 + theta5) - 0.5*a2*lc5_1*m5*theta_dot_1*sin(2.0*theta2 + theta3 + theta4 + theta5) + 0.5*a3*lc5_1*m5*theta_dot_3*sin(theta2 + 2.0*theta3 + theta4 + theta5) + 0.25*a3*lc5_1*m5*theta_dot_4*sin(theta2 + 2.0*theta3 + theta4 + theta5) + 0.25*a3*lc5_1*m5*theta_dot_5*sin(theta2 + 2.0*theta3 + theta4 + theta5) - 0.5*a2*lc3_1*m3*theta_dot_1*cos(2.0*theta2 + theta3) + 0.25*a3*lc3_1*m3*theta_dot_3*cos(theta2 - 2.0*theta3) + 0.25*a3*lc3_1*m3*theta_dot_3*cos(theta2 + 2.0*theta3) - 0.25*a3*lc4_2*m4*theta_dot_1*cos(2.0*theta2 + theta4) + 0.25*a4*lc5_1*m5*theta_dot_1*cos(2.0*theta2 + theta5) + 0.5*lc5_2*lc5_3*m5*theta_dot_1*sin(theta3 - 2.0*theta2 + theta4 + theta5) + 0.5*lc5_2*lc5_3*m5*theta_dot_1*sin(2.0*theta2 + theta3 + theta4 + theta5) - 0.125*a3*a4*m4*theta_dot_1*sin(2.0*theta2 + theta4) - 0.25*a3*a4*m5*theta_dot_1*sin(2.0*theta2 + theta4) + 0.5*lc3_2*lc3_3*m3*theta_dot_1*cos(2.0*theta2 + theta3) + 0.5*a2*lc3_2*m3*theta_dot_1*sin(2.0*theta2 + theta3) + 0.25*a3*lc3_3*m3*theta_dot_1*sin(2.0*theta2 + theta3) + 0.25*a3*lc3_2*m3*theta_dot_3*sin(theta2 - 2.0*theta3) - 0.25*a3*lc3_2*m3*theta_dot_3*sin(theta2 + 2.0*theta3) - 0.25*a3*lc4_1*m4*theta_dot_1*sin(2.0*theta2 + theta4) + 0.5*a3*lc4_3*m4*theta_dot_1*sin(2.0*theta2 + theta3) + 0.5*a3*lc5_3*m5*theta_dot_1*sin(2.0*theta2 + theta3) - 0.25*a4*lc5_2*m5*theta_dot_1*sin(2.0*theta2 + theta5) - 0.25*a3*lc4_2*m4*theta_dot_1*cos(2.0*theta3 - 2.0*theta2 + theta4) + 0.25*a3*lc4_2*m4*theta_dot_1*cos(2.0*theta2 + 2.0*theta3 + theta4) + 0.25*a4*lc4_1*m4*theta_dot_3*cos(theta2 + 2.0*theta3 + 2.0*theta4) + 0.25*a4*lc4_1*m4*theta_dot_4*cos(theta2 + 2.0*theta3 + 2.0*theta4) - 0.125*a3*a4*m4*theta_dot_1*sin(2.0*theta3 - 2.0*theta2 + theta4) + 0.125*a3*a4*m4*theta_dot_1*sin(2.0*theta2 + 2.0*theta3 + theta4) - 0.25*a3*a4*m5*theta_dot_1*sin(2.0*theta3 - 2.0*theta2 + theta4) + 0.25*a3*a4*m5*theta_dot_1*sin(2.0*theta2 + 2.0*theta3 + theta4) + 0.5*lc3_1*lc3_3*m3*theta_dot_1*sin(2.0*theta2 + theta3) + 0.5*lc3_1*lc3_2*m3*theta_dot_3*sin(theta2 - 2.0*theta3) - 0.5*lc3_1*lc3_2*m3*theta_dot_3*sin(theta2 + 2.0*theta3) + 0.125*a4*a5*m5*theta_dot_1*cos(2.0*theta3 - 2.0*theta2 + 2.0*theta4 + theta5) - 0.125*a4*a5*m5*theta_dot_1*cos(2.0*theta2 + 2.0*theta3 + 2.0*theta4 + theta5) - 0.25*a3*lc4_1*m4*theta_dot_1*sin(2.0*theta3 - 2.0*theta2 + theta4) + 0.25*a3*lc4_1*m4*theta_dot_1*sin(2.0*theta2 + 2.0*theta3 + theta4) - 0.25*a4*lc4_2*m4*theta_dot_3*sin(theta2 + 2.0*theta3 + 2.0*theta4) - 0.25*a4*lc4_2*m4*theta_dot_4*sin(theta2 + 2.0*theta3 + 2.0*theta4) + 0.25*a4*lc5_1*m5*theta_dot_1*cos(2.0*theta3 - 2.0*theta2 + 2.0*theta4 + theta5) - 0.25*a4*lc5_1*m5*theta_dot_1*cos(2.0*theta2 + 2.0*theta3 + 2.0*theta4 + theta5) - 0.25*a5*lc5_1*m5*theta_dot_3*cos(theta2 + 2.0*theta3 + 2.0*theta4 + 2.0*theta5) - 0.25*a5*lc5_1*m5*theta_dot_4*cos(theta2 + 2.0*theta3 + 2.0*theta4 + 2.0*theta5) - 0.25*a5*lc5_1*m5*theta_dot_5*cos(theta2 + 2.0*theta3 + 2.0*theta4 + 2.0*theta5) - 0.5*a2*lc2_3*m2*theta_dot_1*cos(2.0*theta2) - 1.0*a2*lc3_3*m3*theta_dot_1*cos(2.0*theta2) - 1.0*a2*lc4_3*m4*theta_dot_1*cos(2.0*theta2) - 1.0*a2*lc5_3*m5*theta_dot_1*cos(2.0*theta2) - 0.5*lc4_1*lc4_2*m4*theta_dot_3*sin(theta2 + 2.0*theta3 + 2.0*theta4) - 0.5*lc4_1*lc4_2*m4*theta_dot_4*sin(theta2 + 2.0*theta3 + 2.0*theta4) + 0.5*a1*lc4_2*m4*theta_dot_1*cos(theta3 - theta2 + theta4) + 0.5*a2*lc4_2*m4*theta_dot_3*cos(theta3 - theta2 + theta4) + 0.5*a2*lc4_2*m4*theta_dot_4*cos(theta3 - theta2 + theta4) - 0.25*a4*lc4_3*m4*theta_dot_3*cos(theta3 - theta2 + theta4) - 0.25*a4*lc4_3*m4*theta_dot_4*cos(theta3 - theta2 + theta4) - 0.5*a3*lc5_2*m5*theta_dot_3*cos(theta4 - theta2 + theta5) - 0.5*a4*lc5_3*m5*theta_dot_3*cos(theta3 - theta2 + theta4) - 0.25*a3*lc5_2*m5*theta_dot_4*cos(theta4 - theta2 + theta5) - 0.5*a4*lc5_3*m5*theta_dot_4*cos(theta3 - theta2 + theta4) - 0.25*a3*lc5_2*m5*theta_dot_5*cos(theta4 - theta2 + theta5) - 1.0*lc2_1*lc2_3*m2*theta_dot_1*cos(2.0*theta2) - 0.25*a4*lc5_2*m5*theta_dot_1*sin(2.0*theta3 - 2.0*theta2 + 2.0*theta4 + theta5) + 0.25*a4*lc5_2*m5*theta_dot_1*sin(2.0*theta2 + 2.0*theta3 + 2.0*theta4 + theta5) + 0.25*a5*lc5_2*m5*theta_dot_3*sin(theta2 + 2.0*theta3 + 2.0*theta4 + 2.0*theta5) + 0.25*a5*lc5_2*m5*theta_dot_4*sin(theta2 + 2.0*theta3 + 2.0*theta4 + 2.0*theta5) + 0.25*a5*lc5_2*m5*theta_dot_5*sin(theta2 + 2.0*theta3 + 2.0*theta4 + 2.0*theta5) + 0.25*a1*a4*m4*theta_dot_1*sin(theta3 - theta2 + theta4) + 0.5*a1*a4*m5*theta_dot_1*sin(theta3 - theta2 + theta4) + 0.25*a2*a4*m4*theta_dot_3*sin(theta3 - theta2 + theta4) + 0.25*a2*a4*m4*theta_dot_4*sin(theta3 - theta2 + theta4) + 0.5*a2*a4*m5*theta_dot_3*sin(theta3 - theta2 + theta4) + 0.5*a2*a4*m5*theta_dot_4*sin(theta3 - theta2 + theta4) - 0.25*a3*a5*m5*theta_dot_3*sin(theta4 - theta2 + theta5) - 0.125*a3*a5*m5*theta_dot_4*sin(theta4 - theta2 + theta5) - 0.125*a3*a5*m5*theta_dot_5*sin(theta4 - theta2 + theta5) - 0.5*a2*lc2_1*m2*theta_dot_1*sin(2.0*theta2) - 0.25*a3*lc3_1*m3*theta_dot_1*sin(2.0*theta2) - 0.25*a4*lc4_1*m4*theta_dot_1*sin(2.0*theta2) - 0.25*a5*lc5_1*m5*theta_dot_1*sin(2.0*theta2) - 0.25*a1*a5*m5*theta_dot_1*cos(theta2 + theta3 + theta4 + theta5) - 0.25*a2*a5*m5*theta_dot_3*cos(theta2 + theta3 + theta4 + theta5) - 0.25*a2*a5*m5*theta_dot_4*cos(theta2 + theta3 + theta4 + theta5) - 0.25*a2*a5*m5*theta_dot_5*cos(theta2 + theta3 + theta4 + theta5) - 0.5*lc4_1*lc4_3*m4*theta_dot_3*cos(theta3 - theta2 + theta4) - 0.5*lc4_1*lc4_3*m4*theta_dot_4*cos(theta3 - theta2 + theta4) + 0.5*lc5_1*lc5_2*m5*theta_dot_3*sin(theta2 + 2.0*theta3 + 2.0*theta4 + 2.0*theta5) + 0.5*lc5_1*lc5_2*m5*theta_dot_4*sin(theta2 + 2.0*theta3 + 2.0*theta4 + 2.0*theta5) + 0.5*lc5_1*lc5_2*m5*theta_dot_5*sin(theta2 + 2.0*theta3 + 2.0*theta4 + 2.0*theta5) + 0.5*a1*lc4_1*m4*theta_dot_1*sin(theta3 - theta2 + theta4) + 0.5*a2*lc4_1*m4*theta_dot_3*sin(theta3 - theta2 + theta4) + 0.5*a2*lc4_1*m4*theta_dot_4*sin(theta3 - theta2 + theta4) - 0.5*a3*lc5_1*m5*theta_dot_3*sin(theta4 - theta2 + theta5) - 0.25*a3*lc5_1*m5*theta_dot_4*sin(theta4 - theta2 + theta5) - 0.25*a3*lc5_1*m5*theta_dot_5*sin(theta4 - theta2 + theta5) + 0.5*a3*lc5_2*m5*theta_dot_3*cos(2.0*theta3 - theta2 + theta4 + theta5) + 0.25*a3*lc5_2*m5*theta_dot_4*cos(2.0*theta3 - theta2 + theta4 + theta5) + 0.25*a3*lc5_2*m5*theta_dot_5*cos(2.0*theta3 - theta2 + theta4 + theta5) - 0.5*a1*lc5_1*m5*theta_dot_1*cos(theta2 + theta3 + theta4 + theta5) - 0.5*a2*lc5_1*m5*theta_dot_3*cos(theta2 + theta3 + theta4 + theta5) - 0.5*a2*lc5_1*m5*theta_dot_4*cos(theta2 + theta3 + theta4 + theta5) - 0.5*a2*lc5_1*m5*theta_dot_5*cos(theta2 + theta3 + theta4 + theta5) + 0.25*a3*a5*m5*theta_dot_3*sin(2.0*theta3 - theta2 + theta4 + theta5) + 0.125*a3*a5*m5*theta_dot_4*sin(2.0*theta3 - theta2 + theta4 + theta5) + 0.125*a3*a5*m5*theta_dot_5*sin(2.0*theta3 - theta2 + theta4 + theta5) + 0.5*lc4_2*lc4_3*m4*theta_dot_3*sin(theta3 - theta2 + theta4) + 0.5*lc4_2*lc4_3*m4*theta_dot_4*sin(theta3 - theta2 + theta4) + 0.25*a2*a3*m3*theta_dot_1*cos(2.0*theta2 - theta3) + 0.5*a2*a3*m4*theta_dot_1*cos(2.0*theta2 - theta3) + 0.5*a2*a3*m5*theta_dot_1*cos(2.0*theta2 - theta3) - 0.125*a4*a5*m5*theta_dot_1*cos(2.0*theta2 - theta5) + 0.5*lc5_2*lc5_3*m5*theta_dot_3*cos(theta2 + theta3 + theta4 + theta5) + 0.5*lc5_2*lc5_3*m5*theta_dot_4*cos(theta2 + theta3 + theta4 + theta5) + 0.5*lc5_2*lc5_3*m5*theta_dot_5*cos(theta2 + theta3 + theta4 + theta5) - 0.25*a3*a4*m4*theta_dot_3*cos(theta2 + theta4) - 0.125*a3*a4*m4*theta_dot_4*cos(theta2 + theta4) - 0.5*a3*a4*m5*theta_dot_3*cos(theta2 + theta4) - 0.25*a3*a4*m5*theta_dot_4*cos(theta2 + theta4) + 0.5*a3*lc5_1*m5*theta_dot_3*sin(2.0*theta3 - theta2 + theta4 + theta5) + 0.25*a3*lc5_1*m5*theta_dot_4*sin(2.0*theta3 - theta2 + theta4 + theta5) + 0.25*a3*lc5_1*m5*theta_dot_5*sin(2.0*theta3 - theta2 + theta4 + theta5) + 0.5*a1*lc5_2*m5*theta_dot_1*sin(theta2 + theta3 + theta4 + theta5) + 0.5*a2*lc5_2*m5*theta_dot_3*sin(theta2 + theta3 + theta4 + theta5) + 0.5*a2*lc5_2*m5*theta_dot_4*sin(theta2 + theta3 + theta4 + theta5) + 0.5*a2*lc5_2*m5*theta_dot_5*sin(theta2 + theta3 + theta4 + theta5) + 0.25*a5*lc5_3*m5*theta_dot_3*sin(theta2 + theta3 + theta4 + theta5) + 0.25*a5*lc5_3*m5*theta_dot_4*sin(theta2 + theta3 + theta4 + theta5) + 0.25*a5*lc5_3*m5*theta_dot_5*sin(theta2 + theta3 + theta4 + theta5) + 0.5*a2*lc3_1*m3*theta_dot_1*cos(2.0*theta2 - theta3) + 0.25*a3*lc4_2*m4*theta_dot_1*cos(2.0*theta2 - theta4) - 0.25*a4*lc5_1*m5*theta_dot_1*cos(2.0*theta2 - theta5) + 0.5*a1*lc3_2*m3*theta_dot_1*cos(theta2 + theta3) + 0.5*a2*lc3_2*m3*theta_dot_3*cos(theta2 + theta3) + 0.25*a3*lc3_3*m3*theta_dot_3*cos(theta2 + theta3) - 0.5*a3*lc4_1*m4*theta_dot_3*cos(theta2 + theta4) - 0.25*a3*lc4_1*m4*theta_dot_4*cos(theta2 + theta4) + 0.5*a3*lc4_3*m4*theta_dot_3*cos(theta2 + theta3) + 0.5*a3*lc5_3*m5*theta_dot_3*cos(theta2 + theta3) - 0.5*a4*lc5_2*m5*theta_dot_3*cos(theta2 + theta5) - 0.5*a4*lc5_2*m5*theta_dot_4*cos(theta2 + theta5) - 0.25*a4*lc5_2*m5*theta_dot_5*cos(theta2 + theta5) - 0.125*a3*a4*m4*theta_dot_1*sin(2.0*theta2 - theta4) - 0.25*a3*a4*m5*theta_dot_1*sin(2.0*theta2 - theta4) + 0.5*lc5_1*lc5_3*m5*theta_dot_3*sin(theta2 + theta3 + theta4 + theta5) + 0.5*lc5_1*lc5_3*m5*theta_dot_4*sin(theta2 + theta3 + theta4 + theta5) + 0.5*lc5_1*lc5_3*m5*theta_dot_5*sin(theta2 + theta3 + theta4 + theta5) + 0.25*a1*a3*m3*theta_dot_1*sin(theta2 + theta3) + 0.5*a1*a3*m4*theta_dot_1*sin(theta2 + theta3) + 0.5*a1*a3*m5*theta_dot_1*sin(theta2 + theta3) + 0.25*a2*a3*m3*theta_dot_3*sin(theta2 + theta3) + 0.5*a2*a3*m4*theta_dot_3*sin(theta2 + theta3) + 0.5*a2*a3*m5*theta_dot_3*sin(theta2 + theta3) - 0.25*a4*a5*m5*theta_dot_3*sin(theta2 + theta5) - 0.25*a4*a5*m5*theta_dot_4*sin(theta2 + theta5) - 0.125*a4*a5*m5*theta_dot_5*sin(theta2 + theta5) + 0.25*a2*a4*m4*theta_dot_1*cos(theta3 - 2.0*theta2 + theta4) - 0.25*a2*a4*m4*theta_dot_1*cos(2.0*theta2 + theta3 + theta4) + 0.5*a2*a4*m5*theta_dot_1*cos(theta3 - 2.0*theta2 + theta4) - 0.5*a2*a4*m5*theta_dot_1*cos(2.0*theta2 + theta3 + theta4) + 0.25*a3*a4*m4*theta_dot_3*cos(theta2 + 2.0*theta3 + theta4) + 0.125*a3*a4*m4*theta_dot_4*cos(theta2 + 2.0*theta3 + theta4) + 0.5*a3*a4*m5*theta_dot_3*cos(theta2 + 2.0*theta3 + theta4) + 0.25*a3*a4*m5*theta_dot_4*cos(theta2 + 2.0*theta3 + theta4) - 0.125*a3*a5*m5*theta_dot_1*cos(theta4 - 2.0*theta2 + theta5) + 0.125*a3*a5*m5*theta_dot_1*cos(2.0*theta2 + theta4 + theta5) + 0.5*lc3_2*lc3_3*m3*theta_dot_1*cos(2.0*theta2 - theta3) + 0.5*lc3_1*lc3_3*m3*theta_dot_3*cos(theta2 + theta3) + 0.5*a2*lc3_2*m3*theta_dot_1*sin(2.0*theta2 - theta3) - 0.25*a3*lc3_3*m3*theta_dot_1*sin(2.0*theta2 - theta3) - 0.25*a3*lc4_1*m4*theta_dot_1*sin(2.0*theta2 - theta4) - 0.5*a3*lc4_3*m4*theta_dot_1*sin(2.0*theta2 - theta3) - 0.5*a3*lc5_3*m5*theta_dot_1*sin(2.0*theta2 - theta3) - 0.25*a4*lc5_2*m5*theta_dot_1*sin(2.0*theta2 - theta5) + 0.5*a1*lc3_1*m3*theta_dot_1*sin(theta2 + theta3) + 0.5*a2*lc3_1*m3*theta_dot_3*sin(theta2 + theta3) + 0.5*a3*lc4_2*m4*theta_dot_3*sin(theta2 + theta4) + 0.25*a3*lc4_2*m4*theta_dot_4*sin(theta2 + theta4) - 0.5*a4*lc5_1*m5*theta_dot_3*sin(theta2 + theta5) - 0.5*a4*lc5_1*m5*theta_dot_4*sin(theta2 + theta5) - 0.25*a4*lc5_1*m5*theta_dot_5*sin(theta2 + theta5) + 0.25*a4*lc4_1*m4*theta_dot_3*cos(2.0*theta3 - theta2 + 2.0*theta4) + 0.25*a4*lc4_1*m4*theta_dot_4*cos(2.0*theta3 - theta2 + 2.0*theta4) + 0.5*a2*lc4_1*m4*theta_dot_1*cos(theta3 - 2.0*theta2 + theta4) - 0.5*a2*lc4_1*m4*theta_dot_1*cos(2.0*theta2 + theta3 + theta4) + 0.5*a3*lc4_1*m4*theta_dot_3*cos(theta2 + 2.0*theta3 + theta4) + 0.25*a3*lc4_1*m4*theta_dot_4*cos(theta2 + 2.0*theta3 + theta4) - 0.25*a3*lc5_1*m5*theta_dot_1*cos(theta4 - 2.0*theta2 + theta5) + 0.25*a3*lc5_1*m5*theta_dot_1*cos(2.0*theta2 + theta4 + theta5) - 0.5*lc3_1*lc3_3*m3*theta_dot_1*sin(2.0*theta2 - theta3) - 0.5*lc3_2*lc3_3*m3*theta_dot_3*sin(theta2 + theta3) + 0.125*a3*a5*m5*theta_dot_1*cos(2.0*theta3 - 2.0*theta2 + theta4 + theta5) - 0.125*a3*a5*m5*theta_dot_1*cos(2.0*theta2 + 2.0*theta3 + theta4 + theta5) + 0.5*lc4_2*lc4_3*m4*theta_dot_1*cos(theta3 - 2.0*theta2 + theta4) + 0.5*lc4_2*lc4_3*m4*theta_dot_1*cos(2.0*theta2 + theta3 + theta4) - 0.5*a1*a2*m2*theta_dot_1*cos(theta2) - 1.0*a1*a2*m3*theta_dot_1*cos(theta2) - 1.0*a1*a2*m4*theta_dot_1*cos(theta2) - 1.0*a1*a2*m5*theta_dot_1*cos(theta2) - 0.25*a4*lc4_2*m4*theta_dot_3*sin(2.0*theta3 - theta2 + 2.0*theta4) - 0.25*a4*lc4_2*m4*theta_dot_4*sin(2.0*theta3 - theta2 + 2.0*theta4) - 0.5*a2*lc4_2*m4*theta_dot_1*sin(theta3 - 2.0*theta2 + theta4) + 0.5*a2*lc4_2*m4*theta_dot_1*sin(2.0*theta2 + theta3 + theta4) - 0.5*a3*lc4_2*m4*theta_dot_3*sin(theta2 + 2.0*theta3 + theta4) + 0.25*a4*lc4_3*m4*theta_dot_1*sin(theta3 - 2.0*theta2 + theta4) + 0.25*a4*lc4_3*m4*theta_dot_1*sin(2.0*theta2 + theta3 + theta4) - 0.25*a3*lc4_2*m4*theta_dot_4*sin(theta2 + 2.0*theta3 + theta4) + 0.25*a3*lc5_2*m5*theta_dot_1*sin(theta4 - 2.0*theta2 + theta5) - 0.25*a3*lc5_2*m5*theta_dot_1*sin(2.0*theta2 + theta4 + theta5) + 0.5*a4*lc5_3*m5*theta_dot_1*sin(theta3 - 2.0*theta2 + theta4) + 0.5*a4*lc5_3*m5*theta_dot_1*sin(2.0*theta2 + theta3 + theta4) - 0.25*a5*lc5_1*m5*theta_dot_3*cos(2.0*theta3 - theta2 + 2.0*theta4 + 2.0*theta5) - 0.25*a5*lc5_1*m5*theta_dot_4*cos(2.0*theta3 - theta2 + 2.0*theta4 + 2.0*theta5) - 0.25*a5*lc5_1*m5*theta_dot_5*cos(2.0*theta3 - theta2 + 2.0*theta4 + 2.0*theta5) + 0.25*a3*lc5_1*m5*theta_dot_1*cos(2.0*theta3 - 2.0*theta2 + theta4 + theta5) - 0.25*a3*lc5_1*m5*theta_dot_1*cos(2.0*theta2 + 2.0*theta3 + theta4 + theta5) + 0.5*a4*lc5_2*m5*theta_dot_3*cos(theta2 + 2.0*theta3 + 2.0*theta4 + theta5) + 0.5*a4*lc5_2*m5*theta_dot_4*cos(theta2 + 2.0*theta3 + 2.0*theta4 + theta5) + 0.25*a4*lc5_2*m5*theta_dot_5*cos(theta2 + 2.0*theta3 + 2.0*theta4 + theta5) - 1.0*a1*lc2_1*m2*theta_dot_1*cos(theta2) - 0.5*a3*lc3_1*m3*theta_dot_3*cos(theta2) - 0.5*a4*lc4_1*m4*theta_dot_3*cos(theta2) - 0.5*a4*lc4_1*m4*theta_dot_4*cos(theta2) - 0.5*a5*lc5_1*m5*theta_dot_3*cos(theta2) - 0.5*a5*lc5_1*m5*theta_dot_4*cos(theta2) - 0.5*a5*lc5_1*m5*theta_dot_5*cos(theta2) + 0.25*a4*a5*m5*theta_dot_3*sin(theta2 + 2.0*theta3 + 2.0*theta4 + theta5) + 0.25*a4*a5*m5*theta_dot_4*sin(theta2 + 2.0*theta3 + 2.0*theta4 + theta5) + 0.125*a4*a5*m5*theta_dot_5*sin(theta2 + 2.0*theta3 + 2.0*theta4 + theta5) - 0.5*lc4_1*lc4_2*m4*theta_dot_3*sin(2.0*theta3 - theta2 + 2.0*theta4) - 0.5*lc4_1*lc4_2*m4*theta_dot_4*sin(2.0*theta3 - theta2 + 2.0*theta4) + 0.5*lc4_1*lc4_3*m4*theta_dot_1*sin(theta3 - 2.0*theta2 + theta4) + 0.5*lc4_1*lc4_3*m4*theta_dot_1*sin(2.0*theta2 + theta3 + theta4) + 0.25*a5*lc5_2*m5*theta_dot_3*sin(2.0*theta3 - theta2 + 2.0*theta4 + 2.0*theta5) + 0.25*a5*lc5_2*m5*theta_dot_4*sin(2.0*theta3 - theta2 + 2.0*theta4 + 2.0*theta5) + 0.25*a5*lc5_2*m5*theta_dot_5*sin(2.0*theta3 - theta2 + 2.0*theta4 + 2.0*theta5) - 0.25*a3*lc5_2*m5*theta_dot_1*sin(2.0*theta3 - 2.0*theta2 + theta4 + theta5) + 0.25*a3*lc5_2*m5*theta_dot_1*sin(2.0*theta2 + 2.0*theta3 + theta4 + theta5) + 0.5*a4*lc5_1*m5*theta_dot_3*sin(theta2 + 2.0*theta3 + 2.0*theta4 + theta5) + 0.5*a4*lc5_1*m5*theta_dot_4*sin(theta2 + 2.0*theta3 + 2.0*theta4 + theta5) + 0.25*a4*lc5_1*m5*theta_dot_5*sin(theta2 + 2.0*theta3 + 2.0*theta4 + theta5) + 1.0*a1*lc2_3*m2*theta_dot_1*sin(theta2) + 1.0*a1*lc3_3*m3*theta_dot_1*sin(theta2) + 1.0*a1*lc4_3*m4*theta_dot_1*sin(theta2) + 1.0*a1*lc5_3*m5*theta_dot_1*sin(theta2) - 0.25*a1*a5*m5*theta_dot_1*cos(theta3 - theta2 + theta4 + theta5) - 0.25*a2*a5*m5*theta_dot_3*cos(theta3 - theta2 + theta4 + theta5) - 0.25*a2*a5*m5*theta_dot_4*cos(theta3 - theta2 + theta4 + theta5) - 0.25*a2*a5*m5*theta_dot_5*cos(theta3 - theta2 + theta4 + theta5) - 0.125*a3*lc3_2*m3*theta_dot_1*cos(2.0*theta2 - 2.0*theta3) + 0.125*a3*lc3_2*m3*theta_dot_1*cos(2.0*theta2 + 2.0*theta3) + 0.5*lc5_1*lc5_2*m5*theta_dot_3*sin(2.0*theta3 - theta2 + 2.0*theta4 + 2.0*theta5) + 0.5*lc5_1*lc5_2*m5*theta_dot_4*sin(2.0*theta3 - theta2 + 2.0*theta4 + 2.0*theta5) + 0.5*lc5_1*lc5_2*m5*theta_dot_5*sin(2.0*theta3 - theta2 + 2.0*theta4 + 2.0*theta5)
C21 = C21a + C21b
C22 = I_xy_5*theta_dot_3*cos(2*theta3 + 2*theta4 + 2*theta5) + I_xy_5*theta_dot_4*cos(2*theta3 + 2*theta4 + 2*theta5) + I_xy_5*theta_dot_5*cos(2*theta3 + 2*theta4 + 2*theta5) + 0.5*I_xx_5*theta_dot_3*sin(2*theta3 + 2*theta4 + 2*theta5) + 0.5*I_xx_5*theta_dot_4*sin(2*theta3 + 2*theta4 + 2*theta5) + 0.5*I_xx_5*theta_dot_5*sin(2*theta3 + 2*theta4 + 2*theta5) - 0.5*I_yy_5*theta_dot_3*sin(2*theta3 + 2*theta4 + 2*theta5) - 0.5*I_yy_5*theta_dot_4*sin(2*theta3 + 2*theta4 + 2*theta5) - 0.5*I_yy_5*theta_dot_5*sin(2*theta3 + 2*theta4 + 2*theta5) - 1.0*I_xy_4*theta_dot_3*cos(2*theta3 + 2*theta4) - 1.0*I_xy_4*theta_dot_4*cos(2*theta3 + 2*theta4) - 1.0*I_xy_3*theta_dot_3*cos(2.0*theta3) - 0.5*I_xx_4*theta_dot_3*sin(2*theta3 + 2*theta4) - 0.5*I_xx_4*theta_dot_4*sin(2*theta3 + 2*theta4) + 0.5*I_yy_4*theta_dot_3*sin(2*theta3 + 2*theta4) + 0.5*I_yy_4*theta_dot_4*sin(2*theta3 + 2*theta4) - 0.5*I_xx_3*theta_dot_3*sin(2.0*theta3) + 0.5*I_yy_3*theta_dot_3*sin(2.0*theta3) - 0.125*a5^2*m5*theta_dot_3*sin(2*theta3 + 2*theta4 + 2*theta5) - 0.125*a5^2*m5*theta_dot_4*sin(2*theta3 + 2*theta4 + 2*theta5) - 0.125*a5^2*m5*theta_dot_5*sin(2*theta3 + 2*theta4 + 2*theta5) - 0.5*lc5_1^2*m5*theta_dot_3*sin(2*theta3 + 2*theta4 + 2*theta5) - 0.5*lc5_1^2*m5*theta_dot_4*sin(2*theta3 + 2*theta4 + 2*theta5) + 0.5*lc5_2^2*m5*theta_dot_3*sin(2*theta3 + 2*theta4 + 2*theta5) - 0.5*lc5_1^2*m5*theta_dot_5*sin(2*theta3 + 2*theta4 + 2*theta5) + 0.5*lc5_2^2*m5*theta_dot_4*sin(2*theta3 + 2*theta4 + 2*theta5) + 0.5*lc5_2^2*m5*theta_dot_5*sin(2*theta3 + 2*theta4 + 2*theta5) + 0.125*a4^2*m4*theta_dot_3*sin(2*theta3 + 2*theta4) + 0.125*a4^2*m4*theta_dot_4*sin(2*theta3 + 2*theta4) + 0.5*a4^2*m5*theta_dot_3*sin(2*theta3 + 2*theta4) + 0.5*a4^2*m5*theta_dot_4*sin(2*theta3 + 2*theta4) + 0.5*lc4_1^2*m4*theta_dot_3*sin(2*theta3 + 2*theta4) + 0.5*lc4_1^2*m4*theta_dot_4*sin(2*theta3 + 2*theta4) - 0.5*lc4_2^2*m4*theta_dot_3*sin(2*theta3 + 2*theta4) - 0.5*lc4_2^2*m4*theta_dot_4*sin(2*theta3 + 2*theta4) + 0.125*a3^2*m3*theta_dot_3*sin(2.0*theta3) + 0.5*a3^2*m4*theta_dot_3*sin(2.0*theta3) + 0.5*a3^2*m5*theta_dot_3*sin(2.0*theta3) + 0.5*lc3_1^2*m3*theta_dot_3*sin(2.0*theta3) - 0.5*lc3_2^2*m3*theta_dot_3*sin(2.0*theta3) - 1.0*a2*lc5_2*m5*theta_dot_3*cos(theta3 + theta4 + theta5) - 1.0*a2*lc5_2*m5*theta_dot_4*cos(theta3 + theta4 + theta5) - 1.0*a2*lc5_2*m5*theta_dot_5*cos(theta3 + theta4 + theta5) - 0.5*a2*a5*m5*theta_dot_3*sin(theta3 + theta4 + theta5) - 0.5*a2*a5*m5*theta_dot_4*sin(theta3 + theta4 + theta5) - 0.5*a2*a5*m5*theta_dot_5*sin(theta3 + theta4 + theta5) - 1.0*a2*lc5_1*m5*theta_dot_3*sin(theta3 + theta4 + theta5) - 1.0*a2*lc5_1*m5*theta_dot_4*sin(theta3 + theta4 + theta5) - 1.0*a2*lc5_1*m5*theta_dot_5*sin(theta3 + theta4 + theta5) - 0.5*a5*lc5_2*m5*theta_dot_3*cos(2*theta3 + 2*theta4 + 2*theta5) - 0.5*a5*lc5_2*m5*theta_dot_4*cos(2*theta3 + 2*theta4 + 2*theta5) - 0.5*a5*lc5_2*m5*theta_dot_5*cos(2*theta3 + 2*theta4 + 2*theta5) - 1.0*lc5_1*lc5_2*m5*theta_dot_3*cos(2*theta3 + 2*theta4 + 2*theta5) - 1.0*lc5_1*lc5_2*m5*theta_dot_4*cos(2*theta3 + 2*theta4 + 2*theta5) - 1.0*lc5_1*lc5_2*m5*theta_dot_5*cos(2*theta3 + 2*theta4 + 2*theta5) + a3*lc4_2*m4*theta_dot_3*cos(2.0*theta3 + theta4) + 0.5*a3*lc4_2*m4*theta_dot_4*cos(2.0*theta3 + theta4) - 0.5*a5*lc5_1*m5*theta_dot_3*sin(2*theta3 + 2*theta4 + 2*theta5) - 0.5*a5*lc5_1*m5*theta_dot_4*sin(2*theta3 + 2*theta4 + 2*theta5) - 0.5*a5*lc5_1*m5*theta_dot_5*sin(2*theta3 + 2*theta4 + 2*theta5) + 0.5*a3*a4*m4*theta_dot_3*sin(2.0*theta3 + theta4) + 0.25*a3*a4*m4*theta_dot_4*sin(2.0*theta3 + theta4) + a3*a4*m5*theta_dot_3*sin(2.0*theta3 + theta4) + 0.5*a3*a4*m5*theta_dot_4*sin(2.0*theta3 + theta4) - 0.5*a4*a5*m5*theta_dot_3*cos(2.0*theta3 + 2.0*theta4 + theta5) - 0.5*a4*a5*m5*theta_dot_4*cos(2.0*theta3 + 2.0*theta4 + theta5) - 0.25*a4*a5*m5*theta_dot_5*cos(2.0*theta3 + 2.0*theta4 + theta5) + a3*lc4_1*m4*theta_dot_3*sin(2.0*theta3 + theta4) + 0.5*a3*lc4_1*m4*theta_dot_4*sin(2.0*theta3 + theta4) - 1.0*a4*lc5_1*m5*theta_dot_3*cos(2.0*theta3 + 2.0*theta4 + theta5) - 1.0*a4*lc5_1*m5*theta_dot_4*cos(2.0*theta3 + 2.0*theta4 + theta5) - 0.5*a4*lc5_1*m5*theta_dot_5*cos(2.0*theta3 + 2.0*theta4 + theta5) + 0.5*a4*lc4_2*m4*theta_dot_3*cos(2*theta3 + 2*theta4) + 0.5*a4*lc4_2*m4*theta_dot_4*cos(2*theta3 + 2*theta4) + a4*lc5_2*m5*theta_dot_3*sin(2.0*theta3 + 2.0*theta4 + theta5) + a4*lc5_2*m5*theta_dot_4*sin(2.0*theta3 + 2.0*theta4 + theta5) + 0.5*a4*lc5_2*m5*theta_dot_5*sin(2.0*theta3 + 2.0*theta4 + theta5) + lc4_1*lc4_2*m4*theta_dot_3*cos(2*theta3 + 2*theta4) + lc4_1*lc4_2*m4*theta_dot_4*cos(2*theta3 + 2*theta4) + 0.5*a3*lc3_2*m3*theta_dot_3*cos(2.0*theta3) + 0.5*a4*lc4_1*m4*theta_dot_3*sin(2*theta3 + 2*theta4) + 0.5*a4*lc4_1*m4*theta_dot_4*sin(2*theta3 + 2*theta4) + lc3_1*lc3_2*m3*theta_dot_3*cos(2.0*theta3) + 0.5*a3*lc3_1*m3*theta_dot_3*sin(2.0*theta3) - 0.5*a2*a4*m4*theta_dot_3*cos(theta3 + theta4) - 0.5*a2*a4*m4*theta_dot_4*cos(theta3 + theta4) - 1.0*a2*a4*m5*theta_dot_3*cos(theta3 + theta4) - 1.0*a2*a4*m5*theta_dot_4*cos(theta3 + theta4) + 0.25*a3*a5*m5*theta_dot_4*cos(theta4 + theta5) + 0.25*a3*a5*m5*theta_dot_5*cos(theta4 + theta5) - 1.0*a2*lc4_1*m4*theta_dot_3*cos(theta3 + theta4) - 1.0*a2*lc4_1*m4*theta_dot_4*cos(theta3 + theta4) + 0.5*a3*lc5_1*m5*theta_dot_4*cos(theta4 + theta5) + 0.5*a3*lc5_1*m5*theta_dot_5*cos(theta4 + theta5) - 0.5*a3*a5*m5*theta_dot_3*cos(2.0*theta3 + theta4 + theta5) - 0.25*a3*a5*m5*theta_dot_4*cos(2.0*theta3 + theta4 + theta5) - 0.25*a3*a5*m5*theta_dot_5*cos(2.0*theta3 + theta4 + theta5) + a2*lc4_2*m4*theta_dot_3*sin(theta3 + theta4) + a2*lc4_2*m4*theta_dot_4*sin(theta3 + theta4) - 0.5*a3*lc5_2*m5*theta_dot_4*sin(theta4 + theta5) - 0.5*a3*lc5_2*m5*theta_dot_5*sin(theta4 + theta5) - 1.0*a3*lc5_1*m5*theta_dot_3*cos(2.0*theta3 + theta4 + theta5) - 0.5*a3*lc5_1*m5*theta_dot_4*cos(2.0*theta3 + theta4 + theta5) - 0.5*a3*lc5_1*m5*theta_dot_5*cos(2.0*theta3 + theta4 + theta5) - 0.5*a2*a3*m3*theta_dot_3*cos(theta3) - 1.0*a2*a3*m4*theta_dot_3*cos(theta3) - 1.0*a2*a3*m5*theta_dot_3*cos(theta3) + 0.25*a4*a5*m5*theta_dot_5*cos(theta5) + a3*lc5_2*m5*theta_dot_3*sin(2.0*theta3 + theta4 + theta5) + 0.5*a3*lc5_2*m5*theta_dot_4*sin(2.0*theta3 + theta4 + theta5) + 0.5*a3*lc5_2*m5*theta_dot_5*sin(2.0*theta3 + theta4 + theta5) - 1.0*a2*lc3_1*m3*theta_dot_3*cos(theta3) - 0.5*a3*lc4_2*m4*theta_dot_4*cos(theta4) + 0.5*a4*lc5_1*m5*theta_dot_5*cos(theta5) - 0.25*a3*a4*m4*theta_dot_4*sin(theta4) - 0.5*a3*a4*m5*theta_dot_4*sin(theta4) + a2*lc3_2*m3*theta_dot_3*sin(theta3) - 0.5*a3*lc4_1*m4*theta_dot_4*sin(theta4) - 0.5*a4*lc5_2*m5*theta_dot_5*sin(theta5)
